simulink model "CONTROL_01"  (R2018b)
(part 101 of 185)

[(de6*((I6xy*(cos(e2)*cos(e3)*sin(e4)*sin(e6) + cos(e2)*cos(e6)*sin(e3)*sin(e5) + cos(e3)*cos(e6)*sin(e2)*sin(e5) - sin(e2)*sin(e3)*sin(e4)*sin(e6) - cos(e2)*cos(e3)*cos(e4)*cos(e5)*cos(e6) + cos(e4)*cos(e5)*cos(e6)*sin(e2)*sin(e3)) + I6yy*(cos(e6)*sin(e2)*sin(e3)*sin(e4) - cos(e2)*cos(e3)*cos(e6)*sin(e4) + cos(e2)*sin(e3)*sin(e5)*sin(e6) + cos(e3)*sin(e2)*sin(e5)*sin(e6) - cos(e2)*cos(e3)*cos(e4)*cos(e5)*sin(e6) + cos(e4)*cos(e5)*sin(e2)*sin(e3)*sin(e6)) + I6yz*(cos(e2)*cos(e5)*sin(e3) + cos(e3)*cos(e5)*sin(e2) + cos(e2)*cos(e3)*cos(e4)*sin(e5) - cos(e4)*sin(e2)*sin(e3)*sin(e5)))*(cos(e2)*cos(e3)*sin(e4)*sin(e6) + cos(e2)*cos(e6)*sin(e3)*sin(e5) + cos(e3)*cos(e6)*sin(e2)*sin(e5) - sin(e2)*sin(e3)*sin(e4)*sin(e6) - cos(e2)*cos(e3)*cos(e4)*cos(e5)*cos(e6) + cos(e4)*cos(e5)*cos(e6)*sin(e2)*sin(e3)) - (I6xx*(cos(e2)*cos(e3)*sin(e4)*sin(e6) + cos(e2)*cos(e6)*sin(e3)*sin(e5) + cos(e3)*cos(e6)*sin(e2)*sin(e5) - sin(e2)*sin(e3)*sin(e4)*sin(e6) - cos(e2)*cos(e3)*cos(e4)*cos(e5)*cos(e6) + cos(e4)*cos(e5)*cos(e6)*sin(e2)*sin(e3)) + I6xy*(cos(e6)*sin(e2)*sin(e3)*sin(e4) - cos(e2)*cos(e3)*cos(e6)*sin(e4) + cos(e2)*sin(e3)*sin(e5)*sin(e6) + cos(e3)*sin(e2)*sin(e5)*sin(e6) - cos(e2)*cos(e3)*cos(e4)*cos(e5)*sin(e6) + cos(e4)*cos(e5)*sin(e2)*sin(e3)*sin(e6)) - I6zx*(cos(e2)*cos(e5)*sin(e3) + cos(e3)*cos(e5)*sin(e2) + cos(e2)*cos(e3)*cos(e4)*sin(e5) - cos(e4)*sin(e2)*sin(e3)*sin(e5)))*(cos(e6)*sin(e2)*sin(e3)*sin(e4) - cos(e2)*cos(e3)*cos(e6)*sin(e4) + cos(e2)*sin(e3)*sin(e5)*sin(e6) + cos(e3)*sin(e2)*sin(e5)*sin(e6) - cos(e2)*cos(e3)*cos(e4)*cos(e5)*sin(e6) + cos(e4)*cos(e5)*sin(e2)*sin(e3)*sin(e6)) + (I6xy*(cos(e2)*cos(e3)*sin(e4)*sin(e6) + cos(e2)*cos(e6)*sin(e3)*sin(e5) + cos(e3)*cos(e6)*sin(e2)*sin(e5) - sin(e2)*sin(e3)*sin(e4)*sin(e6) - cos(e2)*cos(e3)*cos(e4)*cos(e5)*cos(e6) + cos(e4)*cos(e5)*cos(e6)*sin(e2)*sin(e3)) - I6xx*(cos(e6)*sin(e2)*sin(e3)*sin(e4) - cos(e2)*cos(e3)*cos(e6)*sin(e4) + cos(e2)*sin(e3)*sin(e5)*sin(e6) + cos(e3)*sin(e2)*sin(e5)*sin(e6) - cos(e2)*cos(e3)*cos(e4)*cos(e5)*sin(e6) + cos(e4)*cos(e5)*sin(e2)*sin(e3)*sin(e6)))*(cos(e2)*cos(e3)*sin(e4)*sin(e6) + cos(e2)*cos(e6)*sin(e3)*sin(e5) + cos(e3)*cos(e6)*sin(e2)*sin(e5) - sin(e2)*sin(e3)*sin(e4)*sin(e6) - cos(e2)*cos(e3)*cos(e4)*cos(e5)*cos(e6) + cos(e4)*cos(e5)*cos(e6)*sin(e2)*sin(e3)) + (I6yy*(cos(e2)*cos(e3)*sin(e4)*sin(e6) + cos(e2)*cos(e6)*sin(e3)*sin(e5) + cos(e3)*cos(e6)*sin(e2)*sin(e5) - sin(e2)*sin(e3)*sin(e4)*sin(e6) - cos(e2)*cos(e3)*cos(e4)*cos(e5)*cos(e6) + cos(e4)*cos(e5)*cos(e6)*sin(e2)*sin(e3)) - I6xy*(cos(e6)*sin(e2)*sin(e3)*sin(e4) - cos(e2)*cos(e3)*cos(e6)*sin(e4) + cos(e2)*sin(e3)*sin(e5)*sin(e6) + cos(e3)*sin(e2)*sin(e5)*sin(e6) - cos(e2)*cos(e3)*cos(e4)*cos(e5)*sin(e6) + cos(e4)*cos(e5)*sin(e2)*sin(e3)*sin(e6)))*(cos(e6)*sin(e2)*sin(e3)*sin(e4) - cos(e2)*cos(e3)*cos(e6)*sin(e4) + cos(e2)*sin(e3)*sin(e5)*sin(e6) + cos(e3)*sin(e2)*sin(e5)*sin(e6) - cos(e2)*cos(e3)*cos(e4)*cos(e5)*sin(e6) + cos(e4)*cos(e5)*sin(e2)*sin(e3)*sin(e6)) + (I6yz*(cos(e2)*cos(e3)*sin(e4)*sin(e6) + cos(e2)*cos(e6)*sin(e3)*sin(e5) + cos(e3)*cos(e6)*sin(e2)*sin(e5) - sin(e2)*sin(e3)*sin(e4)*sin(e6) - cos(e2)*cos(e3)*cos(e4)*cos(e5)*cos(e6) + cos(e4)*cos(e5)*cos(e6)*sin(e2)*sin(e3)) + I6zx*(cos(e6)*sin(e2)*sin(e3)*sin(e4) - cos(e2)*cos(e3)*cos(e6)*sin(e4) + cos(e2)*sin(e3)*sin(e5)*sin(e6) + cos(e3)*sin(e2)*sin(e5)*sin(e6) - cos(e2)*cos(e3)*cos(e4)*cos(e5)*sin(e6) + cos(e4)*cos(e5)*sin(e2)*sin(e3)*sin(e6)))*(cos(e2)*cos(e5)*sin(e3) + cos(e3)*cos(e5)*sin(e2) + cos(e2)*cos(e3)*cos(e4)*sin(e5) - cos(e4)*sin(e2)*sin(e3)*sin(e5)) + 2*m6*(x6*(cos(e6)*(cos(e4)*sin(e1) - sin(e2 + e3)*cos(e1)*sin(e4)) - sin(e6)*(cos(e5)*(sin(e1)*sin(e4) + sin(e2 + e3)*cos(e1)*cos(e4)) + cos(e2 + e3)*cos(e1)*sin(e5))) - y6*(sin(e6)*(cos(e4)*sin(e1) - sin(e2 + e3)*cos(e1)*sin(e4)) + cos(e6)*(cos(e5)*(sin(e1)*sin(e4) + sin(e2 + e3)*cos(e1)*cos(e4)) + cos(e2 + e3)*cos(e1)*sin(e5))))*(cos(e1)*(a1 + d4*cos(e2 + e3) + a3*sin(e2 + e3) + a2*sin(e2)) + x6*(sin(e6)*(cos(e4)*sin(e1) - sin(e2 + e3)*cos(e1)*sin(e4)) + cos(e6)*(cos(e5)*(sin(e1)*sin(e4) + sin(e2 + e3)*cos(e1)*cos(e4)) + cos(e2 + e3)*cos(e1)*sin(e5))) + y6*(cos(e6)*(cos(e4)*sin(e1) - sin(e2 + e3)*cos(e1)*sin(e4)) - sin(e6)*(cos(e5)*(sin(e1)*sin(e4) + sin(e2 + e3)*cos(e1)*cos(e4)) + cos(e2 + e3)*cos(e1)*sin(e5))) - z6*(sin(e5)*(sin(e1)*sin(e4) + sin(e2 + e3)*cos(e1)*cos(e4)) - cos(e2 + e3)*cos(e1)*cos(e5))) - 2*m6*(x6*(cos(e6)*(cos(e1)*cos(e4) + sin(e2 + e3)*sin(e1)*sin(e4)) - sin(e6)*(cos(e5)*(cos(e1)*sin(e4) - sin(e2 + e3)*cos(e4)*sin(e1)) - cos(e2 + e3)*sin(e1)*sin(e5))) - y6*(sin(e6)*(cos(e1)*cos(e4) + sin(e2 + e3)*sin(e1)*sin(e4)) + cos(e6)*(cos(e5)*(cos(e1)*sin(e4) - sin(e2 + e3)*cos(e4)*sin(e1)) - cos(e2 + e3)*sin(e1)*sin(e5))))*(sin(e1)*(a1 + d4*cos(e2 + e3) + a3*sin(e2 + e3) + a2*sin(e2)) - x6*(sin(e6)*(cos(e1)*cos(e4) + sin(e2 + e3)*sin(e1)*sin(e4)) + cos(e6)*(cos(e5)*(cos(e1)*sin(e4) - sin(e2 + e3)*cos(e4)*sin(e1)) - cos(e2 + e3)*sin(e1)*sin(e5))) - y6*(cos(e6)*(cos(e1)*cos(e4) + sin(e2 + e3)*sin(e1)*sin(e4)) - sin(e6)*(cos(e5)*(cos(e1)*sin(e4) - sin(e2 + e3)*cos(e4)*sin(e1)) - cos(e2 + e3)*sin(e1)*sin(e5))) + z6*(sin(e5)*(cos(e1)*sin(e4) - sin(e2 + e3)*cos(e4)*sin(e1)) + cos(e2 + e3)*cos(e5)*sin(e1)))))/2 + (de3*((I6xx*(cos(e2)*cos(e3)*cos(e6)*sin(e5) - cos(e2)*sin(e3)*sin(e4)*sin(e6) - cos(e3)*sin(e2)*sin(e4)*sin(e6) - cos(e6)*sin(e2)*sin(e3)*sin(e5) + cos(e2)*cos(e4)*cos(e5)*cos(e6)*sin(e3) + cos(e3)*cos(e4)*cos(e5)*cos(e6)*sin(e2)) + I6xy*(cos(e2)*cos(e6)*sin(e3)*sin(e4) + cos(e3)*cos(e6)*sin(e2)*sin(e4) + cos(e2)*cos(e3)*sin(e5)*sin(e6) - sin(e2)*sin(e3)*sin(e5)*sin(e6) + cos(e2)*cos(e4)*cos(e5)*sin(e3)*sin(e6) + cos(e3)*cos(e4)*cos(e5)*sin(e2)*sin(e6)) + I6zx*(cos(e5)*sin(e2)*sin(e3) - cos(e2)*cos(e3)*cos(e5) + cos(e2)*cos(e4)*sin(e3)*sin(e5) + cos(e3)*cos(e4)*sin(e2)*sin(e5)))*(cos(e2)*cos(e3)*sin(e4)*sin(e6) + cos(e2)*cos(e6)*sin(e3)*sin(e5) + cos(e3)*cos(e6)*sin(e2)*sin(e5) - sin(e2)*sin(e3)*sin(e4)*sin(e6) - cos(e2)*cos(e3)*cos(e4)*cos(e5)*cos(e6) + cos(e4)*cos(e5)*cos(e6)*sin(e2)*sin(e3)) + (I6xx*(cos(e2)*cos(e3)*sin(e4)*sin(e6) + cos(e2)*cos(e6)*sin(e3)*sin(e5) + cos(e3)*cos(e6)*sin(e2)*sin(e5) - sin(e2)*sin(e3)*sin(e4)*sin(e6) - cos(e2)*cos(e3)*cos(e4)*cos(e5)*cos(e6) + cos(e4)*cos(e5)*cos(e6)*sin(e2)*sin(e3)) + I6xy*(cos(e6)*sin(e2)*sin(e3)*sin(e4) - cos(e2)*cos(e3)*cos(e6)*sin(e4) + cos(e2)*sin(e3)*sin(e5)*sin(e6) + cos(e3)*sin(e2)*sin(e5)*sin(e6) - cos(e2)*cos(e3)*cos(e4)*cos(e5)*sin(e6) + cos(e4)*cos(e5)*sin(e2)*sin(e3)*sin(e6)) - I6zx*(cos(e2)*cos(e5)*sin(e3) + cos(e3)*cos(e5)*sin(e2) + cos(e2)*cos(e3)*cos(e4)*sin(e5) - cos(e4)*sin(e2)*sin(e3)*sin(e5)))*(cos(e2)*cos(e3)*cos(e6)*sin(e5) - cos(e2)*sin(e3)*sin(e4)*sin(e6) - cos(e3)*sin(e2)*sin(e4)*sin(e6) - cos(e6)*sin(e2)*sin(e3)*sin(e5) + cos(e2)*cos(e4)*cos(e5)*cos(e6)*sin(e3) + cos(e3)*cos(e4)*cos(e5)*cos(e6)*sin(e2)) - (cos(e2)*cos(e3)*cos(e4) - cos(e4)*sin(e2)*sin(e3))*(I4xx*(cos(e2)*cos(e4)*sin(e3) + cos(e3)*cos(e4)*sin(e2)) - I4zx*cos(e2 + e3) + I4xy*(cos(e2)*sin(e3)*sin(e4) + cos(e3)*sin(e2)*sin(e4))) - (cos(e2)*sin(e3)*sin(e4) + cos(e3)*sin(e2)*sin(e4))*(I5zz*(cos(e2)*cos(e3)*sin(e4) - sin(e2)*sin(e3)*sin(e4)) + I5yz*(cos(e2)*cos(e5)*sin(e3) + cos(e3)*cos(e5)*sin(e2) + cos(e2)*cos(e3)*cos(e4)*sin(e5) - cos(e4)*sin(e2)*sin(e3)*sin(e5)) + I5zx*(cos(e2)*sin(e3)*sin(e5) + cos(e3)*sin(e2)*sin(e5) - cos(e2)*cos(e3)*cos(e4)*cos(e5) + cos(e4)*cos(e5)*sin(e2)*sin(e3))) - (cos(e2)*cos(e3)*sin(e4) - sin(e2)*sin(e3)*sin(e4))*(I5zz*(cos(e2)*sin(e3)*sin(e4) + cos(e3)*sin(e2)*sin(e4)) + I5yz*(cos(e5)*sin(e2)*sin(e3) - cos(e2)*cos(e3)*cos(e5) + cos(e2)*cos(e4)*sin(e3)*sin(e5) + cos(e3)*cos(e4)*sin(e2)*sin(e5)) - I5zx*(cos(e2)*cos(e3)*sin(e5) - sin(e2)*sin(e3)*sin(e5) + cos(e2)*cos(e4)*cos(e5)*sin(e3) + cos(e3)*cos(e4)*cos(e5)*sin(e2))) - (cos(e2)*cos(e4)*sin(e3) + cos(e3)*cos(e4)*sin(e2))*(I4zx*sin(e2 + e3) + I4xx*(cos(e2)*cos(e3)*cos(e4) - cos(e4)*sin(e2)*sin(e3)) + I4xy*(cos(e2)*cos(e3)*sin(e4) - sin(e2)*sin(e3)*sin(e4))) + (I6xy*(cos(e2)*cos(e3)*sin(e4)*sin(e6) + cos(e2)*cos(e6)*sin(e3)*sin(e5) + cos(e3)*cos(e6)*sin(e2)*sin(e5) - sin(e2)*sin(e3)*sin(e4)*sin(e6) - cos(e2)*cos(e3)*cos(e4)*cos(e5)*cos(e6) + cos(e4)*cos(e5)*cos(e6)*sin(e2)*sin(e3)) + I6yy*(cos(e6)*sin(e2)*sin(e3)*sin(e4) - cos(e2)*cos(e3)*cos(e6)*sin(e4) + cos(e2)*sin(e3)*sin(e5)*sin(e6) + cos(e3)*sin(e2)*sin(e5)*sin(e6) - cos(e2)*cos(e3)*cos(e4)*cos(e5)*sin(e6) + cos(e4)*cos(e5)*sin(e2)*sin(e3)*sin(e6)) + I6yz*(cos(e2)*cos(e5)*sin(e3) + cos(e3)*cos(e5)*sin(e2) + cos(e2)*cos(e3)*cos(e4)*sin(e5) - cos(e4)*sin(e2)*sin(e3)*sin(e5)))*(cos(e2)*cos(e6)*sin(e3)*sin(e4) + cos(e3)*cos(e6)*sin(e2)*sin(e4) + cos(e2)*cos(e3)*sin(e5)*sin(e6) - sin(e2)*sin(e3)*sin(e5)*sin(e6) + cos(e2)*cos(e4)*cos(e5)*sin(e3)*sin(e6) + cos(e3)*cos(e4)*cos(e5)*sin(e2)*sin(e6)) + (I6xy*(cos(e2)*cos(e3)*cos(e6)*sin(e5) - cos(e2)*sin(e3)*sin(e4)*sin(e6) - cos(e3)*sin(e2)*sin(e4)*sin(e6) - cos(e6)*sin(e2)*sin(e3)*sin(e5) + cos(e2)*cos(e4)*cos(e5)*cos(e6)*sin(e3) + cos(e3)*cos(e4)*cos(e5)*cos(e6)*sin(e2)) + I6yy*(cos(e2)*cos(e6)*sin(e3)*sin(e4) + cos(e3)*cos(e6)*sin(e2)*sin(e4) + cos(e2)*cos(e3)*sin(e5)*sin(e6) - sin(e2)*sin(e3)*sin(e5)*sin(e6) + cos(e2)*cos(e4)*cos(e5)*sin(e3)*sin(e6) + cos(e3)*cos(e4)*cos(e5)*sin(e2)*sin(e6)) - I6yz*(cos(e5)*sin(e2)*sin(e3) - cos(e2)*cos(e3)*cos(e5) + cos(e2)*cos(e4)*sin(e3)*sin(e5) + cos(e3)*cos(e4)*sin(e2)*sin(e5)))*(cos(e6)*sin(e2)*sin(e3)*sin(e4) - cos(e2)*cos(e3)*cos(e6)*sin(e4) + cos(e2)*sin(e3)*sin(e5)*sin(e6) + cos(e3)*sin(e2)*sin(e5)*sin(e6) - cos(e2)*cos(e3)*cos(e4)*cos(e5)*sin(e6) + cos(e4)*cos(e5)*sin(e2)*sin(e3)*sin(e6)) - (cos(e2)*cos(e3)*sin(e4) - sin(e2)*sin(e3)*sin(e4))*(I4yz*cos(e2 + e3) + I4xy*(cos(e2)*cos(e4)*sin(e3) + cos(e3)*cos(e4)*sin(e2)) + I4yy*(cos(e2)*sin(e3)*sin(e4) + cos(e3)*sin(e2)*sin(e4))) + (I5xx*(cos(e2)*cos(e3)*sin(e5) - sin(e2)*sin(e3)*sin(e5) + cos(e2)*cos(e4)*cos(e5)*sin(e3) + cos(e3)*cos(e4)*cos(e5)*sin(e2)) - I5zx*(cos(e2)*sin(e3)*sin(e4) + cos(e3)*sin(e2)*sin(e4)) + I5xy*(cos(e5)*sin(e2)*sin(e3) - cos(e2)*cos(e3)*cos(e5) + cos(e2)*cos(e4)*sin(e3)*sin(e5) + cos(e3)*cos(e4)*sin(e2)*sin(e5)))*(cos(e2)*sin(e3)*sin(e5) + cos(e3)*sin(e2)*sin(e5) - cos(e2)*cos(e3)*cos(e4)*cos(e5) + cos(e4)*cos(e5)*sin(e2)*sin(e3)) + (I5zx*(cos(e2)*cos(e3)*sin(e4) - sin(e2)*sin(e3)*sin(e4)) + I5xx*(cos(e2)*sin(e3)*sin(e5) + cos(e3)*sin(e2)*sin(e5) - cos(e2)*cos(e3)*cos(e4)*cos(e5) + cos(e4)*cos(e5)*sin(e2)*sin(e3)) - I5xy*(cos(e2)*cos(e5)*sin(e3) + cos(e3)*cos(e5)*sin(e2) + cos(e2)*cos(e3)*cos(e4)*sin(e5) - cos(e4)*sin(e2)*sin(e3)*sin(e5)))*(cos(e2)*cos(e3)*sin(e5) - sin(e2)*sin(e3)*sin(e5) + cos(e2)*cos(e4)*cos(e5)*sin(e3) + cos(e3)*cos(e4)*cos(e5)*sin(e2)) - (I5yz*(cos(e2)*sin(e3)*sin(e4) + cos(e3)*sin(e2)*sin(e4)) + I5xy*(cos(e2)*cos(e3)*sin(e5) - sin(e2)*sin(e3)*sin(e5) + cos(e2)*cos(e4)*cos(e5)*sin(e3) + cos(e3)*cos(e4)*cos(e5)*sin(e2)) + I5yy*(cos(e5)*sin(e2)*sin(e3) - cos(e2)*cos(e3)*cos(e5) + cos(e2)*cos(e4)*sin(e3)*sin(e5) + cos(e3)*cos(e4)*sin(e2)*sin(e5)))*(cos(e2)*cos(e5)*sin(e3) + cos(e3)*cos(e5)*sin(e2) + cos(e2)*cos(e3)*cos(e4)*sin(e5) - cos(e4)*sin(e2)*sin(e3)*sin(e5)) - (I5yz*(cos(e2)*cos(e3)*sin(e4) - sin(e2)*sin(e3)*sin(e4)) - I5xy*(cos(e2)*sin(e3)*sin(e5) + cos(e3)*sin(e2)*sin(e5) - cos(e2)*cos(e3)*cos(e4)*cos(e5) + cos(e4)*cos(e5)*sin(e2)*sin(e3)) + I5yy*(cos(e2)*cos(e5)*sin(e3) + cos(e3)*cos(e5)*sin(e2) + cos(e2)*cos(e3)*cos(e4)*sin(e5) - cos(e4)*sin(e2)*sin(e3)*sin(e5)))*(cos(e5)*sin(e2)*sin(e3) - cos(e2)*cos(e3)*cos(e5) + cos(e2)*cos(e4)*sin(e3)*sin(e5) + cos(e3)*cos(e4)*sin(e2)*sin(e5)) - (cos(e2)*sin(e3)*sin(e4) + cos(e3)*sin(e2)*sin(e4))*(I4xy*(cos(e2)*cos(e3)*cos(e4) - cos(e4)*sin(e2)*sin(e3)) - I4yz*sin(e2 + e3) + I4yy*(cos(e2)*cos(e3)*sin(e4) - sin(e2)*sin(e3)*sin(e4))) - (I6zx*(cos(e2)*cos(e3)*cos(e6)*sin(e5) - cos(e2)*sin(e3)*sin(e4)*sin(e6) - cos(e3)*sin(e2)*sin(e4)*sin(e6) - cos(e6)*sin(e2)*sin(e3)*sin(e5) + cos(e2)*cos(e4)*cos(e5)*cos(e6)*sin(e3) + cos(e3)*cos(e4)*cos(e5)*cos(e6)*sin(e2)) - I6yz*(cos(e2)*cos(e6)*sin(e3)*sin(e4) + cos(e3)*cos(e6)*sin(e2)*sin(e4) + cos(e2)*cos(e3)*sin(e5)*sin(e6) - sin(e2)*sin(e3)*sin(e5)*sin(e6) + cos(e2)*cos(e4)*cos(e5)*sin(e3)*sin(e6) + cos(e3)*cos(e4)*cos(e5)*sin(e2)*sin(e6)) + I6zz*(cos(e5)*sin(e2)*sin(e3) - cos(e2)*cos(e3)*cos(e5) + cos(e2)*cos(e4)*sin(e3)*sin(e5) + cos(e3)*cos(e4)*sin(e2)*sin(e5)))*(cos(e2)*cos(e5)*sin(e3) + cos(e3)*cos(e5)*sin(e2) + cos(e2)*cos(e3)*cos(e4)*sin(e5) - cos(e4)*sin(e2)*sin(e3)*sin(e5)) - (I6yz*(cos(e6)*sin(e2)*sin(e3)*sin(e4) - cos(e2)*cos(e3)*cos(e6)*sin(e4) + cos(e2)*sin(e3)*sin(e5)*sin(e6) + cos(e3)*sin(e2)*sin(e5)*sin(e6) - cos(e2)*cos(e3)*cos(e4)*cos(e5)*sin(e6) + cos(e4)*cos(e5)*sin(e2)*sin(e3)*sin(e6)) - I6zx*(cos(e2)*cos(e3)*sin(e4)*sin(e6) + cos(e2)*cos(e6)*sin(e3)*sin(e5) + cos(e3)*cos(e6)*sin(e2)*sin(e5) - sin(e2)*sin(e3)*sin(e4)*sin(e6) - cos(e2)*cos(e3)*cos(e4)*cos(e5)*cos(e6) + cos(e4)*cos(e5)*cos(e6)*sin(e2)*sin(e3)) + I6zz*(cos(e2)*cos(e5)*sin(e3) + cos(e3)*cos(e5)*sin(e2) + cos(e2)*cos(e3)*cos(e4)*sin(e5) - cos(e4)*sin(e2)*sin(e3)*sin(e5)))*(cos(e5)*sin(e2)*sin(e3) - cos(e2)*cos(e3)*cos(e5) + cos(e2)*cos(e4)*sin(e3)*sin(e5) + cos(e3)*cos(e4)*sin(e2)*sin(e5)) + cos(e2 + e3)*(I3xy*cos(e2 + e3) - I3xx*sin(e2 + e3)) + cos(e2 + e3)*(I3xy*cos(e2 + e3) + I3yy*sin(e2 + e3)) - sin(e2 + e3)*(I3xx*cos(e2 + e3) + I3xy*sin(e2 + e3)) + sin(e2 + e3)*(I3yy*cos(e2 + e3) - I3xy*sin(e2 + e3)) + sin(e2 + e3)*(I4zz*cos(e2 + e3) - I4zx*(cos(e2)*cos(e4)*sin(e3) + cos(e3)*cos(e4)*sin(e2)) + I4yz*(cos(e2)*sin(e3)*sin(e4) + cos(e3)*sin(e2)*sin(e4))) + cos(e2 + e3)*(I4zz*sin(e2 + e3) + I4zx*(cos(e2)*cos(e3)*cos(e4) - cos(e4)*sin(e2)*sin(e3)) - I4yz*(cos(e2)*cos(e3)*sin(e4) - sin(e2)*sin(e3)*sin(e4))) + 2*m4*(cos(e1)*(a1 + d4*cos(e2 + e3) + a3*sin(e2 + e3) + a2*sin(e2)) + x4*(sin(e1)*sin(e4) + sin(e2 + e3)*cos(e1)*cos(e4)) + y4*(cos(e4)*sin(e1) - sin(e2 + e3)*cos(e1)*sin(e4)) + z4*cos(e2 + e3)*cos(e1))*(cos(e1)*(a3*cos(e2 + e3) - d4*sin(e2 + e3)) - z4*sin(e2 + e3)*cos(e1) - y4*cos(e2 + e3)*cos(e1)*sin(e4) + x4*cos(e2 + e3)*cos(e1)*cos(e4)) - 2*m6*(sin(e1)*(a1 + d4*cos(e2 + e3) + a3*sin(e2 + e3) + a2*sin(e2)) - x6*(sin(e6)*(cos(e1)*cos(e4) + sin(e2 + e3)*sin(e1)*sin(e4)) + cos(e6)*(cos(e5)*(cos(e1)*sin(e4) - sin(e2 + e3)*cos(e4)*sin(e1)) - cos(e2 + e3)*sin(e1)*sin(e5))) - y6*(cos(e6)*(cos(e1)*cos(e4) + sin(e2 + e3)*sin(e1)*sin(e4)) - sin(e6)*(cos(e5)*(cos(e1)*sin(e4) - sin(e2 + e3)*cos(e4)*sin(e1)) - cos(e2 + e3)*sin(e1)*sin(e5))) + z6*(sin(e5)*(cos(e1)*sin(e4) - sin(e2 + e3)*cos(e4)*sin(e1)) + cos(e2 + e3)*cos(e5)*sin(e1)))*(x6*(cos(e6)*(sin(e2 + e3)*sin(e1)*sin(e5) - cos(e2 + e3)*cos(e4)*cos(e5)*sin(e1)) + cos(e2 + e3)*sin(e1)*sin(e4)*sin(e6)) - y6*(sin(e6)*(sin(e2 + e3)*sin(e1)*sin(e5) - cos(e2 + e3)*cos(e4)*cos(e5)*sin(e1)) - cos(e2 + e3)*cos(e6)*sin(e1)*sin(e4)) + z6*(sin(e2 + e3)*cos(e5)*sin(e1) + cos(e2 + e3)*cos(e4)*sin(e1)*sin(e5)) - sin(e1)*(a3*cos(e2 + e3) - d4*sin(e2 + e3))) - 2*m6*(x6*(cos(e6)*(sin(e2 + e3)*cos(e1)*sin(e5) - cos(e2 + e3)*cos(e1)*cos(e4)*cos(e5)) + cos(e2 + e3)*cos(e1)*sin(e4)*sin(e6)) - y6*(sin(e6)*(sin(e2 + e3)*cos(e1)*sin(e5) - cos(e2 + e3)*cos(e1)*cos(e4)*cos(e5)) - cos(e2 + e3)*cos(e1)*cos(e6)*sin(e4)) + z6*(sin(e2 + e3)*cos(e1)*cos(e5) + cos(e2 + e3)*cos(e1)*cos(e4)*sin(e5)) - cos(e1)*(a3*cos(e2 + e3) - d4*sin(e2 + e3)))*(cos(e1)*(a1 + d4*cos(e2 + e3) + a3*sin(e2 + e3) + a2*sin(e2)) + x6*(sin(e6)*(cos(e4)*sin(e1) - sin(e2 + e3)*cos(e1)*sin(e4)) + cos(e6)*(cos(e5)*(sin(e1)*sin(e4) + sin(e2 + e3)*cos(e1)*cos(e4)) + cos(e2 + e3)*cos(e1)*sin(e5))) + y6*(cos(e6)*(cos(e4)*sin(e1) - sin(e2 + e3)*cos(e1)*sin(e4)) - sin(e6)*(cos(e5)*(sin(e1)*sin(e4) + sin(e2 + e3)*cos(e1)*cos(e4)) + cos(e2 + e3)*cos(e1)*sin(e5))) - z6*(sin(e5)*(sin(e1)*sin(e4) + sin(e2 + e3)*cos(e1)*cos(e4)) - cos(e2 + e3)*cos(e1)*cos(e5))) + 2*m4*(sin(e1)*(a3*cos(e2 + e3) - d4*sin(e2 + e3)) - z4*sin(e2 + e3)*sin(e1) + x4*cos(e2 + e3)*cos(e4)*sin(e1) - y4*cos(e2 + e3)*sin(e1)*sin(e4))*(sin(e1)*(a1 + d4*cos(e2 + e3) + a3*sin(e2 + e3) + a2*sin(e2)) - x4*(cos(e1)*sin(e4) - sin(e2 + e3)*cos(e4)*sin(e1)) - y4*(cos(e1)*cos(e4) + sin(e2 + e3)*sin(e1)*sin(e4)) + z4*cos(e2 + e3)*sin(e1)) - 2*m5*(x5*(sin(e2 + e3)*sin(e1)*sin(e5) - cos(e2 + e3)*cos(e4)*cos(e5)*sin(e1)) + y5*(sin(e2 + e3)*cos(e5)*sin(e1) + cos(e2 + e3)*cos(e4)*sin(e1)*sin(e5)) - sin(e1)*(a3*cos(e2 + e3) - d4*sin(e2 + e3)) - z5*cos(e2 + e3)*sin(e1)*sin(e4))*(sin(e1)*(a1 + d4*cos(e2 + e3) + a3*sin(e2 + e3) + a2*sin(e2)) + z5*(cos(e1)*cos(e4) + sin(e2 + e3)*sin(e1)*sin(e4)) - x5*(cos(e5)*(cos(e1)*sin(e4) - sin(e2 + e3)*cos(e4)*sin(e1)) - cos(e2 + e3)*sin(e1)*sin(e5)) + y5*(sin(e5)*(cos(e1)*sin(e4) - sin(e2 + e3)*cos(e4)*sin(e1)) + cos(e2 + e3)*cos(e5)*sin(e1))) + 2*m3*(x3*cos(e2 + e3)*cos(e1) - y3*sin(e2 + e3)*cos(e1))*(cos(e1)*(a1 + a2*sin(e2)) - z3*sin(e1) + y3*cos(e2 + e3)*cos(e1) + x3*sin(e2 + e3)*cos(e1)) - 2*m5*(cos(e1)*(a1 + d4*cos(e2 + e3) + a3*sin(e2 + e3) + a2*sin(e2)) - z5*(cos(e4)*sin(e1) - sin(e2 + e3)*cos(e1)*sin(e4)) + x5*(cos(e5)*(sin(e1)*sin(e4) + sin(e2 + e3)*cos(e1)*cos(e4)) + cos(e2 + e3)*cos(e1)*sin(e5)) - y5*(sin(e5)*(sin(e1)*sin(e4) + sin(e2 + e3)*cos(e1)*cos(e4)) - cos(e2 + e3)*cos(e1)*cos(e5)))*(x5*(sin(e2 + e3)*cos(e1)*sin(e5) - cos(e2 + e3)*cos(e1)*cos(e4)*cos(e5)) + y5*(sin(e2 + e3)*cos(e1)*cos(e5) + cos(e2 + e3)*cos(e1)*cos(e4)*sin(e5)) - cos(e1)*(a3*cos(e2 + e3) - d4*sin(e2 + e3)) - z5*cos(e2 + e3)*cos(e1)*sin(e4)) + 2*m3*(x3*cos(e2 + e3)*sin(e1) - y3*sin(e2 + e3)*sin(e1))*(sin(e1)*(a1 + a2*sin(e2)) + z3*cos(e1) + y3*cos(e2 + e3)*sin(e1) + x3*sin(e2 + e3)*sin(e1))))/2 + (de5*((I6xy*(cos(e2)*cos(e3)*sin(e4)*sin(e6) + cos(e2)*cos(e6)*sin(e3)*sin(e5) + cos(e3)*cos(e6)*sin(e2)*sin(e5) - sin(e2)*sin(e3)*sin(e4)*sin(e6) - cos(e2)*cos(e3)*cos(e4)*cos(e5)*cos(e6) + cos(e4)*cos(e5)*cos(e6)*sin(e2)*sin(e3)) + I6yy*(cos(e6)*sin(e2)*sin(e3)*sin(e4) - cos(e2)*cos(e3)*cos(e6)*sin(e4) + cos(e2)*sin(e3)*sin(e5)*sin(e6) + cos(e3)*sin(e2)*sin(e5)*sin(e6) - cos(e2)*cos(e3)*cos(e4)*cos(e5)*sin(e6) + cos(e4)*cos(e5)*sin(e2)*sin(e3)*sin(e6)) + I6yz*(cos(e2)*cos(e5)*sin(e3) + cos(e3)*cos(e5)*sin(e2) + cos(e2)*cos(e3)*cos(e4)*sin(e5) - cos(e4)*sin(e2)*sin(e3)*sin(e5)))*(cos(e2)*cos(e5)*sin(e3)*sin(e6) + cos(e3)*cos(e5)*sin(e2)*sin(e6) + cos(e2)*cos(e3)*cos(e4)*sin(e5)*sin(e6) - cos(e4)*sin(e2)*sin(e3)*sin(e5)*sin(e6)) - (I6zz*(cos(e2)*sin(e3)*sin(e5) + cos(e3)*sin(e2)*sin(e5) - cos(e2)*cos(e3)*cos(e4)*cos(e5) + cos(e4)*cos(e5)*sin(e2)*sin(e3)) - I6yz*(cos(e2)*cos(e5)*sin(e3)*sin(e6) + cos(e3)*cos(e5)*sin(e2)*sin(e6) + cos(e2)*cos(e3)*cos(e4)*sin(e5)*sin(e6) - cos(e4)*sin(e2)*sin(e3)*sin(e5)*sin(e6)) + I6zx*(cos(e2)*cos(e5)*cos(e6)*sin(e3) + cos(e3)*cos(e5)*cos(e6)*sin(e2) + cos(e2)*cos(e3)*cos(e4)*cos(e6)*sin(e5) - cos(e4)*cos(e6)*sin(e2)*sin(e3)*sin(e5)))*(cos(e2)*cos(e5)*sin(e3) + cos(e3)*cos(e5)*sin(e2) + cos(e2)*cos(e3)*cos(e4)*sin(e5) - cos(e4)*sin(e2)*sin(e3)*sin(e5)) + (I5zx*(cos(e2)*cos(e3)*sin(e4) - sin(e2)*sin(e3)*sin(e4)) + I5xx*(cos(e2)*sin(e3)*sin(e5) + cos(e3)*sin(e2)*sin(e5) - cos(e2)*cos(e3)*cos(e4)*cos(e5) + cos(e4)*cos(e5)*sin(e2)*sin(e3)) - I5xy*(cos(e2)*cos(e5)*sin(e3) + cos(e3)*cos(e5)*sin(e2) + cos(e2)*cos(e3)*cos(e4)*sin(e5) - cos(e4)*sin(e2)*sin(e3)*sin(e5)))*(cos(e2)*cos(e5)*sin(e3) + cos(e3)*cos(e5)*sin(e2) + cos(e2)*cos(e3)*cos(e4)*sin(e5) - cos(e4)*sin(e2)*sin(e3)*sin(e5)) - (I5yz*(cos(e2)*cos(e3)*sin(e4) - sin(e2)*sin(e3)*sin(e4)) - I5xy*(cos(e2)*sin(e3)*sin(e5) + cos(e3)*sin(e2)*sin(e5) - cos(e2)*cos(e3)*cos(e4)*cos(e5) + cos(e4)*cos(e5)*sin(e2)*sin(e3)) + I5yy*(cos(e2)*cos(e5)*sin(e3) + cos(e3)*cos(e5)*sin(e2) + cos(e2)*cos(e3)*cos(e4)*sin(e5) - cos(e4)*sin(e2)*sin(e3)*sin(e5)))*(cos(e2)*sin(e3)*sin(e5) + cos(e3)*sin(e2)*sin(e5) - cos(e2)*cos(e3)*cos(e4)*cos(e5) + cos(e4)*cos(e5)*sin(e2)*sin(e3)) - (cos(e2)*cos(e3)*sin(e4) - sin(e2)*sin(e3)*sin(e4))*(I5yz*(cos(e2)*sin(e3)*sin(e5) + cos(e3)*sin(e2)*sin(e5) - cos(e2)*cos(e3)*cos(e4)*cos(e5) + cos(e4)*cos(e5)*sin(e2)*sin(e3)) - I5zx*(cos(e2)*cos(e5)*sin(e3) + cos(e3)*cos(e5)*sin(e2) + cos(e2)*cos(e3)*cos(e4)*sin(e5) - cos(e4)*sin(e2)*sin(e3)*sin(e5))) + (I6xy*(cos(e2)*cos(e5)*sin(e3)*sin(e6) + cos(e3)*cos(e5)*sin(e2)*sin(e6) + cos(e2)*cos(e3)*cos(e4)*sin(e5)*sin(e6) - cos(e4)*sin(e2)*sin(e3)*sin(e5)*sin(e6)) + I6zx*(cos(e2)*sin(e3)*sin(e5) + cos(e3)*sin(e2)*sin(e5) - cos(e2)*cos(e3)*cos(e4)*cos(e5) + cos(e4)*cos(e5)*sin(e2)*sin(e3)) + I6xx*(cos(e2)*cos(e5)*cos(e6)*sin(e3) + cos(e3)*cos(e5)*cos(e6)*sin(e2) + cos(e2)*cos(e3)*cos(e4)*cos(e6)*sin(e5) - cos(e4)*cos(e6)*sin(e2)*sin(e3)*sin(e5)))*(cos(e2)*cos(e3)*sin(e4)*sin(e6) + cos(e2)*cos(e6)*sin(e3)*sin(e5) + cos(e3)*cos(e6)*sin(e2)*sin(e5) - sin(e2)*sin(e3)*sin(e4)*sin(e6) - cos(e2)*cos(e3)*cos(e4)*cos(e5)*cos(e6) + cos(e4)*cos(e5)*cos(e6)*sin(e2)*sin(e3)) + (I5xx*(cos(e2)*cos(e5)*sin(e3) + cos(e3)*cos(e5)*sin(e2) + cos(e2)*cos(e3)*cos(e4)*sin(e5) - cos(e4)*sin(e2)*sin(e3)*sin(e5)) + I5xy*(cos(e2)*sin(e3)*sin(e5) + cos(e3)*sin(e2)*sin(e5) - cos(e2)*cos(e3)*cos(e4)*cos(e5) + cos(e4)*cos(e5)*sin(e2)*sin(e3)))*(cos(e2)*sin(e3)*sin(e5) + cos(e3)*sin(e2)*sin(e5) - cos(e2)*cos(e3)*cos(e4)*cos(e5) + cos(e4)*cos(e5)*sin(e2)*sin(e3)) - (I5xy*(cos(e2)*cos(e5)*sin(e3) + cos(e3)*cos(e5)*sin(e2) + cos(e2)*cos(e3)*cos(e4)*sin(e5) - cos(e4)*sin(e2)*sin(e3)*sin(e5)) + I5yy*(cos(e2)*sin(e3)*sin(e5) + cos(e3)*sin(e2)*sin(e5) - cos(e2)*cos(e3)*cos(e4)*cos(e5) + cos(e4)*cos(e5)*sin(e2)*sin(e3)))*(cos(e2)*cos(e5)*sin(e3) + cos(e3)*cos(e5)*sin(e2) + cos(e2)*cos(e3)*cos(e4)*sin(e5) - cos(e4)*sin(e2)*sin(e3)*sin(e5)) + (I6yy*(cos(e2)*cos(e5)*sin(e3)*sin(e6) + cos(e3)*cos(e5)*sin(e2)*sin(e6) + cos(e2)*cos(e3)*cos(e4)*sin(e5)*sin(e6) - cos(e4)*sin(e2)*sin(e3)*sin(e5)*sin(e6)) - I6yz*(cos(e2)*sin(e3)*sin(e5) + cos(e3)*sin(e2)*sin(e5) - cos(e2)*cos(e3)*cos(e4)*cos(e5) + cos(e4)*cos(e5)*sin(e2)*sin(e3)) + I6xy*(cos(e2)*cos(e5)*cos(e6)*sin(e3) + cos(e3)*cos(e5)*cos(e6)*sin(e2) + cos(e2)*cos(e3)*cos(e4)*cos(e6)*sin(e5) - cos(e4)*cos(e6)*sin(e2)*sin(e3)*sin(e5)))*(cos(e6)*sin(e2)*sin(e3)*sin(e4) - cos(e2)*cos(e3)*cos(e6)*sin(e4) + cos(e2)*sin(e3)*sin(e5)*sin(e6) + cos(e3)*sin(e2)*sin(e5)*sin(e6) - cos(e2)*cos(e3)*cos(e4)*cos(e5)*sin(e6) + cos(e4)*cos(e5)*sin(e2)*sin(e3)*sin(e6)) - (I6yz*(cos(e6)*sin(e2)*sin(e3)*sin(e4) - cos(e2)*cos(e3)*cos(e6)*sin(e4) + cos(e2)*sin(e3)*sin(e5)*sin(e6) + cos(e3)*sin(e2)*sin(e5)*sin(e6) - cos(e2)*cos(e3)*cos(e4)*cos(e5)*sin(e6) + cos(e4)*cos(e5)*sin(e2)*sin(e3)*sin(e6)) - I6zx*(cos(e2)*cos(e3)*sin(e4)*sin(e6) + cos(e2)*cos(e6)*sin(e3)*sin(e5) + cos(e3)*cos(e6)*sin(e2)*sin(e5) - sin(e2)*sin(e3)*sin(e4)*sin(e6) - cos(e2)*cos(e3)*cos(e4)*cos(e5)*cos(e6) + cos(e4)*cos(e5)*cos(e6)*sin(e2)*sin(e3)) + I6zz*(cos(e2)*cos(e5)*sin(e3) + cos(e3)*cos(e5)*sin(e2) + cos(e2)*cos(e3)*cos(e4)*sin(e5) - cos(e4)*sin(e2)*sin(e3)*sin(e5)))*(cos(e2)*sin(e3)*sin(e5) + cos(e3)*sin(e2)*sin(e5) - cos(e2)*cos(e3)*cos(e4)*cos(e5) + cos(e4)*cos(e5)*sin(e2)*sin(e3)) + (I6xx*(cos(e2)*cos(e3)*sin(e4)*sin(e6) + cos(e2)*cos(e6)*sin(e3)*sin(e5) + cos(e3)*cos(e6)*sin(e2)*sin(e5) - sin(e2)*sin(e3)*sin(e4)*sin(e6) - cos(e2)*cos(e3)*cos(e4)*cos(e5)*cos(e6) + cos(e4)*cos(e5)*cos(e6)*sin(e2)*sin(e3)) + I6xy*(cos(e6)*sin(e2)*sin(e3)*sin(e4) - cos(e2)*cos(e3)*cos(e6)*sin(e4) + cos(e2)*sin(e3)*sin(e5)*sin(e6) + cos(e3)*sin(e2)*sin(e5)*sin(e6) - cos(e2)*cos(e3)*cos(e4)*cos(e5)*sin(e6) + cos(e4)*cos(e5)*sin(e2)*sin(e3)*sin(e6)) - I6zx*(cos(e2)*cos(e5)*sin(e3) + cos(e3)*cos(e5)*sin(e2) + cos(e2)*cos(e3)*cos(e4)*sin(e5) - cos(e4)*sin(e2)*sin(e3)*sin(e5)))*(cos(e2)*cos(e5)*cos(e6)*sin(e3) + cos(e3)*cos(e5)*cos(e6)*sin(e2) + cos(e2)*cos(e3)*cos(e4)*cos(e6)*sin(e5) - cos(e4)*cos(e6)*sin(e2)*sin(e3)*sin(e5)) - 2*m5*(x5*(sin(e5)*(sin(e1)*sin(e4) + sin(e2 + e3)*cos(e1)*cos(e4)) - cos(e2 + e3)*cos(e1)*cos(e5)) + y5*(cos(e5)*(sin(e1)*sin(e4) + sin(e2 + e3)*cos(e1)*cos(e4)) + cos(e2 + e3)*cos(e1)*sin(e5)))*(cos(e1)*(a1 + d4*cos(e2 + e3) + a3*sin(e2 + e3) + a2*sin(e2)) - z5*(cos(e4)*sin(e1) - sin(e2 + e3)*cos(e1)*sin(e4)) + x5*(cos(e5)*(sin(e1)*sin(e4) + sin(e2 + e3)*cos(e1)*cos(e4)) + cos(e2 + e3)*cos(e1)*sin(e5)) - y5*(sin(e5)*(sin(e1)*sin(e4) + sin(e2 + e3)*cos(e1)*cos(e4)) - cos(e2 + e3)*cos(e1)*cos(e5))) - 2*m6*(z6*(cos(e5)*(sin(e1)*sin(e4) + sin(e2 + e3)*cos(e1)*cos(e4)) + cos(e2 + e3)*cos(e1)*sin(e5)) + x6*cos(e6)*(sin(e5)*(sin(e1)*sin(e4) + sin(e2 + e3)*cos(e1)*cos(e4)) - cos(e2 + e3)*cos(e1)*cos(e5)) - y6*sin(e6)*(sin(e5)*(sin(e1)*sin(e4) + sin(e2 + e3)*cos(e1)*cos(e4)) - cos(e2 + e3)*cos(e1)*cos(e5)))*(cos(e1)*(a1 + d4*cos(e2 + e3) + a3*sin(e2 + e3) + a2*sin(e2)) + x6*(sin(e6)*(cos(e4)*sin(e1) - sin(e2 + e3)*cos(e1)*sin(e4)) + cos(e6)*(cos(e5)*(sin(e1)*sin(e4) + sin(e2 + e3)*cos(e1)*cos(e4)) + cos(e2 + e3)*cos(e1)*sin(e5))) + y6*(cos(e6)*(cos(e4)*sin(e1) - sin(e2 + e3)*cos(e1)*sin(e4)) - sin(e6)*(cos(e5)*(sin(e1)*sin(e4) + sin(e2 + e3)*cos(e1)*cos(e4)) + cos(e2 + e3)*cos(e1)*sin(e5))) - z6*(sin(e5)*(sin(e1)*sin(e4) + sin(e2 + e3)*cos(e1)*cos(e4)) - cos(e2 + e3)*cos(e1)*cos(e5))) + 2*m5*(x5*(sin(e5)*(cos(e1)*sin(e4) - sin(e2 + e3)*cos(e4)*sin(e1)) + cos(e2 + e3)*cos(e5)*sin(e1)) + y5*(cos(e5)*(cos(e1)*sin(e4) - sin(e2 + e3)*cos(e4)*sin(e1)) - cos(e2 + e3)*sin(e1)*sin(e5)))*(sin(e1)*(a1 + d4*cos(e2 + e3) + a3*sin(e2 + e3) + a2*sin(e2)) + z5*(cos(e1)*cos(e4) + sin(e2 + e3)*sin(e1)*sin(e4)) - x5*(cos(e5)*(cos(e1)*sin(e4) - sin(e2 + e3)*cos(e4)*sin(e1)) - cos(e2 + e3)*sin(e1)*sin(e5)) + y5*(sin(e5)*(cos(e1)*sin(e4) - sin(e2 + e3)*cos(e4)*sin(e1)) + cos(e2 + e3)*cos(e5)*sin(e1))) + 2*m6*(z6*(cos(e5)*(cos(e1)*sin(e4) - sin(e2 + e3)*cos(e4)*sin(e1)) - cos(e2 + e3)*sin(e1)*sin(e5)) + x6*cos(e6)*(sin(e5)*(cos(e1)*sin(e4) - sin(e2 + e3)*cos(e4)*sin(e1)) + cos(e2 + e3)*cos(e5)*sin(e1)) - y6*sin(e6)*(sin(e5)*(cos(e1)*sin(e4) - sin(e2 + e3)*cos(e4)*sin(e1)) + cos(e2 + e3)*cos(e5)*sin(e1)))*(sin(e1)*(a1 + d4*cos(e2 + e3) + a3*sin(e2 + e3) + a2*sin(e2)) - x6*(sin(e6)*(cos(e1)*cos(e4) + sin(e2 + e3)*sin(e1)*sin(e4)) + cos(e6)*(cos(e5)*(cos(e1)*sin(e4) - sin(e2 + e3)*cos(e4)*sin(e1)) - cos(e2 + e3)*sin(e1)*sin(e5))) - y6*(cos(e6)*(cos(e1)*cos(e4) + sin(e2 + e3)*sin(e1)*sin(e4)) - sin(e6)*(cos(e5)*(cos(e1)*sin(e4) - sin(e2 + e3)*cos(e4)*sin(e1)) - cos(e2 + e3)*sin(e1)*sin(e5))) + z6*(sin(e5)*(cos(e1)*sin(e4) - sin(e2 + e3)*cos(e4)*sin(e1)) + cos(e2 + e3)*cos(e5)*sin(e1)))))/2 + (de2*((I6xx*(cos(e2)*cos(e3)*cos(e6)*sin(e5) - cos(e2)*sin(e3)*sin(e4)*sin(e6) - cos(e3)*sin(e2)*sin(e4)*sin(e6) - cos(e6)*sin(e2)*sin(e3)*sin(e5) + cos(e2)*cos(e4)*cos(e5)*cos(e6)*sin(e3) + cos(e3)*cos(e4)*cos(e5)*cos(e6)*sin(e2)) + I6xy*(cos(e2)*cos(e6)*sin(e3)*sin(e4) + cos(e3)*cos(e6)*sin(e2)*sin(e4) + cos(e2)*cos(e3)*sin(e5)*sin(e6) - sin(e2)*sin(e3)*sin(e5)*sin(e6) + cos(e2)*cos(e4)*cos(e5)*sin(e3)*sin(e6) + cos(e3)*cos(e4)*cos(e5)*sin(e2)*sin(e6)) + I6zx*(cos(e5)*sin(e2)*sin(e3) - cos(e2)*cos(e3)*cos(e5) + cos(e2)*cos(e4)*sin(e3)*sin(e5) + cos(e3)*cos(e4)*sin(e2)*sin(e5)))*(cos(e2)*cos(e3)*sin(e4)*sin(e6) + cos(e2)*cos(e6)*sin(e3)*sin(e5) + cos(e3)*cos(e6)*sin(e2)*sin(e5) - sin(e2)*sin(e3)*sin(e4)*sin(e6) - cos(e2)*cos(e3)*cos(e4)*cos(e5)*cos(e6) + cos(e4)*cos(e5)*cos(e6)*sin(e2)*sin(e3)) + (I6xx*(cos(e2)*cos(e3)*sin(e4)*sin(e6) + cos(e2)*cos(e6)*sin(e3)*sin(e5) + cos(e3)*cos(e6)*sin(e2)*sin(e5) - sin(e2)*sin(e3)*sin(e4)*sin(e6) - cos(e2)*cos(e3)*cos(e4)*cos(e5)*cos(e6) + cos(e4)*cos(e5)*cos(e6)*sin(e2)*sin(e3)) + I6xy*(cos(e6)*sin(e2)*sin(e3)*sin(e4) - cos(e2)*cos(e3)*cos(e6)*sin(e4) + cos(e2)*sin(e3)*sin(e5)*sin(e6) + cos(e3)*sin(e2)*sin(e5)*sin(e6) - cos(e2)*cos(e3)*cos(e4)*cos(e5)*sin(e6) + cos(e4)*cos(e5)*sin(e2)*sin(e3)*sin(e6)) - I6zx*(cos(e2)*cos(e5)*sin(e3) + cos(e3)*cos(e5)*sin(e2) + cos(e2)*cos(e3)*cos(e4)*sin(e5) - cos(e4)*sin(e2)*sin(e3)*sin(e5)))*(cos(e2)*cos(e3)*cos(e6)*sin(e5) - cos(e2)*sin(e3)*sin(e4)*sin(e6) - cos(e3)*sin(e2)*sin(e4)*sin(e6) - cos(e6)*sin(e2)*sin(e3)*sin(e5) + cos(e2)*cos(e4)*cos(e5)*cos(e6)*sin(e3) + cos(e3)*cos(e4)*cos(e5)*cos(e6)*sin(e2)) - (cos(e2)*cos(e3)*cos(e4) - cos(e4)*sin(e2)*sin(e3))*(I4xx*(cos(e2)*cos(e4)*sin(e3) + cos(e3)*cos(e4)*sin(e2)) - I4zx*cos(e2 + e3) + I4xy*(cos(e2)*sin(e3)*sin(e4) + cos(e3)*sin(e2)*sin(e4))) - (cos(e2)*sin(e3)*sin(e4) + cos(e3)*sin(e2)*sin(e4))*(I5zz*(cos(e2)*cos(e3)*sin(e4) - sin(e2)*sin(e3)*sin(e4)) + I5yz*(cos(e2)*cos(e5)*sin(e3) + cos(e3)*cos(e5)*sin(e2) + cos(e2)*cos(e3)*cos(e4)*sin(e5) - cos(e4)*sin(e2)*sin(e3)*sin(e5)) + I5zx*(cos(e2)*sin(e3)*sin(e5) + cos(e3)*sin(e2)*sin(e5) - cos(e2)*cos(e3)*cos(e4)*cos(e5) + cos(e4)*cos(e5)*sin(e2)*sin(e3))) - (cos(e2)*cos(e3)*sin(e4) - sin(e2)*sin(e3)*sin(e4))*(I5zz*(cos(e2)*sin(e3)*sin(e4) + cos(e3)*sin(e2)*sin(e4)) + I5yz*(cos(e5)*sin(e2)*sin(e3) - cos(e2)*cos(e3)*cos(e5) + cos(e2)*cos(e4)*sin(e3)*sin(e5) + cos(e3)*cos(e4)*sin(e2)*sin(e5)) - I5zx*(cos(e2)*cos(e3)*sin(e5) - sin(e2)*sin(e3)*sin(e5) + cos(e2)*cos(e4)*cos(e5)*sin(e3) + cos(e3)*cos(e4)*cos(e5)*sin(e2))) - (cos(e2)*cos(e4)*sin(e3) + cos(e3)*cos(e4)*sin(e2))*(I4zx*sin(e2 + e3) + I4xx*(cos(e2)*cos(e3)*cos(e4) - cos(e4)*sin(e2)*sin(e3)) + I4xy*(cos(e2)*cos(e3)*sin(e4) - sin(e2)*sin(e3)*sin(e4))) + (I6xy*(cos(e2)*cos(e3)*sin(e4)*sin(e6) + cos(e2)*cos(e6)*sin(e3)*sin(e5) + cos(e3)*cos(e6)*sin(e2)*sin(e5) - sin(e2)*sin(e3)*sin(e4)*sin(e6) - cos(e2)*cos(e3)*cos(e4)*cos(e5)*cos(e6) + cos(e4)*cos(e5)*cos(e6)*sin(e2)*sin(e3)) + I6yy*(cos(e6)*sin(e2)*sin(e3)*sin(e4) - cos(e2)*cos(e3)*cos(e6)*sin(e4) + cos(e2)*sin(e3)*sin(e5)*sin(e6) + cos(e3)*sin(e2)*sin(e5)*sin(e6) - cos(e2)*cos(e3)*cos(e4)*cos(e5)*sin(e6) + cos(e4)*cos(e5)*sin(e2)*sin(e3)*sin(e6)) + I6yz*(cos(e2)*cos(e5)*sin(e3) + cos(e3)*cos(e5)*sin(e2) + cos(e2)*cos(e3)*cos(e4)*sin(e5) - cos(e4)*sin(e2)*sin(e3)*sin(e5)))*(cos(e2)*cos(e6)*sin(e3)*sin(e4) + cos(e3)*cos(e6)*sin(e2)*sin(e4) + cos(e2)*cos(e3)*sin(e5)*sin(e6) - sin(e2)*sin(e3)*sin(e5)*sin(e6) + cos(e2)*cos(e4)*cos(e5)*sin(e3)*sin(e6) + cos(e3)*cos(e4)*cos(e5)*sin(e2)*sin(e6)) + (I6xy*(cos(e2)*cos(e3)*cos(e6)*sin(e5) - cos(e2)*sin(e3)*sin(e4)*sin(e6) - cos(e3)*sin(e2)*sin(e4)*sin(e6) - cos(e6)*sin(e2)*sin(e3)*sin(e5) + cos(e2)*cos(e4)*cos(e5)*cos(e6)*sin(e3) + cos(e3)*cos(e4)*cos(e5)*cos(e6)*sin(e2)) + I6yy*(cos(e2)*cos(e6)*sin(e3)*sin(e4) + cos(e3)*cos(e6)*sin(e2)*sin(e4) + cos(e2)*cos(e3)*sin(e5)*sin(e6) - sin(e2)*sin(e3)*sin(e5)*sin(e6) + cos(e2)*cos(e4)*cos(e5)*sin(e3)*sin(e6) + cos(e3)*cos(e4)*cos(e5)*sin(e2)*sin(e6)) - I6yz*(cos(e5)*sin(e2)*sin(e3) - cos(e2)*cos(e3)*cos(e5) + cos(e2)*cos(e4)*sin(e3)*sin(e5) + cos(e3)*cos(e4)*sin(e2)*sin(e5)))*(cos(e6)*sin(e2)*sin(e3)*sin(e4) - cos(e2)*cos(e3)*cos(e6)*sin(e4) + cos(e2)*sin(e3)*sin(e5)*sin(e6) + cos(e3)*sin(e2)*sin(e5)*sin(e6) - cos(e2)*cos(e3)*cos(e4)*cos(e5)*sin(e6) + cos(e4)*cos(e5)*sin(e2)*sin(e3)*sin(e6)) - (cos(e2)*cos(e3)*sin(e4) - sin(e2)*sin(e3)*sin(e4))*(I4yz*cos(e2 + e3) + I4xy*(cos(e2)*cos(e4)*sin(e3) + cos(e3)*cos(e4)*sin(e2)) + I4yy*(cos(e2)*sin(e3)*sin(e4) + cos(e3)*sin(e2)*sin(e4))) + (I5xx*(cos(e2)*cos(e3)*sin(e5) - sin(e2)*sin(e3)*sin(e5) + cos(e2)*cos(e4)*cos(e5)*sin(e3) + cos(e3)*cos(e4)*cos(e5)*sin(e2)) - I5zx*(cos(e2)*sin(e3)*sin(e4) + cos(e3)*sin(e2)*sin(e4)) + I5xy*(cos(e5)*sin(e2)*sin(e3) - cos(e2)*cos(e3)*cos(e5) + cos(e2)*cos(e4)*sin(e3)*sin(e5) + cos(e3)*cos(e4)*sin(e2)*sin(e5)))*(cos(e2)*sin(e3)*sin(e5) + cos(e3)*sin(e2)*sin(e5) - cos(e2)*cos(e3)*cos(e4)*cos(e5) + cos(e4)*cos(e5)*sin(e2)*sin(e3)) + (I5zx*(cos(e2)*cos(e3)*sin(e4) - sin(e2)*sin(e3)*sin(e4)) + I5xx*(cos(e2)*sin(e3)*sin(e5) + cos(e3)*sin(e2)*sin(e5) - cos(e2)*cos(e3)*cos(e4)*cos(e5) + cos(e4)*cos(e5)*sin(e2)*sin(e3)) - I5xy*(cos(e2)*cos(e5)*sin(e3) + cos(e3)*cos(e5)*sin(e2) + cos(e2)*cos(e3)*cos(e4)*sin(e5) - cos(e4)*sin(e2)*sin(e3)*sin(e5)))*(cos(e2)*cos(e3)*sin(e5) - sin(e2)*sin(e3)*sin(e5) + cos(e2)*cos(e4)*cos(e5)*sin(e3) + cos(e3)*cos(e4)*cos(e5)*sin(e2)) - (I5yz*(cos(e2)*sin(e3)*sin(e4) + cos(e3)*sin(e2)*sin(e4)) + I5xy*(cos(e2)*cos(e3)*sin(e5) - sin(e2)*sin(e3)*sin(e5) + cos(e2)*cos(e4)*cos(e5)*sin(e3) + cos(e3)*cos(e4)*cos(e5)*sin(e2)) + I5yy*(cos(e5)*sin(e2)*sin(e3) - cos(e2)*cos(e3)*cos(e5) + cos(e2)*cos(e4)*sin(e3)*sin(e5) + cos(e3)*cos(e4)*sin(e2)*sin(e5)))*(cos(e2)*cos(e5)*sin(e3) + cos(e3)*cos(e5)*sin(e2) + cos(e2)*cos(e3)*cos(e4)*sin(e5) - cos(e4)*sin(e2)*sin(e3)*sin(e5)) - (I5yz*(cos(e2)*cos(e3)*sin(e4) - sin(e2)*sin(e3)*sin(e4)) - I5xy*(cos(e2)*sin(e3)*sin(e5) + cos(e3)*sin(e2)*sin(e5) - cos(e2)*cos(e3)*cos(e4)*cos(e5) + cos(e4)*cos(e5)*sin(e2)*sin(e3)) + I5yy*(cos(e2)*cos(e5)*sin(e3) + cos(e3)*cos(e5)*sin(e2) + cos(e2)*cos(e3)*cos(e4)*sin(e5) - cos(e4)*sin(e2)*sin(e3)*sin(e5)))*(cos(e5)*sin(e2)*sin(e3) - cos(e2)*cos(e3)*cos(e5) + cos(e2)*cos(e4)*sin(e3)*sin(e5) + cos(e3)*cos(e4)*sin(e2)*sin(e5)) - (cos(e2)*sin(e3)*sin(e4) + cos(e3)*sin(e2)*sin(e4))*(I4xy*(cos(e2)*cos(e3)*cos(e4) - cos(e4)*sin(e2)*sin(e3)) - I4yz*sin(e2 + e3) + I4yy*(cos(e2)*cos(e3)*sin(e4) - sin(e2)*sin(e3)*sin(e4))) + cos(e2)*(I2xy*cos(e2) - I2xx*sin(e2)) + cos(e2)*(I2xy*cos(e2) + I2yy*sin(e2)) - sin(e2)*(I2xx*cos(e2) + I2xy*sin(e2)) + sin(e2)*(I2yy*cos(e2) - I2xy*sin(e2)) - (I6zx*(cos(e2)*cos(e3)*cos(e6)*sin(e5) - cos(e2)*sin(e3)*sin(e4)*sin(e6) - cos(e3)*sin(e2)*sin(e4)*sin(e6) - cos(e6)*sin(e2)*sin(e3)*sin(e5) + cos(e2)*cos(e4)*cos(e5)*cos(e6)*sin(e3) + cos(e3)*cos(e4)*cos(e5)*cos(e6)*sin(e2)) - I6yz*(cos(e2)*cos(e6)*sin(e3)*sin(e4) + cos(e3)*cos(e6)*sin(e2)*sin(e4) + cos(e2)*cos(e3)*sin(e5)*sin(e6) - sin(e2)*sin(e3)*sin(e5)*sin(e6) + cos(e2)*cos(e4)*cos(e5)*sin(e3)*sin(e6) + cos(e3)*cos(e4)*cos(e5)*sin(e2)*sin(e6)) + I6zz*(cos(e5)*sin(e2)*sin(e3) - cos(e2)*cos(e3)*cos(e5) + cos(e2)*cos(e4)*sin(e3)*sin(e5) + cos(e3)*cos(e4)*sin(e2)*sin(e5)))*(cos(e2)*cos(e5)*sin(e3) + cos(e3)*cos(e5)*sin(e2) + cos(e2)*cos(e3)*cos(e4)*sin(e5) - cos(e4)*sin(e2)*sin(e3)*sin(e5)) - (I6yz*(cos(e6)*sin(e2)*sin(e3)*sin(e4) - cos(e2)*cos(e3)*cos(e6)*sin(e4) + cos(e2)*sin(e3)*sin(e5)*sin(e6) + cos(e3)*sin(e2)*sin(e5)*sin(e6) - cos(e2)*cos(e3)*cos(e4)*cos(e5)*sin(e6) + cos(e4)*cos(e5)*sin(e2)*sin(e3)*sin(e6)) - I6zx*(cos(e2)*cos(e3)*sin(e4)*sin(e6) + cos(e2)*cos(e6)*sin(e3)*sin(e5) + cos(e3)*cos(e6)*sin(e2)*sin(e5) - sin(e2)*sin(e3)*sin(e4)*sin(e6) - cos(e2)*cos(e3)*cos(e4)*cos(e5)*cos(e6) + cos(e4)*cos(e5)*cos(e6)*sin(e2)*sin(e3)) + I6zz*(cos(e2)*cos(e5)*sin(e3) + cos(e3)*cos(e5)*sin(e2) + cos(e2)*cos(e3)*cos(e4)*sin(e5) - cos(e4)*sin(e2)*sin(e3)*sin(e5)))*(cos(e5)*sin(e2)*sin(e3) - cos(e2)*cos(e3)*cos(e5) + cos(e2)*cos(e4)*sin(e3)*sin(e5) + cos(e3)*cos(e4)*sin(e2)*sin(e5)) + cos(e2 + e3)*(I3xy*cos(e2 + e3) - I3xx*sin(e2 + e3)) + cos(e2 + e3)*(I3xy*cos(e2 + e3) + I3yy*sin(e2 + e3)) - sin(e2 + e3)*(I3xx*cos(e2 + e3) + I3xy*sin(e2 + e3)) + sin(e2 + e3)*(I3yy*cos(e2 + e3) - I3xy*sin(e2 + e3)) + sin(e2 + e3)*(I4zz*cos(e2 + e3) - I4zx*(cos(e2)*cos(e4)*sin(e3) + cos(e3)*cos(e4)*sin(e2)) + I4yz*(cos(e2)*sin(e3)*sin(e4) + cos(e3)*sin(e2)*sin(e4))) + cos(e2 + e3)*(I4zz*sin(e2 + e3) + I4zx*(cos(e2)*cos(e3)*cos(e4) - cos(e4)*sin(e2)*sin(e3)) - I4yz*(cos(e2)*cos(e3)*sin(e4) - sin(e2)*sin(e3)*sin(e4))) + 2*m3*(x3*cos(e2 + e3)*sin(e1) - y3*sin(e2 + e3)*sin(e1) + a2*cos(e2)*sin(e1))*(sin(e1)*(a1 + a2*sin(e2)) + z3*cos(e1) + y3*cos(e2 + e3)*sin(e1) + x3*sin(e2 + e3)*sin(e1)) - 2*m5*(cos(e1)*(a1 + d4*cos(e2 + e3) + a3*sin(e2 + e3) + a2*sin(e2)) - z5*(cos(e4)*sin(e1) - sin(e2 + e3)*cos(e1)*sin(e4)) + x5*(cos(e5)*(sin(e1)*sin(e4) + sin(e2 + e3)*cos(e1)*cos(e4)) + cos(e2 + e3)*cos(e1)*sin(e5)) - y5*(sin(e5)*(sin(e1)*sin(e4) + sin(e2 + e3)*cos(e1)*cos(e4)) - cos(e2 + e3)*cos(e1)*cos(e5)))*(x5*(sin(e2 + e3)*cos(e1)*sin(e5) - cos(e2 + e3)*cos(e1)*cos(e4)*cos(e5)) + y5*(sin(e2 + e3)*cos(e1)*cos(e5) + cos(e2 + e3)*cos(e1)*cos(e4)*sin(e5)) - cos(e1)*(a3*cos(e2 + e3) - d4*sin(e2 + e3) + a2*cos(e2)) - z5*cos(e2 + e3)*cos(e1)*sin(e4)) + 2*m2*(x2*cos(e1)*cos(e2) - y2*cos(e1)*sin(e2))*(a1*cos(e1) - z2*sin(e1) + y2*cos(e1)*cos(e2) + x2*cos(e1)*sin(e2)) + 2*m4*(cos(e1)*(a3*cos(e2 + e3) - d4*sin(e2 + e3) + a2*cos(e2)) - z4*sin(e2 + e3)*cos(e1) - y4*cos(e2 + e3)*cos(e1)*sin(e4) + x4*cos(e2 + e3)*cos(e1)*cos(e4))*(cos(e1)*(a1 + d4*cos(e2 + e3) + a3*sin(e2 + e3) + a2*sin(e2)) + x4*(sin(e1)*sin(e4) + sin(e2 + e3)*cos(e1)*cos(e4)) + y4*(cos(e4)*sin(e1) - sin(e2 + e3)*cos(e1)*sin(e4)) + z4*cos(e2 + e3)*cos(e1)) - 2*m6*(sin(e1)*(a1 + d4*cos(e2 + e3) + a3*sin(e2 + e3) + a2*sin(e2)) - x6*(sin(e6)*(cos(e1)*cos(e4) + sin(e2 + e3)*sin(e1)*sin(e4)) + cos(e6)*(cos(e5)*(cos(e1)*sin(e4) - sin(e2 + e3)*cos(e4)*sin(e1)) - cos(e2 + e3)*sin(e1)*sin(e5))) - y6*(cos(e6)*(cos(e1)*cos(e4) + sin(e2 + e3)*sin(e1)*sin(e4)) - sin(e6)*(cos(e5)*(cos(e1)*sin(e4) - sin(e2 + e3)*cos(e4)*sin(e1)) - cos(e2 + e3)*sin(e1)*sin(e5))) + z6*(sin(e5)*(cos(e1)*sin(e4) - sin(e2 + e3)*cos(e4)*sin(e1)) + cos(e2 + e3)*cos(e5)*sin(e1)))*(x6*(cos(e6)*(sin(e2 + e3)*sin(e1)*sin(e5) - cos(e2 + e3)*cos(e4)*cos(e5)*sin(e1)) + cos(e2 + e3)*sin(e1)*sin(e4)*sin(e6)) - y6*(sin(e6)*(sin(e2 + e3)*sin(e1)*sin(e5) - cos(e2 + e3)*cos(e4)*cos(e5)*sin(e1)) - cos(e2 + e3)*cos(e6)*sin(e1)*sin(e4)) + z6*(sin(e2 + e3)*cos(e5)*sin(e1) + cos(e2 + e3)*cos(e4)*sin(e1)*sin(e5)) - sin(e1)*(a3*cos(e2 + e3) - d4*sin(e2 + e3) + a2*cos(e2))) + 2*m2*(x2*cos(e2)*sin(e1) - y2*sin(e1)*sin(e2))*(a1*sin(e1) + z2*cos(e1) + y2*cos(e2)*sin(e1) + x2*sin(e1)*sin(e2)) - 2*m6*(x6*(cos(e6)*(sin(e2 + e3)*cos(e1)*sin(e5) - cos(e2 + e3)*cos(e1)*cos(e4)*cos(e5)) + cos(e2 + e3)*cos(e1)*sin(e4)*sin(e6)) - y6*(sin(e6)*(sin(e2 + e3)*cos(e1)*sin(e5) - cos(e2 + e3)*cos(e1)*cos(e4)*cos(e5)) - cos(e2 + e3)*cos(e1)*cos(e6)*sin(e4)) + z6*(sin(e2 + e3)*cos(e1)*cos(e5) + cos(e2 + e3)*cos(e1)*cos(e4)*sin(e5)) - cos(e1)*(a3*cos(e2 + e3) - d4*sin(e2 + e3) + a2*cos(e2)))*(cos(e1)*(a1 + d4*cos(e2 + e3) + a3*sin(e2 + e3) + a2*sin(e2)) + x6*(sin(e6)*(cos(e4)*sin(e1) - sin(e2 + e3)*cos(e1)*sin(e4)) + cos(e6)*(cos(e5)*(sin(e1)*sin(e4) + sin(e2 + e3)*cos(e1)*cos(e4)) + cos(e2 + e3)*cos(e1)*sin(e5))) + y6*(cos(e6)*(cos(e4)*sin(e1) - sin(e2 + e3)*cos(e1)*sin(e4)) - sin(e6)*(cos(e5)*(sin(e1)*sin(e4) + sin(e2 + e3)*cos(e1)*cos(e4)) + cos(e2 + e3)*cos(e1)*sin(e5))) - z6*(sin(e5)*(sin(e1)*sin(e4) + sin(e2 + e3)*cos(e1)*cos(e4)) - cos(e2 + e3)*cos(e1)*cos(e5))) + 2*m3*(x3*cos(e2 + e3)*cos(e1) - y3*sin(e2 + e3)*cos(e1) + a2*cos(e1)*cos(e2))*(cos(e1)*(a1 + a2*sin(e2)) - z3*sin(e1) + y3*cos(e2 + e3)*cos(e1) + x3*sin(e2 + e3)*cos(e1)) + 2*m4*(sin(e1)*(a1 + d4*cos(e2 + e3) + a3*sin(e2 + e3) + a2*sin(e2)) - x4*(cos(e1)*sin(e4) - sin(e2 + e3)*cos(e4)*sin(e1)) - y4*(cos(e1)*cos(e4) + sin(e2 + e3)*sin(e1)*sin(e4)) + z4*cos(e2 + e3)*sin(e1))*(sin(e1)*(a3*cos(e2 + e3) - d4*sin(e2 + e3) + a2*cos(e2)) - z4*sin(e2 + e3)*sin(e1) + x4*cos(e2 + e3)*cos(e4)*sin(e1) - y4*cos(e2 + e3)*sin(e1)*sin(e4)) - 2*m5*(sin(e1)*(a1 + d4*cos(e2 + e3) + a3*sin(e2 + e3) + a2*sin(e2)) + z5*(cos(e1)*cos(e4) + sin(e2 + e3)*sin(e1)*sin(e4)) - x5*(cos(e5)*(cos(e1)*sin(e4) - sin(e2 + e3)*cos(e4)*sin(e1)) - cos(e2 + e3)*sin(e1)*sin(e5)) + y5*(sin(e5)*(cos(e1)*sin(e4) - sin(e2 + e3)*cos(e4)*sin(e1)) + cos(e2 + e3)*cos(e5)*sin(e1)))*(x5*(sin(e2 + e3)*sin(e1)*sin(e5) - cos(e2 + e3)*cos(e4)*cos(e5)*sin(e1)) + y5*(sin(e2 + e3)*cos(e5)*sin(e1) + cos(e2 + e3)*cos(e4)*sin(e1)*sin(e5)) - sin(e1)*(a3*cos(e2 + e3) - d4*sin(e2 + e3) + a2*cos(e2)) - z5*cos(e2 + e3)*sin(e1)*sin(e4))))/2 - (de4*((sin(2*e2 + 2*e3)*(I4yz*cos(e4) + I4zx*sin(e4)))/2 - cos(e2 + e3)*cos(e4)*(I5zz*cos(e2 + e3)*sin(e4) + I5yz*cos(e2)*cos(e5)*sin(e3) + I5yz*cos(e3)*cos(e5)*sin(e2) + I5zx*cos(e2)*sin(e3)*sin(e5) + I5zx*cos(e3)*sin(e2)*sin(e5) - I5zx*cos(e2)*cos(e3)*cos(e4)*cos(e5) + I5yz*cos(e2)*cos(e3)*cos(e4)*sin(e5) + I5zx*cos(e4)*cos(e5)*sin(e2)*sin(e3) - I5yz*cos(e4)*sin(e2)*sin(e3)*sin(e5)) - cos(e2 + e3)*(I6xx*cos(e4)*sin(e6) - I6xy*cos(e4)*cos(e6) + I6zx*sin(e4)*sin(e5) + I6xx*cos(e5)*cos(e6)*sin(e4) + I6xy*cos(e5)*sin(e4)*sin(e6))*(cos(e2)*cos(e3)*sin(e4)*sin(e6) + cos(e2)*cos(e6)*sin(e3)*sin(e5) + cos(e3)*cos(e6)*sin(e2)*sin(e5) - sin(e2)*sin(e3)*sin(e4)*sin(e6) - cos(e2)*cos(e3)*cos(e4)*cos(e5)*cos(e6) + cos(e4)*cos(e5)*cos(e6)*sin(e2)*sin(e3)) - cos(e2 + e3)*(cos(e4)*sin(e6) + cos(e5)*cos(e6)*sin(e4))*(I6xx*(cos(e2)*cos(e3)*sin(e4)*sin(e6) + cos(e2)*cos(e6)*sin(e3)*sin(e5) + cos(e3)*cos(e6)*sin(e2)*sin(e5) - sin(e2)*sin(e3)*sin(e4)*sin(e6) - cos(e2)*cos(e3)*cos(e4)*cos(e5)*cos(e6) + cos(e4)*cos(e5)*cos(e6)*sin(e2)*sin(e3)) + I6xy*(cos(e6)*sin(e2)*sin(e3)*sin(e4) - cos(e2)*cos(e3)*cos(e6)*sin(e4) + cos(e2)*sin(e3)*sin(e5)*sin(e6) + cos(e3)*sin(e2)*sin(e5)*sin(e6) - cos(e2)*cos(e3)*cos(e4)*cos(e5)*sin(e6) + cos(e4)*cos(e5)*sin(e2)*sin(e3)*sin(e6)) - I6zx*(cos(e2)*cos(e5)*sin(e3) + cos(e3)*cos(e5)*sin(e2) + cos(e2)*cos(e3)*cos(e4)*sin(e5) - cos(e4)*sin(e2)*sin(e3)*sin(e5))) + cos(e2 + e3)*(cos(e4)*cos(e6) - cos(e5)*sin(e4)*sin(e6))*(I6xy*(cos(e2)*cos(e3)*sin(e4)*sin(e6) + cos(e2)*cos(e6)*sin(e3)*sin(e5) + cos(e3)*cos(e6)*sin(e2)*sin(e5) - sin(e2)*sin(e3)*sin(e4)*sin(e6) - cos(e2)*cos(e3)*cos(e4)*cos(e5)*cos(e6) + cos(e4)*cos(e5)*cos(e6)*sin(e2)*sin(e3)) + I6yy*(cos(e6)*sin(e2)*sin(e3)*sin(e4) - cos(e2)*cos(e3)*cos(e6)*sin(e4) + cos(e2)*sin(e3)*sin(e5)*sin(e6) + cos(e3)*sin(e2)*sin(e5)*sin(e6) - cos(e2)*cos(e3)*cos(e4)*cos(e5)*sin(e6) + cos(e4)*cos(e5)*sin(e2)*sin(e3)*sin(e6)) + I6yz*(cos(e2)*cos(e5)*sin(e3) + cos(e3)*cos(e5)*sin(e2) + cos(e2)*cos(e3)*cos(e4)*sin(e5) - cos(e4)*sin(e2)*sin(e3)*sin(e5))) - 2*m5*(cos(e1)*(a1 + d4*cos(e2 + e3) + a3*sin(e2 + e3) + a2*sin(e2)) - y5*(sin(e1)*sin(e4)*sin(e5) - cos(e2 + e3)*cos(e1)*cos(e5) + sin(e2 + e3)*cos(e1)*cos(e4)*sin(e5)) + x5*(cos(e2 + e3)*cos(e1)*sin(e5) + cos(e5)*sin(e1)*sin(e4) + sin(e2 + e3)*cos(e1)*cos(e4)*cos(e5)) - z5*cos(e4)*sin(e1) + z5*sin(e2 + e3)*cos(e1)*sin(e4))*(z5*sin(e1)*sin(e4) + z5*sin(e2 + e3)*cos(e1)*cos(e4) + x5*cos(e4)*cos(e5)*sin(e1) - y5*cos(e4)*sin(e1)*sin(e5) - x5*sin(e2 + e3)*cos(e1)*cos(e5)*sin(e4) + y5*sin(e2 + e3)*cos(e1)*sin(e4)*sin(e5)) - cos(e2 + e3)*(I6xy*cos(e4)*sin(e6) - I6yy*cos(e4)*cos(e6) - I6yz*sin(e4)*sin(e5) + I6xy*cos(e5)*cos(e6)*sin(e4) + I6yy*cos(e5)*sin(e4)*sin(e6))*(cos(e6)*sin(e2)*sin(e3)*sin(e4) - cos(e2)*cos(e3)*cos(e6)*sin(e4) + cos(e2)*sin(e3)*sin(e5)*sin(e6) + cos(e3)*sin(e2)*sin(e5)*sin(e6) - cos(e2)*cos(e3)*cos(e4)*cos(e5)*sin(e6) + cos(e4)*cos(e5)*sin(e2)*sin(e3)*sin(e6)) - cos(e2 + e3)^2*cos(e4)*(I4xy*cos(e4) - I4xx*sin(e4)) - cos(e2 + e3)^2*sin(e4)*(I4yy*cos(e4) - I4xy*sin(e4)) + 2*m6*(x6*(sin(e6)*(sin(e1)*sin(e4) + sin(e2 + e3)*cos(e1)*cos(e4)) - cos(e5)*cos(e6)*(cos(e4)*sin(e1) - sin(e2 + e3)*cos(e1)*sin(e4))) + y6*(cos(e6)*(sin(e1)*sin(e4) + sin(e2 + e3)*cos(e1)*cos(e4)) + cos(e5)*sin(e6)*(cos(e4)*sin(e1) - sin(e2 + e3)*cos(e1)*sin(e4))) + z6*sin(e5)*(cos(e4)*sin(e1) - sin(e2 + e3)*cos(e1)*sin(e4)))*(cos(e1)*(a1 + d4*cos(e2 + e3) + a3*sin(e2 + e3) + a2*sin(e2)) - z6*(sin(e1)*sin(e4)*sin(e5) - cos(e2 + e3)*cos(e1)*cos(e5) + sin(e2 + e3)*cos(e1)*cos(e4)*sin(e5)) + x6*(sin(e6)*(cos(e4)*sin(e1) - sin(e2 + e3)*cos(e1)*sin(e4)) + cos(e6)*(cos(e2 + e3)*cos(e1)*sin(e5) + cos(e5)*sin(e1)*sin(e4) + sin(e2 + e3)*cos(e1)*cos(e4)*cos(e5))) + y6*(cos(e6)*(cos(e4)*sin(e1) - sin(e2 + e3)*cos(e1)*sin(e4)) - sin(e6)*(cos(e2 + e3)*cos(e1)*sin(e5) + cos(e5)*sin(e1)*sin(e4) + sin(e2 + e3)*cos(e1)*cos(e4)*cos(e5)))) + 2*m4*(x4*cos(e1)*cos(e4) - y4*cos(e1)*sin(e4) + y4*sin(e2 + e3)*cos(e4)*sin(e1) + x4*sin(e2 + e3)*sin(e1)*sin(e4))*(sin(e1)*(a1 + d4*cos(e2 + e3) + a3*sin(e2 + e3) + a2*sin(e2)) - y4*(cos(e1)*cos(e4) + sin(e2 + e3)*sin(e1)*sin(e4)) + z4*cos(e2 + e3)*sin(e1) - x4*cos(e1)*sin(e4) + x4*sin(e2 + e3)*cos(e4)*sin(e1)) + cos(e2 + e3)*(cos(e2)*cos(e5)*sin(e3) + cos(e3)*cos(e5)*sin(e2) + cos(e2)*cos(e3)*cos(e4)*sin(e5) - cos(e4)*sin(e2)*sin(e3)*sin(e5))*(I6yz*cos(e4)*cos(e6) + I6zx*cos(e4)*sin(e6) + I6zz*sin(e4)*sin(e5) + I6zx*cos(e5)*cos(e6)*sin(e4) - I6yz*cos(e5)*sin(e4)*sin(e6)) - cos(e2 + e3)*(I5zx*cos(e4) + I5xx*cos(e5)*sin(e4) + I5xy*sin(e4)*sin(e5))*(cos(e2)*sin(e3)*sin(e5) + cos(e3)*sin(e2)*sin(e5) - cos(e2)*cos(e3)*cos(e4)*cos(e5) + cos(e4)*cos(e5)*sin(e2)*sin(e3)) + cos(e2 + e3)*(I5xy*cos(e5)*sin(e4) - I5yz*cos(e4) + I5yy*sin(e4)*sin(e5))*(cos(e2)*cos(e5)*sin(e3) + cos(e3)*cos(e5)*sin(e2) + cos(e2)*cos(e3)*cos(e4)*sin(e5) - cos(e4)*sin(e2)*sin(e3)*sin(e5)) - cos(e2 + e3)^2*sin(e4)*(I5zz*cos(e4) + I5zx*cos(e5)*sin(e4) - I5yz*sin(e4)*sin(e5)) + 2*m4*(cos(e1)*(a1 + d4*cos(e2 + e3) + a3*sin(e2 + e3) + a2*sin(e2)) + x4*(sin(e1)*sin(e4) + sin(e2 + e3)*cos(e1)*cos(e4)) + y4*(cos(e4)*sin(e1) - sin(e2 + e3)*cos(e1)*sin(e4)) + z4*cos(e2 + e3)*cos(e1))*(y4*sin(e1)*sin(e4) - x4*cos(e4)*sin(e1) + y4*sin(e2 + e3)*cos(e1)*cos(e4) + x4*sin(e2 + e3)*cos(e1)*sin(e4)) - 2*m6*(x6*(sin(e6)*(cos(e1)*sin(e4) - sin(e2 + e3)*cos(e4)*sin(e1)) - cos(e5)*cos(e6)*(cos(e1)*cos(e4) + sin(e2 + e3)*sin(e1)*sin(e4))) + y6*(cos(e6)*(cos(e1)*sin(e4) - sin(e2 + e3)*cos(e4)*sin(e1)) + cos(e5)*sin(e6)*(cos(e1)*cos(e4) + sin(e2 + e3)*sin(e1)*sin(e4))) + z6*sin(e5)*(cos(e1)*cos(e4) + sin(e2 + e3)*sin(e1)*sin(e4)))*(z6*(cos(e2 + e3)*cos(e5)*sin(e1) + cos(e1)*sin(e4)*sin(e5) - sin(e2 + e3)*cos(e4)*sin(e1)*sin(e5)) + sin(e1)*(a1 + d4*cos(e2 + e3) + a3*sin(e2 + e3) + a2*sin(e2)) - y6*(cos(e1)*cos(e4)*cos(e6) + sin(e2 + e3)*cos(e6)*sin(e1)*sin(e4) + cos(e2 + e3)*sin(e1)*sin(e5)*sin(e6) - cos(e1)*cos(e5)*sin(e4)*sin(e6) + sin(e2 + e3)*cos(e4)*cos(e5)*sin(e1)*sin(e6)) - x6*(sin(e6)*(cos(e1)*cos(e4) + sin(e2 + e3)*sin(e1)*sin(e4)) - cos(e6)*(cos(e2 + e3)*sin(e1)*sin(e5) - cos(e1)*cos(e5)*sin(e4) + sin(e2 + e3)*cos(e4)*cos(e5)*sin(e1)))) + cos(e2 + e3)*cos(e4)*(I4yz*sin(e2 + e3) - I4xy*cos(e2)*cos(e3)*cos(e4) - I4yy*cos(e2)*cos(e3)*sin(e4) + I4xy*cos(e4)*sin(e2)*sin(e3) + I4yy*sin(e2)*sin(e3)*sin(e4)) + cos(e2 + e3)*sin(e4)*(I4zx*sin(e2 + e3) + I4xx*cos(e2)*cos(e3)*cos(e4) + I4xy*cos(e2)*cos(e3)*sin(e4) - I4xx*cos(e4)*sin(e2)*sin(e3) - I4xy*sin(e2)*sin(e3)*sin(e4)) + 2*m5*(z5*(cos(e1)*sin(e4) - sin(e2 + e3)*cos(e4)*sin(e1)) + x5*cos(e5)*(cos(e1)*cos(e4) + sin(e2 + e3)*sin(e1)*sin(e4)) - y5*sin(e5)*(cos(e1)*cos(e4) + sin(e2 + e3)*sin(e1)*sin(e4)))*(x5*(cos(e2 + e3)*sin(e1)*sin(e5) - cos(e1)*cos(e5)*sin(e4) + sin(e2 + e3)*cos(e4)*cos(e5)*sin(e1)) + y5*(cos(e2 + e3)*cos(e5)*sin(e1) + cos(e1)*sin(e4)*sin(e5) - sin(e2 + e3)*cos(e4)*sin(e1)*sin(e5)) + sin(e1)*(a1 + d4*cos(e2 + e3) + a3*sin(e2 + e3) + a2*sin(e2)) + z5*(cos(e1)*cos(e4) + sin(e2 + e3)*sin(e1)*sin(e4))) + cos(e2 + e3)*sin(e4)*sin(e5)*(I6yz*(cos(e6)*sin(e2)*sin(e3)*sin(e4) - cos(e2)*cos(e3)*cos(e6)*sin(e4) + cos(e2)*sin(e3)*sin(e5)*sin(e6) + cos(e3)*sin(e2)*sin(e5)*sin(e6) - cos(e2)*cos(e3)*cos(e4)*cos(e5)*sin(e6) + cos(e4)*cos(e5)*sin(e2)*sin(e3)*sin(e6)) - I6zx*(cos(e2)*cos(e3)*sin(e4)*sin(e6) + cos(e2)*cos(e6)*sin(e3)*sin(e5) + cos(e3)*cos(e6)*sin(e2)*sin(e5) - sin(e2)*sin(e3)*sin(e4)*sin(e6) - cos(e2)*cos(e3)*cos(e4)*cos(e5)*cos(e6) + cos(e4)*cos(e5)*cos(e6)*sin(e2)*sin(e3)) + I6zz*(cos(e2)*cos(e5)*sin(e3) + cos(e3)*cos(e5)*sin(e2) + cos(e2)*cos(e3)*cos(e4)*sin(e5) - cos(e4)*sin(e2)*sin(e3)*sin(e5))) - cos(e2 + e3)*cos(e5)*sin(e4)*(I5zx*cos(e2 + e3)*sin(e4) - I5xy*cos(e2)*cos(e5)*sin(e3) - I5xy*cos(e3)*cos(e5)*sin(e2) + I5xx*cos(e2)*sin(e3)*sin(e5) + I5xx*cos(e3)*sin(e2)*sin(e5) - I5xx*cos(e2)*cos(e3)*cos(e4)*cos(e5) - I5xy*cos(e2)*cos(e3)*cos(e4)*sin(e5) + I5xx*cos(e4)*cos(e5)*sin(e2)*sin(e3) + I5xy*cos(e4)*sin(e2)*sin(e3)*sin(e5)) + cos(e2 + e3)*sin(e4)*sin(e5)*(I5yz*cos(e2 + e3)*sin(e4) + I5yy*cos(e2)*cos(e5)*sin(e3) + I5yy*cos(e3)*cos(e5)*sin(e2) - I5xy*cos(e2)*sin(e3)*sin(e5) - I5xy*cos(e3)*sin(e2)*sin(e5) + I5xy*cos(e2)*cos(e3)*cos(e4)*cos(e5) + I5yy*cos(e2)*cos(e3)*cos(e4)*sin(e5) - I5xy*cos(e4)*cos(e5)*sin(e2)*sin(e3) - I5yy*cos(e4)*sin(e2)*sin(e3)*sin(e5))))/2,I3xy*de1 - I2xy*de1 + 2*I2xy*de1*cos(e2)^2 - 2*I3xy*de1*cos(e2)^2 - 2*I3xy*de1*cos(e3)^2 - (I2xx*de1*sin(2*e2))/2 + (I3xx*de1*sin(2*e2))/2 + (I3xx*de1*sin(2*e3))/2 - (I5xx*de1*sin(2*e2))/2 - (I5xx*de1*sin(2*e3))/2 + (I6xx*de1*sin(2*e2))/2 + (I6xx*de1*sin(2*e3))/2 + (I2yy*de1*sin(2*e2))/2 - (I3yy*de1*sin(2*e2))/2 - (I3yy*de1*sin(2*e3))/2 + (I4yy*de1*sin(2*e2))/2 + (I4yy*de1*sin(2*e3))/2 - (I6yy*de1*sin(2*e2))/2 - (I6yy*de1*sin(2*e3))/2 - (I4zz*de1*sin(2*e2))/2 - (I4zz*de1*sin(2*e3))/2 + (I5zz*de1*sin(2*e2))/2 + (I5zz*de1*sin(2*e3))/2 - I5xy*de1*cos(e4) + I2yz*de2*cos(e2) + I4zx*de1*cos(e4) - I4yz*de1*sin(e4) + I2zx*de2*sin(e2) + a3*de1*m4*z4 + 2*I4yz*de1*cos(e2)^2*sin(e4) + 2*I4yz*de1*cos(e3)^2*sin(e4) - de1*m2*x2*y2 + de1*m3*x3*y3 + (a2^2*de1*m3*sin(2*e2))/2 + (a2^2*de1*m4*sin(2*e2))/2 + (a2^2*de1*m5*sin(2*e2))/2 - (a3^2*de1*m4*sin(2*e2))/2 + (a2^2*de1*m6*sin(2*e2))/2 - (a3^2*de1*m4*sin(2*e3))/2 - (a3^2*de1*m5*sin(2*e2))/2 - (a3^2*de1*m5*sin(2*e3))/2 - (a3^2*de1*m6*sin(2*e2))/2 - (a3^2*de1*m6*sin(2*e3))/2 + (d4^2*de1*m4*sin(2*e2))/2 + (d4^2*de1*m4*sin(2*e3))/2 + (d4^2*de1*m5*sin(2*e2))/2 + (d4^2*de1*m5*sin(2*e3))/2 + (d4^2*de1*m6*sin(2*e2))/2 + (d4^2*de1*m6*sin(2*e3))/2 + (de1*m2*x2^2*sin(2*e2))/2 - (de1*m3*x3^2*sin(2*e2))/2 - (de1*m3*x3^2*sin(2*e3))/2 + (de1*m5*x5^2*sin(2*e2))/2 + (de1*m5*x5^2*sin(2*e3))/2 - (de1*m6*x6^2*sin(2*e2))/2 - (de1*m6*x6^2*sin(2*e3))/2 - (de1*m2*y2^2*sin(2*e2))/2 + (de1*m3*y3^2*sin(2*e2))/2 + (de1*m3*y3^2*sin(2*e3))/2 - (de1*m4*y4^2*sin(2*e2))/2 - (de1*m4*y4^2*sin(2*e3))/2 + (de1*m6*y6^2*sin(2*e2))/2 + (de1*m6*y6^2*sin(2*e3))/2 + (de1*m4*z4^2*sin(2*e2))/2 + (de1*m4*z4^2*sin(2*e3))/2 - (de1*m5*z5^2*sin(2*e2))/2 - (de1*m5*z5^2*sin(2*e3))/2 + 4*I3xy*de1*cos(e2)^2*cos(e3)^2 + (I4xx*de4*cos(e2)*cos(e3))/2 - (I5xx*de4*cos(e2)*cos(e3))/2 - (I6xx*de4*cos(e2)*cos(e3))/2 + I3yz*de2*cos(e2)*cos(e3) + I3yz*de3*cos(e2)*cos(e3) - (I4yy*de4*cos(e2)*cos(e3))/2 + (I5yy*de4*cos(e2)*cos(e3))/2 - (I6yy*de4*cos(e2)*cos(e3))/2 - (I4zz*de4*cos(e2)*cos(e3))/2 - (I5zz*de4*cos(e2)*cos(e3))/2 - I6zx*de1*cos(e4)*cos(e6) + (I6zz*de4*cos(e2)*cos(e3))/2 + I4xy*de2*cos(e2)*sin(e3) + I4xy*de2*cos(e3)*sin(e2) + I4xy*de3*cos(e2)*sin(e3) + I4xy*de3*cos(e3)*sin(e2) + I5yz*de1*cos(e5)*sin(e4) + I6yz*de1*cos(e4)*sin(e6) + I3zx*de2*cos(e2)*sin(e3) + I3zx*de2*cos(e3)*sin(e2) + I3zx*de3*cos(e2)*sin(e3) + I3zx*de3*cos(e3)*sin(e2) - (I4xx*de4*sin(e2)*sin(e3))/2 + (I5xx*de4*sin(e2)*sin(e3))/2 + (I6xx*de4*sin(e2)*sin(e3))/2 + I6xy*de1*sin(e4)*sin(e5) - I3yz*de2*sin(e2)*sin(e3) - I3yz*de3*sin(e2)*sin(e3) + (I4yy*de4*sin(e2)*sin(e3))/2 - (I5yy*de4*sin(e2)*sin(e3))/2 + (I6yy*de4*sin(e2)*sin(e3))/2 + I5zx*de1*sin(e4)*sin(e5) + (I4zz*de4*sin(e2)*sin(e3))/2 + (I5zz*de4*sin(e2)*sin(e3))/2 - (I6zz*de4*sin(e2)*sin(e3))/2 + a3*d4*de1*m4 + a3*d4*de1*m5 + a3*d4*de1*m6 + 2*I5xy*de1*cos(e2)^2*cos(e4) + 2*I5xy*de1*cos(e3)^2*cos(e4) + 2*I5xy*de1*cos(e4)*cos(e5)^2 - 2*I4zx*de1*cos(e2)^2*cos(e4) - 2*I4zx*de1*cos(e3)^2*cos(e4) - 2*a3*d4*de1*m4*cos(e2)^2 - 2*a3*d4*de1*m4*cos(e3)^2 - 2*a3*d4*de1*m5*cos(e2)^2 - 2*a3*d4*de1*m5*cos(e3)^2 - 2*a3*d4*de1*m6*cos(e2)^2 - 2*a3*d4*de1*m6*cos(e3)^2 - 4*I5xy*de1*cos(e2)^2*cos(e3)^2*cos(e4) - 4*I5xy*de1*cos(e2)^2*cos(e4)*cos(e5)^2 - 4*I5xy*de1*cos(e3)^2*cos(e4)*cos(e5)^2 + 4*I4zx*de1*cos(e2)^2*cos(e3)^2*cos(e4) - 2*a3*de1*m4*z4*cos(e2)^2 - 2*a3*de1*m4*z4*cos(e3)^2 - 4*I4yz*de1*cos(e2)^2*cos(e3)^2*sin(e4) + d4*de1*m4*z4*sin(2*e2) + d4*de1*m4*z4*sin(2*e3) + 2*de1*m2*x2*y2*cos(e2)^2 - 2*de1*m3*x3*y3*cos(e2)^2 - 2*de1*m3*x3*y3*cos(e3)^2 - (I6xx*de6*cos(e2)*cos(e3)*cos(e5))/2 - I4yz*de2*cos(e2)*cos(e3)*cos(e4) - I4yz*de3*cos(e2)*cos(e3)*cos(e4) + (I6yy*de6*cos(e2)*cos(e3)*cos(e5))/2 - (I6zz*de6*cos(e2)*cos(e3)*cos(e5))/2 + I5xy*de2*cos(e2)*cos(e3)*sin(e4) + I5xy*de3*cos(e2)*cos(e3)*sin(e4) - I6xy*de2*cos(e2)*cos(e5)*sin(e3) - I6xy*de2*cos(e3)*cos(e5)*sin(e2) - I5xx*de1*cos(e4)*cos(e5)*sin(e5) - I6xy*de3*cos(e2)*cos(e5)*sin(e3) - I6xy*de3*cos(e3)*cos(e5)*sin(e2) + I5yy*de1*cos(e4)*cos(e5)*sin(e5) - I6yy*de1*cos(e4)*cos(e5)*sin(e5) - I6yz*de1*cos(e5)*cos(e6)*sin(e4) - I4zx*de2*cos(e2)*cos(e3)*sin(e4) - I4zx*de3*cos(e2)*cos(e3)*sin(e4) - I5zx*de2*cos(e2)*cos(e5)*sin(e3) - I5zx*de2*cos(e3)*cos(e5)*sin(e2) - I5zx*de3*cos(e2)*cos(e5)*sin(e3) - I5zx*de3*cos(e3)*cos(e5)*sin(e2) + I6zz*de1*cos(e4)*cos(e5)*sin(e5) - (I5xx*de5*cos(e2)*sin(e3)*sin(e4))/2 - (I5xx*de5*cos(e3)*sin(e2)*sin(e4))/2 - (I6xx*de5*cos(e2)*sin(e3)*sin(e4))/2 - (I6xx*de5*cos(e3)*sin(e2)*sin(e4))/2 + (I6xx*de6*cos(e5)*sin(e2)*sin(e3))/2 + I4yz*de2*cos(e4)*sin(e2)*sin(e3) + I4yz*de3*cos(e4)*sin(e2)*sin(e3) + I5yz*de2*cos(e2)*sin(e3)*sin(e5) + I5yz*de2*cos(e3)*sin(e2)*sin(e5) + (I5yy*de5*cos(e2)*sin(e3)*sin(e4))/2 + (I5yy*de5*cos(e3)*sin(e2)*sin(e4))/2 + I5yz*de3*cos(e2)*sin(e3)*sin(e5) + I5yz*de3*cos(e3)*sin(e2)*sin(e5) - (I6yy*de5*cos(e2)*sin(e3)*sin(e4))/2 - (I6yy*de5*cos(e3)*sin(e2)*sin(e4))/2 - (I6yy*de6*cos(e5)*sin(e2)*sin(e3))/2 - (I5zz*de5*cos(e2)*sin(e3)*sin(e4))/2 - (I5zz*de5*cos(e3)*sin(e2)*sin(e4))/2 - I6zx*de1*cos(e5)*sin(e4)*sin(e6) + (I6zz*de5*cos(e2)*sin(e3)*sin(e4))/2 + (I6zz*de5*cos(e3)*sin(e2)*sin(e4))/2 + (I6zz*de6*cos(e5)*sin(e2)*sin(e3))/2 - I5xy*de2*sin(e2)*sin(e3)*sin(e4) - I5xy*de3*sin(e2)*sin(e3)*sin(e4) + I4zx*de2*sin(e2)*sin(e3)*sin(e4) + I4zx*de3*sin(e2)*sin(e3)*sin(e4) - de4*m4*x4^2*cos(e2)*cos(e3) - de4*m5*y5^2*cos(e2)*cos(e3) - de4*m6*z6^2*cos(e2)*cos(e3) + de4*m4*x4^2*sin(e2)*sin(e3) + de4*m5*y5^2*sin(e2)*sin(e3) + de4*m6*z6^2*sin(e2)*sin(e3) + a1*a2*de1*m3*cos(e2) + a1*a2*de1*m4*cos(e2) + a1*a2*de1*m5*cos(e2) + a1*a2*de1*m6*cos(e2) - a2*d4*de1*m4*cos(e3) - a2*d4*de1*m5*cos(e3) - a2*d4*de1*m6*cos(e3) - I4xx*de4*cos(e2)*cos(e3)*cos(e4)^2 + I5xx*de4*cos(e2)*cos(e3)*cos(e5)^2 + I6xx*de4*cos(e2)*cos(e3)*cos(e4)^2 + I4yy*de4*cos(e2)*cos(e3)*cos(e4)^2 - I5yy*de4*cos(e2)*cos(e3)*cos(e4)^2 - I5yy*de4*cos(e2)*cos(e3)*cos(e5)^2 + I6yy*de4*cos(e2)*cos(e3)*cos(e5)^2 + 2*I6zx*de1*cos(e2)^2*cos(e4)*cos(e6) + 2*I6zx*de1*cos(e3)^2*cos(e4)*cos(e6) + I5zz*de4*cos(e2)*cos(e3)*cos(e4)^2 - I6zz*de4*cos(e2)*cos(e3)*cos(e4)^2 + 2*I6zx*de1*cos(e4)*cos(e5)^2*cos(e6) - I6zz*de4*cos(e2)*cos(e3)*cos(e5)^2 - a2*a3*de1*m4*sin(e3) - a2*a3*de1*m5*sin(e3) - a2*a3*de1*m6*sin(e3) + a1*de1*m2*x2*cos(e2) - a2*de1*m3*y3*cos(e3) + a3*de1*m5*y5*cos(e5) - a2*de1*m4*z4*cos(e3) + a3*de1*m6*z6*cos(e5) + d4*de1*m4*x4*cos(e4) - 2*I3xx*de1*cos(e2)*cos(e3)^2*sin(e2) - 2*I3xx*de1*cos(e2)^2*cos(e3)*sin(e3) + I4xx*de1*cos(e2)*cos(e4)^2*sin(e2) + 2*I5xx*de1*cos(e2)*cos(e3)^2*sin(e2) + 2*I5xx*de1*cos(e2)^2*cos(e3)*sin(e3) - 2*I6xx*de1*cos(e2)*cos(e3)^2*sin(e2) + I4xx*de1*cos(e3)*cos(e4)^2*sin(e3) + I5xx*de1*cos(e2)*cos(e5)^2*sin(e2) - I6xx*de1*cos(e2)*cos(e4)^2*sin(e2) - 2*I6xx*de1*cos(e2)^2*cos(e3)*sin(e3) - 2*I4xy*de2*cos(e2)*cos(e4)^2*sin(e3) - 2*I4xy*de2*cos(e3)*cos(e4)^2*sin(e2) - 2*I4xy*de3*cos(e2)*cos(e4)^2*sin(e3) - 2*I4xy*de3*cos(e3)*cos(e4)^2*sin(e2) + I5xx*de1*cos(e3)*cos(e5)^2*sin(e3) - 2*I6xx*de1*cos(e2)*cos(e6)^2*sin(e2) - I6xx*de1*cos(e3)*cos(e4)^2*sin(e3) - 2*I6xx*de1*cos(e3)*cos(e6)^2*sin(e3) + 2*I3yy*de1*cos(e2)*cos(e3)^2*sin(e2) + 2*I3yy*de1*cos(e2)^2*cos(e3)*sin(e3) - 2*I4yy*de1*cos(e2)*cos(e3)^2*sin(e2) - I4yy*de1*cos(e2)*cos(e4)^2*sin(e2) - 2*I4yy*de1*cos(e2)^2*cos(e3)*sin(e3) + I5yy*de1*cos(e2)*cos(e4)^2*sin(e2) + 2*I6yy*de1*cos(e2)*cos(e3)^2*sin(e2) - I4yy*de1*cos(e3)*cos(e4)^2*sin(e3) - I5yy*de1*cos(e2)*cos(e5)^2*sin(e2) + 2*I6yy*de1*cos(e2)^2*cos(e3)*sin(e3) + I5yy*de1*cos(e3)*cos(e4)^2*sin(e3) + I6yy*de1*cos(e2)*cos(e5)^2*sin(e2) - I5yy*de1*cos(e3)*cos(e5)^2*sin(e3) + 2*I6yy*de1*cos(e2)*cos(e6)^2*sin(e2) - 2*I5yz*de1*cos(e2)^2*cos(e5)*sin(e4) + I6yy*de1*cos(e3)*cos(e5)^2*sin(e3) - 2*I5yz*de1*cos(e3)^2*cos(e5)*sin(e4) + 2*I6yy*de1*cos(e3)*cos(e6)^2*sin(e3) - 2*I6yz*de1*cos(e2)^2*cos(e4)*sin(e6) - 2*I6yz*de1*cos(e3)^2*cos(e4)*sin(e6) - 2*I6yz*de1*cos(e4)*cos(e5)^2*sin(e6) + 2*I4zz*de1*cos(e2)*cos(e3)^2*sin(e2) + 2*I4zz*de1*cos(e2)^2*cos(e3)*sin(e3) - 2*I5zz*de1*cos(e2)*cos(e3)^2*sin(e2) - I5zz*de1*cos(e2)*cos(e4)^2*sin(e2) - 2*I5zz*de1*cos(e2)^2*cos(e3)*sin(e3) + I6zz*de1*cos(e2)*cos(e4)^2*sin(e2) - I5zz*de1*cos(e3)*cos(e4)^2*sin(e3) - I6zz*de1*cos(e2)*cos(e5)^2*sin(e2) + I6zz*de1*cos(e3)*cos(e4)^2*sin(e3) - I6zz*de1*cos(e3)*cos(e5)^2*sin(e3) - a2*de1*m3*x3*sin(e3) + a3*de1*m5*x5*sin(e5) - a1*de1*m2*y2*sin(e2) + a2*de2*m3*z3*sin(e2) + I4xx*de4*cos(e4)^2*sin(e2)*sin(e3) - I5xx*de4*cos(e5)^2*sin(e2)*sin(e3) - I6xx*de4*cos(e4)^2*sin(e2)*sin(e3) - 2*I6xy*de1*cos(e2)^2*sin(e4)*sin(e5) - 2*I6xy*de1*cos(e3)^2*sin(e4)*sin(e5) - 2*I6xy*de1*cos(e6)^2*sin(e4)*sin(e5) - I4yy*de4*cos(e4)^2*sin(e2)*sin(e3) + I5yy*de4*cos(e4)^2*sin(e2)*sin(e3) + I5yy*de4*cos(e5)^2*sin(e2)*sin(e3) - I6yy*de4*cos(e5)^2*sin(e2)*sin(e3) - 2*I5zx*de1*cos(e2)^2*sin(e4)*sin(e5) - 2*I5zx*de1*cos(e3)^2*sin(e4)*sin(e5) - I5zz*de4*cos(e4)^2*sin(e2)*sin(e3) + I6zz*de4*cos(e4)^2*sin(e2)*sin(e3) + I6zz*de4*cos(e5)^2*sin(e2)*sin(e3) - d4*de1*m4*y4*sin(e4) + d4*de1*m5*z5*sin(e4) - de1*m5*x5*y5*cos(e4) + de1*m4*x4*z4*cos(e4) + de2*m2*y2*z2*cos(e2) + de2*m2*x2*z2*sin(e2) - de1*m4*y4*z4*sin(e4) + 2*a2*de1*m3*x3*cos(e2)^2*sin(e3) - 2*a3*de1*m5*x5*cos(e2)^2*sin(e5) - 2*a3*de1*m5*x5*cos(e3)^2*sin(e5) + 4*I6xy*de1*cos(e2)^2*cos(e3)^2*sin(e4)*sin(e5) + I5xx*de4*cos(e4)^2*cos(e5)^2*sin(e2)*sin(e3) + I6xx*de4*cos(e4)^2*cos(e6)^2*sin(e2)*sin(e3) + 4*I6xy*de1*cos(e2)^2*cos(e6)^2*sin(e4)*sin(e5) - I6xx*de4*cos(e5)^2*cos(e6)^2*sin(e2)*sin(e3) + 4*I6xy*de1*cos(e3)^2*cos(e6)^2*sin(e4)*sin(e5) - I5yy*de4*cos(e4)^2*cos(e5)^2*sin(e2)*sin(e3) + I6yy*de4*cos(e4)^2*cos(e5)^2*sin(e2)*sin(e3) - I6yy*de4*cos(e4)^2*cos(e6)^2*sin(e2)*sin(e3) + I6yy*de4*cos(e5)^2*cos(e6)^2*sin(e2)*sin(e3) + 4*I5zx*de1*cos(e2)^2*cos(e3)^2*sin(e4)*sin(e5) - I6zz*de4*cos(e4)^2*cos(e5)^2*sin(e2)*sin(e3) + 2*d4*de1*m4*y4*cos(e2)^2*sin(e4) + 2*d4*de1*m4*y4*cos(e3)^2*sin(e4) - 2*d4*de1*m5*z5*cos(e2)^2*sin(e4) - 2*d4*de1*m5*z5*cos(e3)^2*sin(e4) + 2*de1*m5*x5*y5*cos(e2)^2*cos(e4) + 2*de1*m5*x5*y5*cos(e3)^2*cos(e4) + 2*de1*m5*x5*y5*cos(e4)*cos(e5)^2 - 2*de1*m4*x4*z4*cos(e2)^2*cos(e4) - 2*de1*m4*x4*z4*cos(e3)^2*cos(e4) + 2*de1*m4*y4*z4*cos(e2)^2*sin(e4) + 2*de1*m4*y4*z4*cos(e3)^2*sin(e4) + I5yz*de2*cos(e2)*cos(e3)*cos(e4)*cos(e5) + I5yz*de3*cos(e2)*cos(e3)*cos(e4)*cos(e5) - 2*I4xy*de4*cos(e2)*cos(e3)*cos(e4)*sin(e4) + I6xy*de2*cos(e2)*cos(e3)*cos(e4)*sin(e5) + I5xy*de5*cos(e2)*cos(e3)*cos(e4)*sin(e4) + I6xy*de3*cos(e2)*cos(e3)*cos(e4)*sin(e5) + 2*I5xy*de4*cos(e2)*cos(e3)*cos(e5)*sin(e5) + I6xy*de5*cos(e2)*cos(e4)*cos(e5)*sin(e3) + I6xy*de5*cos(e3)*cos(e4)*cos(e5)*sin(e2) + I6xy*de6*cos(e2)*cos(e3)*cos(e4)*sin(e4) + I5zx*de2*cos(e2)*cos(e3)*cos(e4)*sin(e5) + I5zx*de3*cos(e2)*cos(e3)*cos(e4)*sin(e5) + I6zx*de2*cos(e2)*cos(e3)*cos(e6)*sin(e4) + I5zx*de5*cos(e2)*cos(e4)*cos(e5)*sin(e3) + I5zx*de5*cos(e3)*cos(e4)*cos(e5)*sin(e2) + I6zx*de3*cos(e2)*cos(e3)*cos(e6)*sin(e4) + I6zx*de6*cos(e2)*cos(e3)*cos(e6)*sin(e5) + 4*a3*d4*de1*m4*cos(e2)^2*cos(e3)^2 + 4*a3*d4*de1*m5*cos(e2)^2*cos(e3)^2 + 4*a3*d4*de1*m6*cos(e2)^2*cos(e3)^2 + 8*I5xy*de1*cos(e2)^2*cos(e3)^2*cos(e4)*cos(e5)^2 - 4*I3xy*de1*cos(e2)*cos(e3)*sin(e2)*sin(e3) + 2*I4xy*de1*cos(e2)*cos(e4)*sin(e2)*sin(e4) + I4xx*de2*cos(e2)*cos(e4)*sin(e3)*sin(e4) + I4xx*de2*cos(e3)*cos(e4)*sin(e2)*sin(e4) + I4xx*de3*cos(e2)*cos(e4)*sin(e3)*sin(e4) + I4xx*de3*cos(e3)*cos(e4)*sin(e2)*sin(e4) + 2*I4xy*de1*cos(e3)*cos(e4)*sin(e3)*sin(e4) + 2*I5xy*de1*cos(e2)*cos(e5)*sin(e2)*sin(e5) - I6xx*de2*cos(e2)*cos(e4)*sin(e3)*sin(e4) - I6xx*de2*cos(e3)*cos(e4)*sin(e2)*sin(e4) - I6xx*de3*cos(e2)*cos(e4)*sin(e3)*sin(e4) - I6xx*de3*cos(e3)*cos(e4)*sin(e2)*sin(e4) + 2*I5xy*de1*cos(e3)*cos(e5)*sin(e3)*sin(e5) - 4*I6xy*de1*cos(e2)*cos(e6)*sin(e2)*sin(e6) - (I6xx*de6*cos(e2)*cos(e4)*sin(e3)*sin(e5))/2 - (I6xx*de6*cos(e3)*cos(e4)*sin(e2)*sin(e5))/2 - 4*I6xy*de1*cos(e3)*cos(e6)*sin(e3)*sin(e6) - I4yy*de2*cos(e2)*cos(e4)*sin(e3)*sin(e4) - I4yy*de2*cos(e3)*cos(e4)*sin(e2)*sin(e4) - I4yy*de3*cos(e2)*cos(e4)*sin(e3)*sin(e4) - I4yy*de3*cos(e3)*cos(e4)*sin(e2)*sin(e4) + I5yy*de2*cos(e2)*cos(e4)*sin(e3)*sin(e4) + I5yy*de2*cos(e3)*cos(e4)*sin(e2)*sin(e4) + I5yy*de3*cos(e2)*cos(e4)*sin(e3)*sin(e4) + I5yy*de3*cos(e3)*cos(e4)*sin(e2)*sin(e4) - I5yz*de2*cos(e4)*cos(e5)*sin(e2)*sin(e3) - I5yz*de3*cos(e4)*cos(e5)*sin(e2)*sin(e3) - I6yz*de2*cos(e2)*cos(e3)*sin(e4)*sin(e6) - I5yz*de5*cos(e2)*cos(e4)*sin(e3)*sin(e5) - I5yz*de5*cos(e3)*cos(e4)*sin(e2)*sin(e5) - I6yz*de2*cos(e2)*cos(e6)*sin(e3)*sin(e5) - I6yz*de2*cos(e3)*cos(e6)*sin(e2)*sin(e5) - I6yz*de3*cos(e2)*cos(e3)*sin(e4)*sin(e6) + (I6yy*de6*cos(e2)*cos(e4)*sin(e3)*sin(e5))/2 + (I6yy*de6*cos(e3)*cos(e4)*sin(e2)*sin(e5))/2 - I6yz*de3*cos(e2)*cos(e6)*sin(e3)*sin(e5) - I6yz*de3*cos(e3)*cos(e6)*sin(e2)*sin(e5) - I6yz*de6*cos(e2)*cos(e6)*sin(e3)*sin(e4) - I6yz*de6*cos(e3)*cos(e6)*sin(e2)*sin(e4) - I6yz*de6*cos(e2)*cos(e3)*sin(e5)*sin(e6) - I5zz*de2*cos(e2)*cos(e4)*sin(e3)*sin(e4) - I5zz*de2*cos(e3)*cos(e4)*sin(e2)*sin(e4) - I5zz*de3*cos(e2)*cos(e4)*sin(e3)*sin(e4) - I5zz*de3*cos(e3)*cos(e4)*sin(e2)*sin(e4) + I6zz*de2*cos(e2)*cos(e4)*sin(e3)*sin(e4) + I6zz*de2*cos(e3)*cos(e4)*sin(e2)*sin(e4) + I6zz*de3*cos(e2)*cos(e4)*sin(e3)*sin(e4) + I6zz*de3*cos(e3)*cos(e4)*sin(e2)*sin(e4) + (I6zz*de6*cos(e2)*cos(e4)*sin(e3)*sin(e5))/2 + (I6zz*de6*cos(e3)*cos(e4)*sin(e2)*sin(e5))/2 + 4*a3*de1*m4*z4*cos(e2)^2*cos(e3)^2 + 2*I4xy*de4*cos(e4)*sin(e2)*sin(e3)*sin(e4) - I6xy*de2*cos(e4)*sin(e2)*sin(e3)*sin(e5) - I5xy*de5*cos(e4)*sin(e2)*sin(e3)*sin(e4) - I6xy*de3*cos(e4)*sin(e2)*sin(e3)*sin(e5) - 2*I5xy*de4*cos(e5)*sin(e2)*sin(e3)*sin(e5) - I6xy*de6*cos(e4)*sin(e2)*sin(e3)*sin(e4) + I6xx*de1*cos(e6)*sin(e4)*sin(e5)*sin(e6) - I6yy*de1*cos(e6)*sin(e4)*sin(e5)*sin(e6) - I5zx*de2*cos(e4)*sin(e2)*sin(e3)*sin(e5) - I5zx*de3*cos(e4)*sin(e2)*sin(e3)*sin(e5) - I6zx*de2*cos(e6)*sin(e2)*sin(e3)*sin(e4) - I6zx*de2*cos(e2)*sin(e3)*sin(e5)*sin(e6) - I6zx*de2*cos(e3)*sin(e2)*sin(e5)*sin(e6) - I6zx*de3*cos(e6)*sin(e2)*sin(e3)*sin(e4) - I6zx*de3*cos(e2)*sin(e3)*sin(e5)*sin(e6) - I6zx*de3*cos(e3)*sin(e2)*sin(e5)*sin(e6) - I6zx*de6*cos(e2)*sin(e3)*sin(e4)*sin(e6) - I6zx*de6*cos(e3)*sin(e2)*sin(e4)*sin(e6) - I6zx*de6*cos(e6)*sin(e2)*sin(e3)*sin(e5) - de6*m6*y6^2*cos(e2)*cos(e3)*cos(e5) + I6yz*de2*sin(e2)*sin(e3)*sin(e4)*sin(e6) + I6yz*de3*sin(e2)*sin(e3)*sin(e4)*sin(e6) + I6yz*de6*sin(e2)*sin(e3)*sin(e5)*sin(e6) + de1*m5*x5^2*cos(e4)*cos(e5)*sin(e5) + 4*de1*m3*x3*y3*cos(e2)^2*cos(e3)^2 - de1*m5*y5^2*cos(e4)*cos(e5)*sin(e5) + de1*m6*y6^2*cos(e4)*cos(e5)*sin(e5) - de1*m6*z6^2*cos(e4)*cos(e5)*sin(e5) - de5*m5*y5^2*cos(e2)*sin(e3)*sin(e4) - de5*m5*y5^2*cos(e3)*sin(e2)*sin(e4) + de6*m6*y6^2*cos(e5)*sin(e2)*sin(e3) - de5*m6*z6^2*cos(e2)*sin(e3)*sin(e4) - de5*m6*z6^2*cos(e3)*sin(e2)*sin(e4) + a1*a3*de1*m4*cos(e2)*cos(e3) + a1*a3*de1*m5*cos(e2)*cos(e3) + a1*a3*de1*m6*cos(e2)*cos(e3) + I6xx*de6*cos(e2)*cos(e3)*cos(e4)^2*cos(e5) + I6xx*de6*cos(e2)*cos(e3)*cos(e5)*cos(e6)^2 + I5yz*de5*cos(e2)*cos(e3)*cos(e4)^2*cos(e5) - I6yy*de6*cos(e2)*cos(e3)*cos(e4)^2*cos(e5) - I6yy*de6*cos(e2)*cos(e3)*cos(e5)*cos(e6)^2 - a1*d4*de1*m4*cos(e2)*sin(e3) - a1*d4*de1*m4*cos(e3)*sin(e2) - a1*d4*de1*m5*cos(e2)*sin(e3) - a1*d4*de1*m5*cos(e3)*sin(e2) - a1*d4*de1*m6*cos(e2)*sin(e3) - a1*d4*de1*m6*cos(e3)*sin(e2) + a1*de1*m3*x3*cos(e2)*cos(e3) - a2*de1*m5*y5*cos(e3)*cos(e5) - a2*de1*m6*z6*cos(e3)*cos(e5) + d4*de1*m5*x5*cos(e4)*cos(e5) + 2*I5xx*de1*cos(e2)^2*cos(e4)*cos(e5)*sin(e5) - 2*I5xy*de2*cos(e2)*cos(e3)*cos(e5)^2*sin(e4) + 2*I5xx*de1*cos(e3)^2*cos(e4)*cos(e5)*sin(e5) - 2*I5xy*de3*cos(e2)*cos(e3)*cos(e5)^2*sin(e4) + 2*I6xy*de2*cos(e2)*cos(e4)^2*cos(e5)*sin(e3) + 2*I6xy*de2*cos(e3)*cos(e4)^2*cos(e5)*sin(e2) + 2*I6xy*de3*cos(e2)*cos(e4)^2*cos(e5)*sin(e3) + 2*I6xy*de3*cos(e3)*cos(e4)^2*cos(e5)*sin(e2) + 2*I6xy*de2*cos(e2)*cos(e5)*cos(e6)^2*sin(e3) + 2*I6xy*de2*cos(e3)*cos(e5)*cos(e6)^2*sin(e2) + 2*I6xy*de3*cos(e2)*cos(e5)*cos(e6)^2*sin(e3) + 2*I6xy*de3*cos(e3)*cos(e5)*cos(e6)^2*sin(e2) + I6xy*de5*cos(e2)*cos(e3)*cos(e4)^2*sin(e5) - I6xx*de1*cos(e4)*cos(e5)*cos(e6)^2*sin(e5) - 2*I5yy*de1*cos(e2)^2*cos(e4)*cos(e5)*sin(e5) - 2*I5yy*de1*cos(e3)^2*cos(e4)*cos(e5)*sin(e5) + 2*I6yy*de1*cos(e2)^2*cos(e4)*cos(e5)*sin(e5) + 2*I6yy*de1*cos(e3)^2*cos(e4)*cos(e5)*sin(e5) + 2*I6yz*de1*cos(e2)^2*cos(e5)*cos(e6)*sin(e4) + 2*I6yz*de1*cos(e3)^2*cos(e5)*cos(e6)*sin(e4) + I6yy*de1*cos(e4)*cos(e5)*cos(e6)^2*sin(e5) + 2*I5zx*de2*cos(e2)*cos(e4)^2*cos(e5)*sin(e3) + 2*I5zx*de2*cos(e3)*cos(e4)^2*cos(e5)*sin(e2) + 2*I5zx*de3*cos(e2)*cos(e4)^2*cos(e5)*sin(e3) + 2*I5zx*de3*cos(e3)*cos(e4)^2*cos(e5)*sin(e2) + I5zx*de5*cos(e2)*cos(e3)*cos(e4)^2*sin(e5) - 2*I6zz*de1*cos(e2)^2*cos(e4)*cos(e5)*sin(e5) - 2*I6zz*de1*cos(e3)^2*cos(e4)*cos(e5)*sin(e5) - a1*a3*de1*m4*sin(e2)*sin(e3) - a1*a3*de1*m5*sin(e2)*sin(e3) - a1*a3*de1*m6*sin(e2)*sin(e3) - a2*de1*m4*x4*cos(e4)*sin(e3) - a2*de1*m5*x5*cos(e3)*sin(e5) + a3*de1*m6*x6*cos(e6)*sin(e5) - a1*de1*m3*y3*cos(e2)*sin(e3) - a1*de1*m3*y3*cos(e3)*sin(e2) - a2*de2*m4*y4*cos(e4)*sin(e2) - a1*de1*m4*z4*cos(e2)*sin(e3) - a1*de1*m4*z4*cos(e3)*sin(e2) + a2*de2*m5*z5*cos(e4)*sin(e2) + I5xx*de5*cos(e2)*cos(e5)^2*sin(e3)*sin(e4) + I5xx*de5*cos(e3)*cos(e5)^2*sin(e2)*sin(e4) - I6xx*de6*cos(e4)^2*cos(e5)*sin(e2)*sin(e3) - I6xx*de6*cos(e5)*cos(e6)^2*sin(e2)*sin(e3) - 2*I5yz*de2*cos(e2)*cos(e4)^2*sin(e3)*sin(e5) - 2*I5yz*de2*cos(e3)*cos(e4)^2*sin(e2)*sin(e5) - 2*I5yz*de3*cos(e2)*cos(e4)^2*sin(e3)*sin(e5) - 2*I5yz*de3*cos(e3)*cos(e4)^2*sin(e2)*sin(e5) - I5yy*de5*cos(e2)*cos(e5)^2*sin(e3)*sin(e4) - I5yy*de5*cos(e3)*cos(e5)^2*sin(e2)*sin(e4) - I5yz*de5*cos(e4)^2*cos(e5)*sin(e2)*sin(e3) + I6yy*de5*cos(e2)*cos(e5)^2*sin(e3)*sin(e4) + I6yy*de5*cos(e3)*cos(e5)^2*sin(e2)*sin(e4) + I6yy*de6*cos(e4)^2*cos(e5)*sin(e2)*sin(e3) + I6yy*de6*cos(e5)*cos(e6)^2*sin(e2)*sin(e3) + 2*I6zx*de1*cos(e2)^2*cos(e5)*sin(e4)*sin(e6) + 2*I6zx*de1*cos(e3)^2*cos(e5)*sin(e4)*sin(e6) - I6zz*de5*cos(e2)*cos(e5)^2*sin(e3)*sin(e4) - I6zz*de5*cos(e3)*cos(e5)^2*sin(e2)*sin(e4) - d4*de1*m5*y5*cos(e4)*sin(e5) - d4*de1*m6*y6*cos(e6)*sin(e4) - d4*de1*m6*z6*cos(e4)*sin(e5) - de1*m6*x6*z6*cos(e4)*cos(e6) + de2*m3*y3*z3*cos(e2)*cos(e3) + de3*m3*y3*z3*cos(e2)*cos(e3) + 2*a3^2*de1*m4*cos(e2)*cos(e3)^2*sin(e2) + 2*a3^2*de1*m4*cos(e2)^2*cos(e3)*sin(e3) + 2*a3^2*de1*m5*cos(e2)*cos(e3)^2*sin(e2) + 2*a3^2*de1*m5*cos(e2)^2*cos(e3)*sin(e3) + 2*a3^2*de1*m6*cos(e2)*cos(e3)^2*sin(e2) + 2*a3^2*de1*m6*cos(e2)^2*cos(e3)*sin(e3) - a1*de1*m3*x3*sin(e2)*sin(e3) - a2*de2*m4*x4*sin(e2)*sin(e4) + a2*de1*m4*y4*sin(e3)*sin(e4) - a3*de1*m6*y6*sin(e5)*sin(e6) - a2*de1*m5*z5*sin(e3)*sin(e4) - 2*d4^2*de1*m4*cos(e2)*cos(e3)^2*sin(e2) - 2*d4^2*de1*m4*cos(e2)^2*cos(e3)*sin(e3) - 2*d4^2*de1*m5*cos(e2)*cos(e3)^2*sin(e2) - 2*d4^2*de1*m5*cos(e2)^2*cos(e3)*sin(e3) - 2*d4^2*de1*m6*cos(e2)*cos(e3)^2*sin(e2) - 2*d4^2*de1*m6*cos(e2)^2*cos(e3)*sin(e3) - d4*de1*m6*x6*sin(e4)*sin(e6) + 2*I5xy*de2*cos(e5)^2*sin(e2)*sin(e3)*sin(e4) + 2*I5xy*de3*cos(e5)^2*sin(e2)*sin(e3)*sin(e4) - I6xy*de5*cos(e4)^2*sin(e2)*sin(e3)*sin(e5) - I5zx*de5*cos(e4)^2*sin(e2)*sin(e3)*sin(e5) + de4*m4*x4^2*cos(e2)*cos(e3)*cos(e4)^2 - de4*m5*x5^2*cos(e2)*cos(e3)*cos(e5)^2 - de4*m6*x6^2*cos(e2)*cos(e3)*cos(e4)^2 - de4*m4*y4^2*cos(e2)*cos(e3)*cos(e4)^2 + de4*m5*y5^2*cos(e2)*cos(e3)*cos(e4)^2 + de4*m5*y5^2*cos(e2)*cos(e3)*cos(e5)^2 - de4*m6*y6^2*cos(e2)*cos(e3)*cos(e5)^2 + de2*m4*x4*y4*cos(e2)*sin(e3) + de2*m4*x4*y4*cos(e3)*sin(e2) + de3*m4*x4*y4*cos(e2)*sin(e3) + de3*m4*x4*y4*cos(e3)*sin(e2) - de4*m5*z5^2*cos(e2)*cos(e3)*cos(e4)^2 + de4*m6*z6^2*cos(e2)*cos(e3)*cos(e4)^2 + de4*m6*z6^2*cos(e2)*cos(e3)*cos(e5)^2 + de2*m3*x3*z3*cos(e2)*sin(e3) + de2*m3*x3*z3*cos(e3)*sin(e2) + de3*m3*x3*z3*cos(e2)*sin(e3) + de3*m3*x3*z3*cos(e3)*sin(e2) + de1*m5*y5*z5*cos(e5)*sin(e4) + de1*m6*y6*z6*cos(e4)*sin(e6) + 2*de1*m3*x3^2*cos(e2)*cos(e3)^2*sin(e2) + 2*de1*m3*x3^2*cos(e2)^2*cos(e3)*sin(e3) - de1*m4*x4^2*cos(e2)*cos(e4)^2*sin(e2) - 2*de1*m5*x5^2*cos(e2)*cos(e3)^2*sin(e2) - de1*m4*x4^2*cos(e3)*cos(e4)^2*sin(e3) - 2*de1*m5*x5^2*cos(e2)^2*cos(e3)*sin(e3) - de1*m5*x5^2*cos(e2)*cos(e5)^2*sin(e2) + 2*de1*m6*x6^2*cos(e2)*cos(e3)^2*sin(e2) + de1*m6*x6^2*cos(e2)*cos(e4)^2*sin(e2) + 2*de1*m6*x6^2*cos(e2)^2*cos(e3)*sin(e3) - de1*m5*x5^2*cos(e3)*cos(e5)^2*sin(e3) + 2*de1*m6*x6^2*cos(e2)*cos(e6)^2*sin(e2) + de1*m6*x6^2*cos(e3)*cos(e4)^2*sin(e3) + 2*de1*m6*x6^2*cos(e3)*cos(e6)^2*sin(e3) - 2*de1*m3*y3^2*cos(e2)*cos(e3)^2*sin(e2) - 2*de1*m3*y3^2*cos(e2)^2*cos(e3)*sin(e3) + 2*de1*m4*y4^2*cos(e2)*cos(e3)^2*sin(e2) + de1*m4*y4^2*cos(e2)*cos(e4)^2*sin(e2) + 2*de1*m4*y4^2*cos(e2)^2*cos(e3)*sin(e3) + de1*m4*y4^2*cos(e3)*cos(e4)^2*sin(e3) - de1*m5*y5^2*cos(e2)*cos(e4)^2*sin(e2) + de1*m5*y5^2*cos(e2)*cos(e5)^2*sin(e2) - 2*de1*m6*y6^2*cos(e2)*cos(e3)^2*sin(e2) - de1*m5*y5^2*cos(e3)*cos(e4)^2*sin(e3) - 2*de1*m6*y6^2*cos(e2)^2*cos(e3)*sin(e3) + de1*m5*y5^2*cos(e3)*cos(e5)^2*sin(e3) - de1*m6*y6^2*cos(e2)*cos(e5)^2*sin(e2) - 2*de1*m6*y6^2*cos(e2)*cos(e6)^2*sin(e2) - de1*m6*y6^2*cos(e3)*cos(e5)^2*sin(e3) - 2*de1*m6*y6^2*cos(e3)*cos(e6)^2*sin(e3) + de1*m6*x6*y6*sin(e4)*sin(e5) - 2*de1*m4*z4^2*cos(e2)*cos(e3)^2*sin(e2) - 2*de1*m4*z4^2*cos(e2)^2*cos(e3)*sin(e3) + 2*de1*m5*z5^2*cos(e2)*cos(e3)^2*sin(e2) + de1*m5*z5^2*cos(e2)*cos(e4)^2*sin(e2) + 2*de1*m5*z5^2*cos(e2)^2*cos(e3)*sin(e3) + de1*m5*z5^2*cos(e3)*cos(e4)^2*sin(e3) - de1*m6*z6^2*cos(e2)*cos(e4)^2*sin(e2) + de1*m6*z6^2*cos(e2)*cos(e5)^2*sin(e2) - de1*m6*z6^2*cos(e3)*cos(e4)^2*sin(e3) + de1*m6*z6^2*cos(e3)*cos(e5)^2*sin(e3) + de1*m5*x5*z5*sin(e4)*sin(e5) - de2*m3*y3*z3*sin(e2)*sin(e3) - de3*m3*y3*z3*sin(e2)*sin(e3) - de4*m4*x4^2*cos(e4)^2*sin(e2)*sin(e3) + de4*m5*x5^2*cos(e5)^2*sin(e2)*sin(e3) + de4*m6*x6^2*cos(e4)^2*sin(e2)*sin(e3) + de4*m4*y4^2*cos(e4)^2*sin(e2)*sin(e3) - de4*m5*y5^2*cos(e4)^2*sin(e2)*sin(e3) - de4*m5*y5^2*cos(e5)^2*sin(e2)*sin(e3) + de4*m6*y6^2*cos(e5)^2*sin(e2)*sin(e3) + de4*m5*z5^2*cos(e4)^2*sin(e2)*sin(e3) - de4*m6*z6^2*cos(e4)^2*sin(e2)*sin(e3) - de4*m6*z6^2*cos(e5)^2*sin(e2)*sin(e3) + 2*a2*d4*de1*m4*cos(e2)^2*cos(e3) + 2*a2*d4*de1*m5*cos(e2)^2*cos(e3) + 2*a2*d4*de1*m6*cos(e2)^2*cos(e3) - I5xx*de4*cos(e2)*cos(e3)*cos(e4)^2*cos(e5)^2 - I6xx*de4*cos(e2)*cos(e3)*cos(e4)^2*cos(e6)^2 + I6xx*de4*cos(e2)*cos(e3)*cos(e5)^2*cos(e6)^2 + I5yy*de4*cos(e2)*cos(e3)*cos(e4)^2*cos(e5)^2 - I6yy*de4*cos(e2)*cos(e3)*cos(e4)^2*cos(e5)^2 + I6yy*de4*cos(e2)*cos(e3)*cos(e4)^2*cos(e6)^2 - I6yy*de4*cos(e2)*cos(e3)*cos(e5)^2*cos(e6)^2 - 4*I6zx*de1*cos(e2)^2*cos(e3)^2*cos(e4)*cos(e6) - 4*I6zx*de1*cos(e2)^2*cos(e4)*cos(e5)^2*cos(e6) - 4*I6zx*de1*cos(e3)^2*cos(e4)*cos(e5)^2*cos(e6) + I6zz*de4*cos(e2)*cos(e3)*cos(e4)^2*cos(e5)^2 + 2*a2*a3*de1*m4*cos(e2)^2*sin(e3) + 2*a2*a3*de1*m5*cos(e2)^2*sin(e3) + 2*a2*a3*de1*m6*cos(e2)^2*sin(e3) + 2*a2*de1*m3*y3*cos(e2)^2*cos(e3) - 2*a3*de1*m5*y5*cos(e2)^2*cos(e5) - 2*a3*de1*m5*y5*cos(e3)^2*cos(e5) + 2*a2*de1*m4*z4*cos(e2)^2*cos(e3) - 2*a3*de1*m6*z6*cos(e2)^2*cos(e5) - 2*a3*de1*m6*z6*cos(e3)^2*cos(e5) - 2*d4*de1*m4*x4*cos(e2)^2*cos(e4) - 2*d4*de1*m4*x4*cos(e3)^2*cos(e4) - 2*I4xx*de1*cos(e2)*cos(e3)^2*cos(e4)^2*sin(e2) - 2*I4xx*de1*cos(e2)^2*cos(e3)*cos(e4)^2*sin(e3) - 2*I5xx*de1*cos(e2)*cos(e3)^2*cos(e5)^2*sin(e2) + 2*I6xx*de1*cos(e2)*cos(e3)^2*cos(e4)^2*sin(e2) + I5xx*de1*cos(e2)*cos(e4)^2*cos(e5)^2*sin(e2) - 2*I5xx*de1*cos(e2)^2*cos(e3)*cos(e5)^2*sin(e3) + 2*I6xx*de1*cos(e2)^2*cos(e3)*cos(e4)^2*sin(e3) + 4*I6xx*de1*cos(e2)*cos(e3)^2*cos(e6)^2*sin(e2) + I5xx*de1*cos(e3)*cos(e4)^2*cos(e5)^2*sin(e3) + I6xx*de1*cos(e2)*cos(e4)^2*cos(e6)^2*sin(e2) + 4*I6xx*de1*cos(e2)^2*cos(e3)*cos(e6)^2*sin(e3) + I6xx*de1*cos(e2)*cos(e5)^2*cos(e6)^2*sin(e2) + I6xx*de1*cos(e3)*cos(e4)^2*cos(e6)^2*sin(e3) + I6xx*de1*cos(e3)*cos(e5)^2*cos(e6)^2*sin(e3) + 2*I4yy*de1*cos(e2)*cos(e3)^2*cos(e4)^2*sin(e2) + 2*I4yy*de1*cos(e2)^2*cos(e3)*cos(e4)^2*sin(e3) - 2*I5yy*de1*cos(e2)*cos(e3)^2*cos(e4)^2*sin(e2) + 2*I5yy*de1*cos(e2)*cos(e3)^2*cos(e5)^2*sin(e2) - 2*I5yy*de1*cos(e2)^2*cos(e3)*cos(e4)^2*sin(e3) - I5yy*de1*cos(e2)*cos(e4)^2*cos(e5)^2*sin(e2) + 2*I5yy*de1*cos(e2)^2*cos(e3)*cos(e5)^2*sin(e3) - 2*I6yy*de1*cos(e2)*cos(e3)^2*cos(e5)^2*sin(e2) - 4*I6yy*de1*cos(e2)*cos(e3)^2*cos(e6)^2*sin(e2) + I6yy*de1*cos(e2)*cos(e4)^2*cos(e5)^2*sin(e2) - 2*I6yy*de1*cos(e2)^2*cos(e3)*cos(e5)^2*sin(e3) - I5yy*de1*cos(e3)*cos(e4)^2*cos(e5)^2*sin(e3) + 4*I5yz*de1*cos(e2)^2*cos(e3)^2*cos(e5)*sin(e4) - I6yy*de1*cos(e2)*cos(e4)^2*cos(e6)^2*sin(e2) - 4*I6yy*de1*cos(e2)^2*cos(e3)*cos(e6)^2*sin(e3) - I6yy*de1*cos(e2)*cos(e5)^2*cos(e6)^2*sin(e2) + I6yy*de1*cos(e3)*cos(e4)^2*cos(e5)^2*sin(e3) - I6yy*de1*cos(e3)*cos(e4)^2*cos(e6)^2*sin(e3) + 4*I6yz*de1*cos(e2)^2*cos(e3)^2*cos(e4)*sin(e6) - I6yy*de1*cos(e3)*cos(e5)^2*cos(e6)^2*sin(e3) + 4*I6yz*de1*cos(e2)^2*cos(e4)*cos(e5)^2*sin(e6) + 4*I6yz*de1*cos(e3)^2*cos(e4)*cos(e5)^2*sin(e6) + 2*I5zz*de1*cos(e2)*cos(e3)^2*cos(e4)^2*sin(e2) + 2*I5zz*de1*cos(e2)^2*cos(e3)*cos(e4)^2*sin(e3) - 2*I6zz*de1*cos(e2)*cos(e3)^2*cos(e4)^2*sin(e2) + 2*I6zz*de1*cos(e2)*cos(e3)^2*cos(e5)^2*sin(e2) - 2*I6zz*de1*cos(e2)^2*cos(e3)*cos(e4)^2*sin(e3) - I6zz*de1*cos(e2)*cos(e4)^2*cos(e5)^2*sin(e2) + 2*I6zz*de1*cos(e2)^2*cos(e3)*cos(e5)^2*sin(e3) - I6zz*de1*cos(e3)*cos(e4)^2*cos(e5)^2*sin(e3) + 2*I6xy*de4*cos(e2)*cos(e3)*cos(e4)*cos(e5)*sin(e4) + 2*I6xy*de6*cos(e2)*cos(e3)*cos(e5)*cos(e6)*sin(e6) + 2*I5zx*de4*cos(e2)*cos(e3)*cos(e4)*cos(e5)*sin(e4) - I6zx*de2*cos(e2)*cos(e3)*cos(e4)*cos(e5)*sin(e6) - I6zx*de3*cos(e2)*cos(e3)*cos(e4)*cos(e5)*sin(e6) + I6zx*de5*cos(e2)*cos(e3)*cos(e4)*cos(e6)*sin(e4) + 2*I6zx*de4*cos(e2)*cos(e3)*cos(e5)*cos(e6)*sin(e5) - de4*m5*x5^2*cos(e4)^2*cos(e5)^2*sin(e2)*sin(e3) - de4*m6*x6^2*cos(e4)^2*cos(e6)^2*sin(e2)*sin(e3) + de4*m6*x6^2*cos(e5)^2*cos(e6)^2*sin(e2)*sin(e3) + de4*m5*y5^2*cos(e4)^2*cos(e5)^2*sin(e2)*sin(e3) - de4*m6*y6^2*cos(e4)^2*cos(e5)^2*sin(e2)*sin(e3) + de4*m6*y6^2*cos(e4)^2*cos(e6)^2*sin(e2)*sin(e3) - de4*m6*y6^2*cos(e5)^2*cos(e6)^2*sin(e2)*sin(e3) + de4*m6*z6^2*cos(e4)^2*cos(e5)^2*sin(e2)*sin(e3) - I6xx*de4*cos(e2)*cos(e3)*cos(e4)^2*cos(e5)^2*cos(e6)^2 + I6yy*de4*cos(e2)*cos(e3)*cos(e4)^2*cos(e5)^2*cos(e6)^2 + 8*I6zx*de1*cos(e2)^2*cos(e3)^2*cos(e4)*cos(e5)^2*cos(e6) + 4*I5xy*de1*cos(e2)*cos(e3)*cos(e4)*sin(e2)*sin(e3) - 2*I6xy*de1*cos(e2)*cos(e4)*cos(e5)*sin(e2)*sin(e4) + I5xx*de2*cos(e2)*cos(e3)*cos(e5)*sin(e4)*sin(e5) + I5xx*de3*cos(e2)*cos(e3)*cos(e5)*sin(e4)*sin(e5) - 2*I6xy*de1*cos(e3)*cos(e4)*cos(e5)*sin(e3)*sin(e4) - I6xx*de2*cos(e2)*cos(e5)*cos(e6)*sin(e3)*sin(e6) - I6xx*de2*cos(e3)*cos(e5)*cos(e6)*sin(e2)*sin(e6) - I6xx*de3*cos(e2)*cos(e5)*cos(e6)*sin(e3)*sin(e6) - I6xx*de3*cos(e3)*cos(e5)*cos(e6)*sin(e2)*sin(e6) - 2*I6xy*de1*cos(e4)*cos(e5)*cos(e6)*sin(e5)*sin(e6) - I5yy*de2*cos(e2)*cos(e3)*cos(e5)*sin(e4)*sin(e5) - I5yy*de3*cos(e2)*cos(e3)*cos(e5)*sin(e4)*sin(e5) + I6yy*de2*cos(e2)*cos(e3)*cos(e5)*sin(e4)*sin(e5) - 2*I5yz*de4*cos(e2)*cos(e3)*cos(e4)*sin(e4)*sin(e5) + I6yy*de3*cos(e2)*cos(e3)*cos(e5)*sin(e4)*sin(e5) + I6yz*de2*cos(e4)*cos(e5)*cos(e6)*sin(e2)*sin(e3) + I6yy*de2*cos(e2)*cos(e5)*cos(e6)*sin(e3)*sin(e6) + I6yy*de2*cos(e3)*cos(e5)*cos(e6)*sin(e2)*sin(e6) + I6yz*de3*cos(e4)*cos(e5)*cos(e6)*sin(e2)*sin(e3) + I6yy*de3*cos(e2)*cos(e5)*cos(e6)*sin(e3)*sin(e6) + I6yy*de3*cos(e3)*cos(e5)*cos(e6)*sin(e2)*sin(e6) - I6yz*de5*cos(e2)*cos(e3)*cos(e4)*sin(e4)*sin(e6) - 2*I6yz*de4*cos(e2)*cos(e3)*cos(e5)*sin(e5)*sin(e6) + I6yz*de5*cos(e2)*cos(e4)*cos(e6)*sin(e3)*sin(e5) + I6yz*de5*cos(e3)*cos(e4)*cos(e6)*sin(e2)*sin(e5) - 4*I4zx*de1*cos(e2)*cos(e3)*cos(e4)*sin(e2)*sin(e3) - 2*I5zx*de1*cos(e2)*cos(e4)*cos(e5)*sin(e2)*sin(e4) - 2*I5zx*de1*cos(e3)*cos(e4)*cos(e5)*sin(e3)*sin(e4) + 2*I6zx*de1*cos(e2)*cos(e5)*cos(e6)*sin(e2)*sin(e5) + 2*I6zx*de1*cos(e3)*cos(e5)*cos(e6)*sin(e3)*sin(e5) - I6zz*de2*cos(e2)*cos(e3)*cos(e5)*sin(e4)*sin(e5) - I6zz*de3*cos(e2)*cos(e3)*cos(e5)*sin(e4)*sin(e5) + 4*a3*de1*m5*y5*cos(e2)^2*cos(e3)^2*cos(e5) + 4*a3*de1*m6*z6*cos(e2)^2*cos(e3)^2*cos(e5) + 4*d4*de1*m4*x4*cos(e2)^2*cos(e3)^2*cos(e4) - 2*I5xx*de1*cos(e2)*cos(e3)^2*cos(e4)^2*cos(e5)^2*sin(e2) - 2*I5xx*de1*cos(e2)^2*cos(e3)*cos(e4)^2*cos(e5)^2*sin(e3) - 2*I6xx*de1*cos(e2)*cos(e3)^2*cos(e4)^2*cos(e6)^2*sin(e2) - 2*I6xx*de1*cos(e2)*cos(e3)^2*cos(e5)^2*cos(e6)^2*sin(e2) - 2*I6xx*de1*cos(e2)^2*cos(e3)*cos(e4)^2*cos(e6)^2*sin(e3) + I6xx*de1*cos(e2)*cos(e4)^2*cos(e5)^2*cos(e6)^2*sin(e2) - 2*I6xx*de1*cos(e2)^2*cos(e3)*cos(e5)^2*cos(e6)^2*sin(e3) + I6xx*de1*cos(e3)*cos(e4)^2*cos(e5)^2*cos(e6)^2*sin(e3) + 2*I5yy*de1*cos(e2)*cos(e3)^2*cos(e4)^2*cos(e5)^2*sin(e2) + 2*I5yy*de1*cos(e2)^2*cos(e3)*cos(e4)^2*cos(e5)^2*sin(e3) - 2*I6yy*de1*cos(e2)*cos(e3)^2*cos(e4)^2*cos(e5)^2*sin(e2) + 2*I6yy*de1*cos(e2)*cos(e3)^2*cos(e4)^2*cos(e6)^2*sin(e2) - 2*I6yy*de1*cos(e2)^2*cos(e3)*cos(e4)^2*cos(e5)^2*sin(e3) + 2*I6yy*de1*cos(e2)*cos(e3)^2*cos(e5)^2*cos(e6)^2*sin(e2) + 2*I6yy*de1*cos(e2)^2*cos(e3)*cos(e4)^2*cos(e6)^2*sin(e3) - I6yy*de1*cos(e2)*cos(e4)^2*cos(e5)^2*cos(e6)^2*sin(e2) + 2*I6yy*de1*cos(e2)^2*cos(e3)*cos(e5)^2*cos(e6)^2*sin(e3) - I6yy*de1*cos(e3)*cos(e4)^2*cos(e5)^2*cos(e6)^2*sin(e3) - 8*I6yz*de1*cos(e2)^2*cos(e3)^2*cos(e4)*cos(e5)^2*sin(e6) + 2*I6zz*de1*cos(e2)*cos(e3)^2*cos(e4)^2*cos(e5)^2*sin(e2) + 2*I6zz*de1*cos(e2)^2*cos(e3)*cos(e4)^2*cos(e5)^2*sin(e3) - 2*I6xy*de4*cos(e4)*cos(e5)*sin(e2)*sin(e3)*sin(e4) + 2*I5xy*de5*cos(e2)*cos(e5)*sin(e3)*sin(e4)*sin(e5) + 2*I5xy*de5*cos(e3)*cos(e5)*sin(e2)*sin(e4)*sin(e5) - I6xy*de6*cos(e2)*cos(e5)*sin(e3)*sin(e4)*sin(e5) - I6xy*de6*cos(e3)*cos(e5)*sin(e2)*sin(e4)*sin(e5) - 2*I6xy*de6*cos(e5)*cos(e6)*sin(e2)*sin(e3)*sin(e6) + 4*I4yz*de1*cos(e2)*cos(e3)*sin(e2)*sin(e3)*sin(e4) + 2*I5yz*de1*cos(e2)*cos(e4)*sin(e2)*sin(e4)*sin(e5) + 2*I5yz*de1*cos(e3)*cos(e4)*sin(e3)*sin(e4)*sin(e5) - 2*I6yz*de1*cos(e2)*cos(e5)*sin(e2)*sin(e5)*sin(e6) - 2*I6yz*de1*cos(e3)*cos(e5)*sin(e3)*sin(e5)*sin(e6) - 2*I5zx*de4*cos(e4)*cos(e5)*sin(e2)*sin(e3)*sin(e4) + I6zx*de2*cos(e4)*cos(e5)*sin(e2)*sin(e3)*sin(e6) + I6zx*de3*cos(e4)*cos(e5)*sin(e2)*sin(e3)*sin(e6) - I6zx*de5*cos(e4)*cos(e6)*sin(e2)*sin(e3)*sin(e4) - 2*I6zx*de4*cos(e5)*cos(e6)*sin(e2)*sin(e3)*sin(e5) + I6zx*de5*cos(e2)*cos(e4)*sin(e3)*sin(e5)*sin(e6) + I6zx*de5*cos(e3)*cos(e4)*sin(e2)*sin(e5)*sin(e6) + 4*a3*de1*m5*x5*cos(e2)^2*cos(e3)^2*sin(e5) - 8*I6xy*de1*cos(e2)^2*cos(e3)^2*cos(e6)^2*sin(e4)*sin(e5) + I6xx*de4*cos(e4)^2*cos(e5)^2*cos(e6)^2*sin(e2)*sin(e3) - I6yy*de4*cos(e4)^2*cos(e5)^2*cos(e6)^2*sin(e2)*sin(e3) - 4*d4*de1*m4*y4*cos(e2)^2*cos(e3)^2*sin(e4) - I5xx*de2*cos(e5)*sin(e2)*sin(e3)*sin(e4)*sin(e5) - I5xx*de3*cos(e5)*sin(e2)*sin(e3)*sin(e4)*sin(e5) + I5yy*de2*cos(e5)*sin(e2)*sin(e3)*sin(e4)*sin(e5) + I5yy*de3*cos(e5)*sin(e2)*sin(e3)*sin(e4)*sin(e5) - I6yy*de2*cos(e5)*sin(e2)*sin(e3)*sin(e4)*sin(e5) + 2*I5yz*de4*cos(e4)*sin(e2)*sin(e3)*sin(e4)*sin(e5) - I6yy*de3*cos(e5)*sin(e2)*sin(e3)*sin(e4)*sin(e5) + I6yz*de5*cos(e4)*sin(e2)*sin(e3)*sin(e4)*sin(e6) + 2*I6yz*de4*cos(e5)*sin(e2)*sin(e3)*sin(e5)*sin(e6) + I6zz*de2*cos(e5)*sin(e2)*sin(e3)*sin(e4)*sin(e5) + I6zz*de3*cos(e5)*sin(e2)*sin(e3)*sin(e4)*sin(e5) + 4*d4*de1*m5*z5*cos(e2)^2*cos(e3)^2*sin(e4) - 4*de1*m5*x5*y5*cos(e2)^2*cos(e3)^2*cos(e4) - 4*de1*m5*x5*y5*cos(e2)^2*cos(e4)*cos(e5)^2 - 4*de1*m5*x5*y5*cos(e3)^2*cos(e4)*cos(e5)^2 + 4*de1*m4*x4*z4*cos(e2)^2*cos(e3)^2*cos(e4) - de2*m4*x4^2*cos(e2)*cos(e4)*sin(e3)*sin(e4) - de2*m4*x4^2*cos(e3)*cos(e4)*sin(e2)*sin(e4) - de3*m4*x4^2*cos(e2)*cos(e4)*sin(e3)*sin(e4) - de3*m4*x4^2*cos(e3)*cos(e4)*sin(e2)*sin(e4) + de2*m6*x6^2*cos(e2)*cos(e4)*sin(e3)*sin(e4) + de2*m6*x6^2*cos(e3)*cos(e4)*sin(e2)*sin(e4) + de3*m6*x6^2*cos(e2)*cos(e4)*sin(e3)*sin(e4) + de3*m6*x6^2*cos(e3)*cos(e4)*sin(e2)*sin(e4) + de6*m6*x6^2*cos(e2)*cos(e4)*sin(e3)*sin(e5) + de6*m6*x6^2*cos(e3)*cos(e4)*sin(e2)*sin(e5) + de2*m4*y4^2*cos(e2)*cos(e4)*sin(e3)*sin(e4) + de2*m4*y4^2*cos(e3)*cos(e4)*sin(e2)*sin(e4) + de3*m4*y4^2*cos(e2)*cos(e4)*sin(e3)*sin(e4) + de3*m4*y4^2*cos(e3)*cos(e4)*sin(e2)*sin(e4) - de2*m5*y5^2*cos(e2)*cos(e4)*sin(e3)*sin(e4) - de2*m5*y5^2*cos(e3)*cos(e4)*sin(e2)*sin(e4) - de3*m5*y5^2*cos(e2)*cos(e4)*sin(e3)*sin(e4) - de3*m5*y5^2*cos(e3)*cos(e4)*sin(e2)*sin(e4) + de2*m5*z5^2*cos(e2)*cos(e4)*sin(e3)*sin(e4) + de2*m5*z5^2*cos(e3)*cos(e4)*sin(e2)*sin(e4) + de3*m5*z5^2*cos(e2)*cos(e4)*sin(e3)*sin(e4) + de3*m5*z5^2*cos(e3)*cos(e4)*sin(e2)*sin(e4) - de2*m6*z6^2*cos(e2)*cos(e4)*sin(e3)*sin(e4) - de2*m6*z6^2*cos(e3)*cos(e4)*sin(e2)*sin(e4) - de3*m6*z6^2*cos(e2)*cos(e4)*sin(e3)*sin(e4) - de3*m6*z6^2*cos(e3)*cos(e4)*sin(e2)*sin(e4) - 4*de1*m4*y4*z4*cos(e2)^2*cos(e3)^2*sin(e4) - I6yz*de5*cos(e2)*cos(e3)*cos(e4)^2*cos(e5)*cos(e6) - de1*m6*x6^2*cos(e6)*sin(e4)*sin(e5)*sin(e6) + de1*m6*y6^2*cos(e6)*sin(e4)*sin(e5)*sin(e6) + 2*a2*a3*de1*m4*cos(e2)*cos(e3)*sin(e2) + 2*a2*a3*de1*m5*cos(e2)*cos(e3)*sin(e2) + 2*a2*a3*de1*m6*cos(e2)*cos(e3)*sin(e2) + a1*de1*m4*x4*cos(e2)*cos(e3)*cos(e4) + d4*de1*m6*x6*cos(e4)*cos(e5)*cos(e6) - 2*I5xy*de4*cos(e2)*cos(e3)*cos(e4)^2*cos(e5)*sin(e5) - 2*I5xy*de5*cos(e2)*cos(e3)*cos(e4)*cos(e5)^2*sin(e4) - 2*I6xy*de2*cos(e2)*cos(e3)*cos(e4)*cos(e6)^2*sin(e5) - 2*I6xy*de3*cos(e2)*cos(e3)*cos(e4)*cos(e6)^2*sin(e5) + I6xy*de6*cos(e2)*cos(e3)*cos(e4)*cos(e5)^2*sin(e4) - 2*I6xy*de4*cos(e2)*cos(e3)*cos(e4)^2*cos(e6)*sin(e6) - 2*I6xy*de5*cos(e2)*cos(e4)*cos(e5)*cos(e6)^2*sin(e3) - 2*I6xy*de5*cos(e3)*cos(e4)*cos(e5)*cos(e6)^2*sin(e2) - 2*I6xy*de6*cos(e2)*cos(e3)*cos(e4)*cos(e6)^2*sin(e4) + 2*I6xy*de4*cos(e2)*cos(e3)*cos(e5)^2*cos(e6)*sin(e6) - 2*I6zx*de2*cos(e2)*cos(e3)*cos(e5)^2*cos(e6)*sin(e4) - 2*I6zx*de3*cos(e2)*cos(e3)*cos(e5)^2*cos(e6)*sin(e4) - I6zx*de5*cos(e2)*cos(e3)*cos(e4)^2*cos(e5)*sin(e6) - I6zx*de6*cos(e2)*cos(e3)*cos(e4)^2*cos(e6)*sin(e5) - d4*de2*m4*y4*cos(e2)*cos(e3)*cos(e4) - d4*de3*m4*y4*cos(e2)*cos(e3)*cos(e4) + d4*de2*m5*z5*cos(e2)*cos(e3)*cos(e4) + d4*de3*m5*z5*cos(e2)*cos(e3)*cos(e4) - 2*a2*d4*de1*m4*cos(e2)*sin(e2)*sin(e3) - 2*a2*d4*de1*m5*cos(e2)*sin(e2)*sin(e3) - 2*a2*d4*de1*m6*cos(e2)*sin(e2)*sin(e3) + 2*a2*de1*m3*x3*cos(e2)*cos(e3)*sin(e2) - 2*a3*de1*m4*x4*cos(e2)*cos(e4)*sin(e2) - 2*a3*de1*m4*x4*cos(e3)*cos(e4)*sin(e3) - a2*de1*m5*x5*cos(e4)*cos(e5)*sin(e3) - a2*de1*m6*x6*cos(e3)*cos(e6)*sin(e5) - a1*de1*m4*y4*cos(e2)*cos(e3)*sin(e4) - a1*de1*m5*y5*cos(e2)*cos(e5)*sin(e3) - a1*de1*m5*y5*cos(e3)*cos(e5)*sin(e2) - a3*de2*m4*y4*cos(e2)*cos(e4)*sin(e3) - a3*de2*m4*y4*cos(e3)*cos(e4)*sin(e2) - a3*de3*m4*y4*cos(e2)*cos(e4)*sin(e3) - a3*de3*m4*y4*cos(e3)*cos(e4)*sin(e2) - a2*de2*m6*y6*cos(e4)*cos(e6)*sin(e2) + a1*de1*m5*z5*cos(e2)*cos(e3)*sin(e4) - a1*de1*m6*z6*cos(e2)*cos(e5)*sin(e3) - a1*de1*m6*z6*cos(e3)*cos(e5)*sin(e2) + a3*de2*m5*z5*cos(e2)*cos(e4)*sin(e3) + a3*de2*m5*z5*cos(e3)*cos(e4)*sin(e2) + a3*de3*m5*z5*cos(e2)*cos(e4)*sin(e3) + a3*de3*m5*z5*cos(e3)*cos(e4)*sin(e2) - d4*de2*m4*x4*cos(e2)*cos(e3)*sin(e4) - d4*de3*m4*x4*cos(e2)*cos(e3)*sin(e4) - 4*I4xy*de1*cos(e2)*cos(e3)^2*cos(e4)*sin(e2)*sin(e4) - 4*I4xy*de1*cos(e2)^2*cos(e3)*cos(e4)*sin(e3)*sin(e4) - 4*I5xy*de1*cos(e2)*cos(e3)^2*cos(e5)*sin(e2)*sin(e5) + I5xx*de2*cos(e2)*cos(e4)*cos(e5)^2*sin(e3)*sin(e4) + I5xx*de2*cos(e3)*cos(e4)*cos(e5)^2*sin(e2)*sin(e4) + 2*I5xy*de1*cos(e2)*cos(e4)^2*cos(e5)*sin(e2)*sin(e5) - 4*I5xy*de1*cos(e2)^2*cos(e3)*cos(e5)*sin(e3)*sin(e5) + I5xx*de3*cos(e2)*cos(e4)*cos(e5)^2*sin(e3)*sin(e4) + I5xx*de3*cos(e3)*cos(e4)*cos(e5)^2*sin(e2)*sin(e4) + 2*I5xy*de1*cos(e3)*cos(e4)^2*cos(e5)*sin(e3)*sin(e5) + I6xx*de2*cos(e2)*cos(e4)*cos(e6)^2*sin(e3)*sin(e4) + I6xx*de2*cos(e3)*cos(e4)*cos(e6)^2*sin(e2)*sin(e4) + 8*I6xy*de1*cos(e2)*cos(e3)^2*cos(e6)*sin(e2)*sin(e6) + I6xx*de3*cos(e2)*cos(e4)*cos(e6)^2*sin(e3)*sin(e4) + I6xx*de3*cos(e3)*cos(e4)*cos(e6)^2*sin(e2)*sin(e4) + 2*I6xy*de1*cos(e2)*cos(e4)^2*cos(e6)*sin(e2)*sin(e6) + 8*I6xy*de1*cos(e2)^2*cos(e3)*cos(e6)*sin(e3)*sin(e6) + 2*I6xy*de1*cos(e2)*cos(e5)^2*cos(e6)*sin(e2)*sin(e6) + 2*I6xy*de1*cos(e3)*cos(e4)^2*cos(e6)*sin(e3)*sin(e6) + 2*I6xy*de1*cos(e3)*cos(e5)^2*cos(e6)*sin(e3)*sin(e6) + I6xx*de6*cos(e2)*cos(e4)*cos(e6)^2*sin(e3)*sin(e5) + I6xx*de6*cos(e3)*cos(e4)*cos(e6)^2*sin(e2)*sin(e5) - I5yy*de2*cos(e2)*cos(e4)*cos(e5)^2*sin(e3)*sin(e4) - I5yy*de2*cos(e3)*cos(e4)*cos(e5)^2*sin(e2)*sin(e4) - I5yy*de3*cos(e2)*cos(e4)*cos(e5)^2*sin(e3)*sin(e4) - I5yy*de3*cos(e3)*cos(e4)*cos(e5)^2*sin(e2)*sin(e4) + I6yy*de2*cos(e2)*cos(e4)*cos(e5)^2*sin(e3)*sin(e4) + I6yy*de2*cos(e3)*cos(e4)*cos(e5)^2*sin(e2)*sin(e4) - I6yy*de2*cos(e2)*cos(e4)*cos(e6)^2*sin(e3)*sin(e4) - I6yy*de2*cos(e3)*cos(e4)*cos(e6)^2*sin(e2)*sin(e4) + I6yy*de3*cos(e2)*cos(e4)*cos(e5)^2*sin(e3)*sin(e4) + I6yy*de3*cos(e3)*cos(e4)*cos(e5)^2*sin(e2)*sin(e4) - I6yy*de3*cos(e2)*cos(e4)*cos(e6)^2*sin(e3)*sin(e4) - I6yy*de3*cos(e3)*cos(e4)*cos(e6)^2*sin(e2)*sin(e4) + 2*I6yz*de2*cos(e2)*cos(e3)*cos(e5)^2*sin(e4)*sin(e6) + 2*I6yz*de2*cos(e2)*cos(e4)^2*cos(e6)*sin(e3)*sin(e5) + 2*I6yz*de2*cos(e3)*cos(e4)^2*cos(e6)*sin(e2)*sin(e5) + 2*I6yz*de3*cos(e2)*cos(e3)*cos(e5)^2*sin(e4)*sin(e6) + 2*I6yz*de3*cos(e2)*cos(e4)^2*cos(e6)*sin(e3)*sin(e5) + 2*I6yz*de3*cos(e3)*cos(e4)^2*cos(e6)*sin(e2)*sin(e5) - I6yy*de6*cos(e2)*cos(e4)*cos(e6)^2*sin(e3)*sin(e5) - I6yy*de6*cos(e3)*cos(e4)*cos(e6)^2*sin(e2)*sin(e5) + I6yz*de5*cos(e4)^2*cos(e5)*cos(e6)*sin(e2)*sin(e3) + I6yz*de6*cos(e2)*cos(e3)*cos(e4)^2*sin(e5)*sin(e6) + I6yz*de6*cos(e2)*cos(e5)^2*cos(e6)*sin(e3)*sin(e4) + I6yz*de6*cos(e3)*cos(e5)^2*cos(e6)*sin(e2)*sin(e4) - I6zz*de2*cos(e2)*cos(e4)*cos(e5)^2*sin(e3)*sin(e4) - I6zz*de2*cos(e3)*cos(e4)*cos(e5)^2*sin(e2)*sin(e4) - I6zz*de3*cos(e2)*cos(e4)*cos(e5)^2*sin(e3)*sin(e4) - I6zz*de3*cos(e3)*cos(e4)*cos(e5)^2*sin(e2)*sin(e4) + 2*d4*de1*m5*y5*cos(e2)*cos(e5)*sin(e2) + 2*d4*de1*m5*y5*cos(e3)*cos(e5)*sin(e3) - d4*de1*m6*y6*cos(e4)*cos(e5)*sin(e6) + 2*d4*de1*m6*z6*cos(e2)*cos(e5)*sin(e2) + 2*d4*de1*m6*z6*cos(e3)*cos(e5)*sin(e3) - de2*m4*y4*z4*cos(e2)*cos(e3)*cos(e4) - de3*m4*y4*z4*cos(e2)*cos(e3)*cos(e4) - a1*de1*m4*x4*cos(e4)*sin(e2)*sin(e3) - a1*de1*m5*x5*cos(e2)*sin(e3)*sin(e5) - a1*de1*m5*x5*cos(e3)*sin(e2)*sin(e5) - a3*de2*m4*x4*cos(e2)*sin(e3)*sin(e4) - a3*de2*m4*x4*cos(e3)*sin(e2)*sin(e4) - a3*de3*m4*x4*cos(e2)*sin(e3)*sin(e4) - a3*de3*m4*x4*cos(e3)*sin(e2)*sin(e4) - a2*de2*m5*x5*cos(e5)*sin(e2)*sin(e4) - a2*de2*m6*x6*cos(e4)*sin(e2)*sin(e6) - 2*a2*de1*m3*y3*cos(e2)*sin(e2)*sin(e3) + 2*a3*de1*m4*y4*cos(e2)*sin(e2)*sin(e4) + 2*a3*de1*m4*y4*cos(e3)*sin(e3)*sin(e4) + a2*de1*m5*y5*cos(e4)*sin(e3)*sin(e5) + a2*de1*m6*y6*cos(e6)*sin(e3)*sin(e4) + a2*de1*m6*y6*cos(e3)*sin(e5)*sin(e6) - 2*a2*de1*m4*z4*cos(e2)*sin(e2)*sin(e3) - 2*a3*de1*m5*z5*cos(e2)*sin(e2)*sin(e4) - 2*a3*de1*m5*z5*cos(e3)*sin(e3)*sin(e4) + a2*de1*m6*z6*cos(e4)*sin(e3)*sin(e5) + 2*d4*de1*m5*x5*cos(e2)*sin(e2)*sin(e5) + 2*d4*de1*m5*x5*cos(e3)*sin(e3)*sin(e5) + 2*I5xy*de4*cos(e4)^2*cos(e5)*sin(e2)*sin(e3)*sin(e5) + 2*I5xy*de5*cos(e4)*cos(e5)^2*sin(e2)*sin(e3)*sin(e4) + 2*I6xy*de2*cos(e4)*cos(e6)^2*sin(e2)*sin(e3)*sin(e5) - 2*I6xx*de1*cos(e2)^2*cos(e6)*sin(e4)*sin(e5)*sin(e6) + 2*I6xy*de3*cos(e4)*cos(e6)^2*sin(e2)*sin(e3)*sin(e5) - 2*I6xx*de1*cos(e3)^2*cos(e6)*sin(e4)*sin(e5)*sin(e6) - I6xy*de6*cos(e4)*cos(e5)^2*sin(e2)*sin(e3)*sin(e4) + 2*I6xy*de4*cos(e4)^2*cos(e6)*sin(e2)*sin(e3)*sin(e6) + 2*I6xy*de6*cos(e4)*cos(e6)^2*sin(e2)*sin(e3)*sin(e4) - 2*I6xy*de4*cos(e5)^2*cos(e6)*sin(e2)*sin(e3)*sin(e6) + 2*I6yy*de1*cos(e2)^2*cos(e6)*sin(e4)*sin(e5)*sin(e6) + 2*I6yy*de1*cos(e3)^2*cos(e6)*sin(e4)*sin(e5)*sin(e6) + 2*I6zx*de2*cos(e2)*cos(e4)^2*sin(e3)*sin(e5)*sin(e6) + 2*I6zx*de2*cos(e3)*cos(e4)^2*sin(e2)*sin(e5)*sin(e6) + 2*I6zx*de2*cos(e5)^2*cos(e6)*sin(e2)*sin(e3)*sin(e4) + 2*I6zx*de3*cos(e2)*cos(e4)^2*sin(e3)*sin(e5)*sin(e6) + 2*I6zx*de3*cos(e3)*cos(e4)^2*sin(e2)*sin(e5)*sin(e6) + 2*I6zx*de3*cos(e5)^2*cos(e6)*sin(e2)*sin(e3)*sin(e4) + I6zx*de5*cos(e4)^2*cos(e5)*sin(e2)*sin(e3)*sin(e6) + I6zx*de6*cos(e2)*cos(e5)^2*sin(e3)*sin(e4)*sin(e6) + I6zx*de6*cos(e3)*cos(e5)^2*sin(e2)*sin(e4)*sin(e6) + I6zx*de6*cos(e4)^2*cos(e6)*sin(e2)*sin(e3)*sin(e5) + d4*de2*m4*y4*cos(e4)*sin(e2)*sin(e3) + d4*de3*m4*y4*cos(e4)*sin(e2)*sin(e3) - d4*de2*m5*z5*cos(e4)*sin(e2)*sin(e3) - d4*de3*m5*z5*cos(e4)*sin(e2)*sin(e3) - de6*m6*x6^2*cos(e2)*cos(e3)*cos(e4)^2*cos(e5) - de6*m6*x6^2*cos(e2)*cos(e3)*cos(e5)*cos(e6)^2 + de6*m6*y6^2*cos(e2)*cos(e3)*cos(e4)^2*cos(e5) + de6*m6*y6^2*cos(e2)*cos(e3)*cos(e5)*cos(e6)^2 + de2*m5*x5*y5*cos(e2)*cos(e3)*sin(e4) + de3*m5*x5*y5*cos(e2)*cos(e3)*sin(e4) - de2*m6*x6*y6*cos(e2)*cos(e5)*sin(e3) - de2*m6*x6*y6*cos(e3)*cos(e5)*sin(e2) - de3*m6*x6*y6*cos(e2)*cos(e5)*sin(e3) - de3*m6*x6*y6*cos(e3)*cos(e5)*sin(e2) - de2*m4*x4*z4*cos(e2)*cos(e3)*sin(e4) - de3*m4*x4*z4*cos(e2)*cos(e3)*sin(e4) - de2*m5*x5*z5*cos(e2)*cos(e5)*sin(e3) - de2*m5*x5*z5*cos(e3)*cos(e5)*sin(e2) - de3*m5*x5*z5*cos(e2)*cos(e5)*sin(e3) - de3*m5*x5*z5*cos(e3)*cos(e5)*sin(e2) - de1*m6*y6*z6*cos(e5)*cos(e6)*sin(e4) + a2*de1*m6*x6*sin(e3)*sin(e4)*sin(e6) + a1*de1*m4*y4*sin(e2)*sin(e3)*sin(e4) + a2*de2*m5*y5*sin(e2)*sin(e4)*sin(e5) - a1*de1*m5*z5*sin(e2)*sin(e3)*sin(e4) + a2*de2*m6*z6*sin(e2)*sin(e4)*sin(e5) + d4*de2*m4*x4*sin(e2)*sin(e3)*sin(e4) + d4*de3*m4*x4*sin(e2)*sin(e3)*sin(e4) - 2*I6yz*de2*cos(e5)^2*sin(e2)*sin(e3)*sin(e4)*sin(e6) - 2*I6yz*de3*cos(e5)^2*sin(e2)*sin(e3)*sin(e4)*sin(e6) - I6yz*de6*cos(e4)^2*sin(e2)*sin(e3)*sin(e5)*sin(e6) - 2*de1*m5*x5^2*cos(e2)^2*cos(e4)*cos(e5)*sin(e5) - 2*de1*m5*x5^2*cos(e3)^2*cos(e4)*cos(e5)*sin(e5) + de1*m6*x6^2*cos(e4)*cos(e5)*cos(e6)^2*sin(e5) + 2*de1*m5*y5^2*cos(e2)^2*cos(e4)*cos(e5)*sin(e5) + 2*de1*m5*y5^2*cos(e3)^2*cos(e4)*cos(e5)*sin(e5) - 2*de1*m6*y6^2*cos(e2)^2*cos(e4)*cos(e5)*sin(e5) - 2*de1*m6*y6^2*cos(e3)^2*cos(e4)*cos(e5)*sin(e5) - de1*m6*y6^2*cos(e4)*cos(e5)*cos(e6)^2*sin(e5) + 2*de1*m6*z6^2*cos(e2)^2*cos(e4)*cos(e5)*sin(e5) + 2*de1*m6*z6^2*cos(e3)^2*cos(e4)*cos(e5)*sin(e5) - de1*m6*x6*z6*cos(e5)*sin(e4)*sin(e6) + de2*m4*y4*z4*cos(e4)*sin(e2)*sin(e3) + de3*m4*y4*z4*cos(e4)*sin(e2)*sin(e3) + de2*m5*y5*z5*cos(e2)*sin(e3)*sin(e5) + de2*m5*y5*z5*cos(e3)*sin(e2)*sin(e5) + de3*m5*y5*z5*cos(e2)*sin(e3)*sin(e5) + de3*m5*y5*z5*cos(e3)*sin(e2)*sin(e5) - de5*m5*x5^2*cos(e2)*cos(e5)^2*sin(e3)*sin(e4) - de5*m5*x5^2*cos(e3)*cos(e5)^2*sin(e2)*sin(e4) + de6*m6*x6^2*cos(e4)^2*cos(e5)*sin(e2)*sin(e3) + de6*m6*x6^2*cos(e5)*cos(e6)^2*sin(e2)*sin(e3) + de5*m5*y5^2*cos(e2)*cos(e5)^2*sin(e3)*sin(e4) + de5*m5*y5^2*cos(e3)*cos(e5)^2*sin(e2)*sin(e4) - de5*m6*y6^2*cos(e2)*cos(e5)^2*sin(e3)*sin(e4) - de5*m6*y6^2*cos(e3)*cos(e5)^2*sin(e2)*sin(e4) - de6*m6*y6^2*cos(e4)^2*cos(e5)*sin(e2)*sin(e3) - de6*m6*y6^2*cos(e5)*cos(e6)^2*sin(e2)*sin(e3) - de2*m5*x5*y5*sin(e2)*sin(e3)*sin(e4) - de3*m5*x5*y5*sin(e2)*sin(e3)*sin(e4) + de5*m6*z6^2*cos(e2)*cos(e5)^2*sin(e3)*sin(e4) + de5*m6*z6^2*cos(e3)*cos(e5)^2*sin(e2)*sin(e4) + de2*m4*x4*z4*sin(e2)*sin(e3)*sin(e4) + de3*m4*x4*z4*sin(e2)*sin(e3)*sin(e4) - 2*I6xx*de6*cos(e2)*cos(e3)*cos(e4)^2*cos(e5)*cos(e6)^2 + 2*I6yy*de6*cos(e2)*cos(e3)*cos(e4)^2*cos(e5)*cos(e6)^2 + 2*a2*de1*m5*y5*cos(e2)^2*cos(e3)*cos(e5) + 2*a2*de1*m6*z6*cos(e2)^2*cos(e3)*cos(e5) - 2*d4*de1*m5*x5*cos(e2)^2*cos(e4)*cos(e5) - 2*d4*de1*m5*x5*cos(e3)^2*cos(e4)*cos(e5) - 4*I5xx*de1*cos(e2)^2*cos(e3)^2*cos(e4)*cos(e5)*sin(e5) + 2*I6xx*de1*cos(e2)^2*cos(e4)*cos(e5)*cos(e6)^2*sin(e5) - 4*I6xy*de2*cos(e2)*cos(e4)^2*cos(e5)*cos(e6)^2*sin(e3) - 4*I6xy*de2*cos(e3)*cos(e4)^2*cos(e5)*cos(e6)^2*sin(e2) + 2*I6xx*de1*cos(e3)^2*cos(e4)*cos(e5)*cos(e6)^2*sin(e5) - 4*I6xy*de3*cos(e2)*cos(e4)^2*cos(e5)*cos(e6)^2*sin(e3) - 4*I6xy*de3*cos(e3)*cos(e4)^2*cos(e5)*cos(e6)^2*sin(e2) - 2*I6xy*de5*cos(e2)*cos(e3)*cos(e4)^2*cos(e6)^2*sin(e5) + 4*I5yy*de1*cos(e2)^2*cos(e3)^2*cos(e4)*cos(e5)*sin(e5) - 4*I6yy*de1*cos(e2)^2*cos(e3)^2*cos(e4)*cos(e5)*sin(e5) - 4*I6yz*de1*cos(e2)^2*cos(e3)^2*cos(e5)*cos(e6)*sin(e4) - 2*I6yy*de1*cos(e2)^2*cos(e4)*cos(e5)*cos(e6)^2*sin(e5) - 2*I6yy*de1*cos(e3)^2*cos(e4)*cos(e5)*cos(e6)^2*sin(e5) + 4*I6zz*de1*cos(e2)^2*cos(e3)^2*cos(e4)*cos(e5)*sin(e5) + 2*a2*de1*m4*x4*cos(e2)^2*cos(e4)*sin(e3) + 2*a2*de1*m5*x5*cos(e2)^2*cos(e3)*sin(e5) - 2*a3*de1*m6*x6*cos(e2)^2*cos(e6)*sin(e5) - 2*a3*de1*m6*x6*cos(e3)^2*cos(e6)*sin(e5) + I6xx*de5*cos(e2)*cos(e5)^2*cos(e6)^2*sin(e3)*sin(e4) + I6xx*de5*cos(e3)*cos(e5)^2*cos(e6)^2*sin(e2)*sin(e4) + 2*I6xx*de6*cos(e4)^2*cos(e5)*cos(e6)^2*sin(e2)*sin(e3) - I6yy*de5*cos(e2)*cos(e5)^2*cos(e6)^2*sin(e3)*sin(e4) - I6yy*de5*cos(e3)*cos(e5)^2*cos(e6)^2*sin(e2)*sin(e4) - 2*I6yy*de6*cos(e4)^2*cos(e5)*cos(e6)^2*sin(e2)*sin(e3) - 4*I6zx*de1*cos(e2)^2*cos(e3)^2*cos(e5)*sin(e4)*sin(e6) + 2*d4*de1*m5*y5*cos(e2)^2*cos(e4)*sin(e5) + 2*d4*de1*m5*y5*cos(e3)^2*cos(e4)*sin(e5) + 2*d4*de1*m6*y6*cos(e2)^2*cos(e6)*sin(e4) + 2*d4*de1*m6*y6*cos(e3)^2*cos(e6)*sin(e4) - 4*d4*de1*m4*z4*cos(e2)*cos(e3)^2*sin(e2) - 4*d4*de1*m4*z4*cos(e2)^2*cos(e3)*sin(e3) + 2*d4*de1*m6*z6*cos(e2)^2*cos(e4)*sin(e5) + 2*d4*de1*m6*z6*cos(e3)^2*cos(e4)*sin(e5) + 2*de1*m6*x6*z6*cos(e2)^2*cos(e4)*cos(e6) + 2*de1*m6*x6*z6*cos(e3)^2*cos(e4)*cos(e6) + 2*de1*m6*x6*z6*cos(e4)*cos(e5)^2*cos(e6) - 2*a2*de1*m4*y4*cos(e2)^2*sin(e3)*sin(e4) + 2*a3*de1*m6*y6*cos(e2)^2*sin(e5)*sin(e6) + 2*a3*de1*m6*y6*cos(e3)^2*sin(e5)*sin(e6) + 2*a2*de1*m5*z5*cos(e2)^2*sin(e3)*sin(e4) + 2*d4*de1*m6*x6*cos(e2)^2*sin(e4)*sin(e6) + 2*d4*de1*m6*x6*cos(e3)^2*sin(e4)*sin(e6) + 2*I6xy*de5*cos(e4)^2*cos(e6)^2*sin(e2)*sin(e3)*sin(e5) + de4*m5*x5^2*cos(e2)*cos(e3)*cos(e4)^2*cos(e5)^2 + de4*m6*x6^2*cos(e2)*cos(e3)*cos(e4)^2*cos(e6)^2 - de4*m6*x6^2*cos(e2)*cos(e3)*cos(e5)^2*cos(e6)^2 - de4*m5*y5^2*cos(e2)*cos(e3)*cos(e4)^2*cos(e5)^2 + de4*m6*y6^2*cos(e2)*cos(e3)*cos(e4)^2*cos(e5)^2 - de4*m6*y6^2*cos(e2)*cos(e3)*cos(e4)^2*cos(e6)^2 + de4*m6*y6^2*cos(e2)*cos(e3)*cos(e5)^2*cos(e6)^2 - 2*de2*m4*x4*y4*cos(e2)*cos(e4)^2*sin(e3) - 2*de2*m4*x4*y4*cos(e3)*cos(e4)^2*sin(e2) - 2*de3*m4*x4*y4*cos(e2)*cos(e4)^2*sin(e3) - 2*de3*m4*x4*y4*cos(e3)*cos(e4)^2*sin(e2) - de4*m6*z6^2*cos(e2)*cos(e3)*cos(e4)^2*cos(e5)^2 - 2*de1*m5*y5*z5*cos(e2)^2*cos(e5)*sin(e4) - 2*de1*m5*y5*z5*cos(e3)^2*cos(e5)*sin(e4) - 2*de1*m6*y6*z6*cos(e2)^2*cos(e4)*sin(e6) - 2*de1*m6*y6*z6*cos(e3)^2*cos(e4)*sin(e6) - 2*de1*m6*y6*z6*cos(e4)*cos(e5)^2*sin(e6) - I6yz*de2*cos(e2)*cos(e3)*cos(e4)*cos(e5)*cos(e6) - I6yz*de3*cos(e2)*cos(e3)*cos(e4)*cos(e5)*cos(e6) + 2*de1*m4*x4^2*cos(e2)*cos(e3)^2*cos(e4)^2*sin(e2) + 2*de1*m4*x4^2*cos(e2)^2*cos(e3)*cos(e4)^2*sin(e3) + 2*de1*m5*x5^2*cos(e2)*cos(e3)^2*cos(e5)^2*sin(e2) - de1*m5*x5^2*cos(e2)*cos(e4)^2*cos(e5)^2*sin(e2) + 2*de1*m5*x5^2*cos(e2)^2*cos(e3)*cos(e5)^2*sin(e3) - 2*de1*m6*x6^2*cos(e2)*cos(e3)^2*cos(e4)^2*sin(e2) - 2*de1*m6*x6^2*cos(e2)^2*cos(e3)*cos(e4)^2*sin(e3) - de1*m5*x5^2*cos(e3)*cos(e4)^2*cos(e5)^2*sin(e3) - 4*de1*m6*x6^2*cos(e2)*cos(e3)^2*cos(e6)^2*sin(e2) - de1*m6*x6^2*cos(e2)*cos(e4)^2*cos(e6)^2*sin(e2) - 4*de1*m6*x6^2*cos(e2)^2*cos(e3)*cos(e6)^2*sin(e3) - de1*m6*x6^2*cos(e2)*cos(e5)^2*cos(e6)^2*sin(e2) - de1*m6*x6^2*cos(e3)*cos(e4)^2*cos(e6)^2*sin(e3) - de1*m6*x6^2*cos(e3)*cos(e5)^2*cos(e6)^2*sin(e3) - 2*de1*m4*y4^2*cos(e2)*cos(e3)^2*cos(e4)^2*sin(e2) - 2*de1*m4*y4^2*cos(e2)^2*cos(e3)*cos(e4)^2*sin(e3) + 2*de1*m5*y5^2*cos(e2)*cos(e3)^2*cos(e4)^2*sin(e2) - 2*de1*m5*y5^2*cos(e2)*cos(e3)^2*cos(e5)^2*sin(e2) + 2*de1*m5*y5^2*cos(e2)^2*cos(e3)*cos(e4)^2*sin(e3) + de1*m5*y5^2*cos(e2)*cos(e4)^2*cos(e5)^2*sin(e2) - 2*de1*m5*y5^2*cos(e2)^2*cos(e3)*cos(e5)^2*sin(e3) + 2*de1*m6*y6^2*cos(e2)*cos(e3)^2*cos(e5)^2*sin(e2) + de1*m5*y5^2*cos(e3)*cos(e4)^2*cos(e5)^2*sin(e3) + 4*de1*m6*y6^2*cos(e2)*cos(e3)^2*cos(e6)^2*sin(e2) - de1*m6*y6^2*cos(e2)*cos(e4)^2*cos(e5)^2*sin(e2) + 2*de1*m6*y6^2*cos(e2)^2*cos(e3)*cos(e5)^2*sin(e3) + de1*m6*y6^2*cos(e2)*cos(e4)^2*cos(e6)^2*sin(e2) + 4*de1*m6*y6^2*cos(e2)^2*cos(e3)*cos(e6)^2*sin(e3) + de1*m6*y6^2*cos(e2)*cos(e5)^2*cos(e6)^2*sin(e2) - de1*m6*y6^2*cos(e3)*cos(e4)^2*cos(e5)^2*sin(e3) + de1*m6*y6^2*cos(e3)*cos(e4)^2*cos(e6)^2*sin(e3) + de1*m6*y6^2*cos(e3)*cos(e5)^2*cos(e6)^2*sin(e3) - 2*de1*m6*x6*y6*cos(e2)^2*sin(e4)*sin(e5) - 2*de1*m6*x6*y6*cos(e3)^2*sin(e4)*sin(e5) - 2*de1*m6*x6*y6*cos(e6)^2*sin(e4)*sin(e5) - 2*de1*m5*z5^2*cos(e2)*cos(e3)^2*cos(e4)^2*sin(e2) - 2*de1*m5*z5^2*cos(e2)^2*cos(e3)*cos(e4)^2*sin(e3) + 2*de1*m6*z6^2*cos(e2)*cos(e3)^2*cos(e4)^2*sin(e2) - 2*de1*m6*z6^2*cos(e2)*cos(e3)^2*cos(e5)^2*sin(e2) + 2*de1*m6*z6^2*cos(e2)^2*cos(e3)*cos(e4)^2*sin(e3) + de1*m6*z6^2*cos(e2)*cos(e4)^2*cos(e5)^2*sin(e2) - 2*de1*m6*z6^2*cos(e2)^2*cos(e3)*cos(e5)^2*sin(e3) + de1*m6*z6^2*cos(e3)*cos(e4)^2*cos(e5)^2*sin(e3) - 2*de1*m5*x5*z5*cos(e2)^2*sin(e4)*sin(e5) - 2*de1*m5*x5*z5*cos(e3)^2*sin(e4)*sin(e5) - 4*de1*m6*x6*z6*cos(e2)^2*cos(e3)^2*cos(e4)*cos(e6) - 4*de1*m6*x6*z6*cos(e2)^2*cos(e4)*cos(e5)^2*cos(e6) - 4*de1*m6*x6*z6*cos(e3)^2*cos(e4)*cos(e5)^2*cos(e6) - 4*a3*de1*m6*y6*cos(e2)^2*cos(e3)^2*sin(e5)*sin(e6) - 4*d4*de1*m6*x6*cos(e2)^2*cos(e3)^2*sin(e4)*sin(e6) - 2*I6zx*de4*cos(e4)*sin(e2)*sin(e3)*sin(e4)*sin(e5)*sin(e6) + de4*m6*x6^2*cos(e2)*cos(e3)*cos(e4)^2*cos(e5)^2*cos(e6)^2 - de4*m6*y6^2*cos(e2)*cos(e3)*cos(e4)^2*cos(e5)^2*cos(e6)^2 - de2*m5*x5^2*cos(e2)*cos(e3)*cos(e5)*sin(e4)*sin(e5) - de3*m5*x5^2*cos(e2)*cos(e3)*cos(e5)*sin(e4)*sin(e5) + de2*m6*x6^2*cos(e2)*cos(e5)*cos(e6)*sin(e3)*sin(e6) + de2*m6*x6^2*cos(e3)*cos(e5)*cos(e6)*sin(e2)*sin(e6) + de3*m6*x6^2*cos(e2)*cos(e5)*cos(e6)*sin(e3)*sin(e6) + de3*m6*x6^2*cos(e3)*cos(e5)*cos(e6)*sin(e2)*sin(e6) + de2*m5*y5^2*cos(e2)*cos(e3)*cos(e5)*sin(e4)*sin(e5) + de3*m5*y5^2*cos(e2)*cos(e3)*cos(e5)*sin(e4)*sin(e5) - de2*m6*y6^2*cos(e2)*cos(e3)*cos(e5)*sin(e4)*sin(e5) - de3*m6*y6^2*cos(e2)*cos(e3)*cos(e5)*sin(e4)*sin(e5) - de2*m6*y6^2*cos(e2)*cos(e5)*cos(e6)*sin(e3)*sin(e6) - de2*m6*y6^2*cos(e3)*cos(e5)*cos(e6)*sin(e2)*sin(e6) - de3*m6*y6^2*cos(e2)*cos(e5)*cos(e6)*sin(e3)*sin(e6) - de3*m6*y6^2*cos(e3)*cos(e5)*cos(e6)*sin(e2)*sin(e6) + de2*m6*z6^2*cos(e2)*cos(e3)*cos(e5)*sin(e4)*sin(e5) + de3*m6*z6^2*cos(e2)*cos(e3)*cos(e5)*sin(e4)*sin(e5) + 4*de1*m5*y5*z5*cos(e2)^2*cos(e3)^2*cos(e5)*sin(e4) + 4*de1*m6*y6*z6*cos(e2)^2*cos(e3)^2*cos(e4)*sin(e6) + 4*de1*m6*y6*z6*cos(e2)^2*cos(e4)*cos(e5)^2*sin(e6) + 4*de1*m6*y6*z6*cos(e3)^2*cos(e4)*cos(e5)^2*sin(e6) + 2*de1*m5*x5^2*cos(e2)*cos(e3)^2*cos(e4)^2*cos(e5)^2*sin(e2) + 2*de1*m5*x5^2*cos(e2)^2*cos(e3)*cos(e4)^2*cos(e5)^2*sin(e3) + 2*de1*m6*x6^2*cos(e2)*cos(e3)^2*cos(e4)^2*cos(e6)^2*sin(e2) + 2*de1*m6*x6^2*cos(e2)*cos(e3)^2*cos(e5)^2*cos(e6)^2*sin(e2) + 2*de1*m6*x6^2*cos(e2)^2*cos(e3)*cos(e4)^2*cos(e6)^2*sin(e3) - de1*m6*x6^2*cos(e2)*cos(e4)^2*cos(e5)^2*cos(e6)^2*sin(e2) + 2*de1*m6*x6^2*cos(e2)^2*cos(e3)*cos(e5)^2*cos(e6)^2*sin(e3) - de1*m6*x6^2*cos(e3)*cos(e4)^2*cos(e5)^2*cos(e6)^2*sin(e3) - 2*de1*m5*y5^2*cos(e2)*cos(e3)^2*cos(e4)^2*cos(e5)^2*sin(e2) - 2*de1*m5*y5^2*cos(e2)^2*cos(e3)*cos(e4)^2*cos(e5)^2*sin(e3) + 2*de1*m6*y6^2*cos(e2)*cos(e3)^2*cos(e4)^2*cos(e5)^2*sin(e2) - 2*de1*m6*y6^2*cos(e2)*cos(e3)^2*cos(e4)^2*cos(e6)^2*sin(e2) + 2*de1*m6*y6^2*cos(e2)^2*cos(e3)*cos(e4)^2*cos(e5)^2*sin(e3) - 2*de1*m6*y6^2*cos(e2)*cos(e3)^2*cos(e5)^2*cos(e6)^2*sin(e2) - 2*de1*m6*y6^2*cos(e2)^2*cos(e3)*cos(e4)^2*cos(e6)^2*sin(e3) + de1*m6*y6^2*cos(e2)*cos(e4)^2*cos(e5)^2*cos(e6)^2*sin(e2) - 2*de1*m6*y6^2*cos(e2)^2*cos(e3)*cos(e5)^2*cos(e6)^2*sin(e3) + de1*m6*y6^2*cos(e3)*cos(e4)^2*cos(e5)^2*cos(e6)^2*sin(e3) + 4*de1*m6*x6*y6*cos(e2)^2*cos(e3)^2*sin(e4)*sin(e5) + 4*de1*m6*x6*y6*cos(e2)^2*cos(e6)^2*sin(e4)*sin(e5) + 4*de1*m6*x6*y6*cos(e3)^2*cos(e6)^2*sin(e4)*sin(e5) - 2*de1*m6*z6^2*cos(e2)*cos(e3)^2*cos(e4)^2*cos(e5)^2*sin(e2) - 2*de1*m6*z6^2*cos(e2)^2*cos(e3)*cos(e4)^2*cos(e5)^2*sin(e3) + 4*de1*m5*x5*z5*cos(e2)^2*cos(e3)^2*sin(e4)*sin(e5) + a1*de1*m5*x5*cos(e2)*cos(e3)*cos(e4)*cos(e5) - 4*I6xy*de4*cos(e2)*cos(e3)*cos(e4)*cos(e5)*cos(e6)^2*sin(e4) - 4*I6xy*de6*cos(e2)*cos(e3)*cos(e4)^2*cos(e5)*cos(e6)*sin(e6) - 2*I6zx*de4*cos(e2)*cos(e3)*cos(e4)^2*cos(e5)*cos(e6)*sin(e5) - 2*I6zx*de5*cos(e2)*cos(e3)*cos(e4)*cos(e5)^2*cos(e6)*sin(e4) - d4*de2*m6*y6*cos(e2)*cos(e3)*cos(e4)*cos(e6) - d4*de3*m6*y6*cos(e2)*cos(e3)*cos(e4)*cos(e6) - de4*m6*x6^2*cos(e4)^2*cos(e5)^2*cos(e6)^2*sin(e2)*sin(e3) + de4*m6*y6^2*cos(e4)^2*cos(e5)^2*cos(e6)^2*sin(e2)*sin(e3) + de2*m5*x5^2*cos(e5)*sin(e2)*sin(e3)*sin(e4)*sin(e5) + de3*m5*x5^2*cos(e5)*sin(e2)*sin(e3)*sin(e4)*sin(e5) - de2*m5*y5^2*cos(e5)*sin(e2)*sin(e3)*sin(e4)*sin(e5) - de3*m5*y5^2*cos(e5)*sin(e2)*sin(e3)*sin(e4)*sin(e5) + de2*m6*y6^2*cos(e5)*sin(e2)*sin(e3)*sin(e4)*sin(e5) + de3*m6*y6^2*cos(e5)*sin(e2)*sin(e3)*sin(e4)*sin(e5) - de2*m6*z6^2*cos(e5)*sin(e2)*sin(e3)*sin(e4)*sin(e5) - de3*m6*z6^2*cos(e5)*sin(e2)*sin(e3)*sin(e4)*sin(e5) - 4*a3*d4*de1*m4*cos(e2)*cos(e3)*sin(e2)*sin(e3) - 4*a3*d4*de1*m5*cos(e2)*cos(e3)*sin(e2)*sin(e3) - 4*a3*d4*de1*m6*cos(e2)*cos(e3)*sin(e2)*sin(e3) + 2*a2*de1*m4*x4*cos(e2)*cos(e3)*cos(e4)*sin(e2) - 2*a3*de1*m5*x5*cos(e2)*cos(e4)*cos(e5)*sin(e2) - 2*a3*de1*m5*x5*cos(e3)*cos(e4)*cos(e5)*sin(e3) - a2*de1*m6*x6*cos(e4)*cos(e5)*cos(e6)*sin(e3) - a1*de1*m5*y5*cos(e2)*cos(e3)*cos(e4)*sin(e5) - a1*de1*m6*y6*cos(e2)*cos(e3)*cos(e6)*sin(e4) - a3*de2*m6*y6*cos(e2)*cos(e4)*cos(e6)*sin(e3) - a3*de2*m6*y6*cos(e3)*cos(e4)*cos(e6)*sin(e2) - a3*de3*m6*y6*cos(e2)*cos(e4)*cos(e6)*sin(e3) - a3*de3*m6*y6*cos(e3)*cos(e4)*cos(e6)*sin(e2) - a1*de1*m6*z6*cos(e2)*cos(e3)*cos(e4)*sin(e5) - d4*de2*m5*x5*cos(e2)*cos(e3)*cos(e5)*sin(e4) - d4*de3*m5*x5*cos(e2)*cos(e3)*cos(e5)*sin(e4) - d4*de2*m6*x6*cos(e2)*cos(e3)*cos(e4)*sin(e6) - d4*de3*m6*x6*cos(e2)*cos(e3)*cos(e4)*sin(e6) - 8*I5xy*de1*cos(e2)*cos(e3)*cos(e4)*cos(e5)^2*sin(e2)*sin(e3) + 4*I6xy*de1*cos(e2)*cos(e3)^2*cos(e4)*cos(e5)*sin(e2)*sin(e4) + 4*I6xy*de1*cos(e2)^2*cos(e3)*cos(e4)*cos(e5)*sin(e3)*sin(e4) + 4*I6xy*de1*cos(e2)*cos(e4)*cos(e5)*cos(e6)^2*sin(e2)*sin(e4) + I6xx*de2*cos(e2)*cos(e3)*cos(e5)*cos(e6)^2*sin(e4)*sin(e5) + 4*I6xy*de1*cos(e3)*cos(e4)*cos(e5)*cos(e6)^2*sin(e3)*sin(e4) + 2*I6xx*de2*cos(e2)*cos(e4)^2*cos(e5)*cos(e6)*sin(e3)*sin(e6) + 2*I6xx*de2*cos(e3)*cos(e4)^2*cos(e5)*cos(e6)*sin(e2)*sin(e6) + I6xx*de3*cos(e2)*cos(e3)*cos(e5)*cos(e6)^2*sin(e4)*sin(e5) + 2*I6xx*de3*cos(e2)*cos(e4)^2*cos(e5)*cos(e6)*sin(e3)*sin(e6) + 2*I6xx*de3*cos(e3)*cos(e4)^2*cos(e5)*cos(e6)*sin(e2)*sin(e6) + 4*I6xy*de1*cos(e2)^2*cos(e4)*cos(e5)*cos(e6)*sin(e5)*sin(e6) + I6xx*de5*cos(e2)*cos(e3)*cos(e4)^2*cos(e6)*sin(e5)*sin(e6) + 4*I6xy*de1*cos(e3)^2*cos(e4)*cos(e5)*cos(e6)*sin(e5)*sin(e6) - I6yy*de2*cos(e2)*cos(e3)*cos(e5)*cos(e6)^2*sin(e4)*sin(e5) - 2*I6yy*de2*cos(e2)*cos(e4)^2*cos(e5)*cos(e6)*sin(e3)*sin(e6) - 2*I6yy*de2*cos(e3)*cos(e4)^2*cos(e5)*cos(e6)*sin(e2)*sin(e6) - I6yy*de3*cos(e2)*cos(e3)*cos(e5)*cos(e6)^2*sin(e4)*sin(e5) - 2*I6yy*de3*cos(e2)*cos(e4)^2*cos(e5)*cos(e6)*sin(e3)*sin(e6) - 2*I6yy*de3*cos(e3)*cos(e4)^2*cos(e5)*cos(e6)*sin(e2)*sin(e6) + 2*I6yz*de4*cos(e2)*cos(e3)*cos(e4)^2*cos(e5)*sin(e5)*sin(e6) + 2*I6yz*de5*cos(e2)*cos(e3)*cos(e4)*cos(e5)^2*sin(e4)*sin(e6) - I6yy*de5*cos(e2)*cos(e3)*cos(e4)^2*cos(e6)*sin(e5)*sin(e6) + 4*I5zx*de1*cos(e2)*cos(e3)^2*cos(e4)*cos(e5)*sin(e2)*sin(e4) + 4*I5zx*de1*cos(e2)^2*cos(e3)*cos(e4)*cos(e5)*sin(e3)*sin(e4) - 4*I6zx*de1*cos(e2)*cos(e3)^2*cos(e5)*cos(e6)*sin(e2)*sin(e5) + 2*I6zx*de1*cos(e2)*cos(e4)^2*cos(e5)*cos(e6)*sin(e2)*sin(e5) - 4*I6zx*de1*cos(e2)^2*cos(e3)*cos(e5)*cos(e6)*sin(e3)*sin(e5) + 2*I6zx*de1*cos(e3)*cos(e4)^2*cos(e5)*cos(e6)*sin(e3)*sin(e5) + de2*m5*y5*z5*cos(e2)*cos(e3)*cos(e4)*cos(e5) + de3*m5*y5*z5*cos(e2)*cos(e3)*cos(e4)*cos(e5) - a1*de1*m5*x5*cos(e4)*cos(e5)*sin(e2)*sin(e3) - a1*de1*m6*x6*cos(e2)*cos(e3)*sin(e4)*sin(e6) - a3*de2*m5*x5*cos(e2)*cos(e5)*sin(e3)*sin(e4) - a3*de2*m5*x5*cos(e3)*cos(e5)*sin(e2)*sin(e4) - a1*de1*m6*x6*cos(e2)*cos(e6)*sin(e3)*sin(e5) - a1*de1*m6*x6*cos(e3)*cos(e6)*sin(e2)*sin(e5) - a3*de3*m5*x5*cos(e2)*cos(e5)*sin(e3)*sin(e4) - a3*de3*m5*x5*cos(e3)*cos(e5)*sin(e2)*sin(e4) - a3*de2*m6*x6*cos(e2)*cos(e4)*sin(e3)*sin(e6) - a3*de2*m6*x6*cos(e3)*cos(e4)*sin(e2)*sin(e6) - a2*de2*m6*x6*cos(e5)*cos(e6)*sin(e2)*sin(e4) - a3*de3*m6*x6*cos(e2)*cos(e4)*sin(e3)*sin(e6) - a3*de3*m6*x6*cos(e3)*cos(e4)*sin(e2)*sin(e6) - 2*a2*de1*m4*y4*cos(e2)*cos(e3)*sin(e2)*sin(e4) - 2*a2*de1*m5*y5*cos(e2)*cos(e5)*sin(e2)*sin(e3) + 2*a3*de1*m5*y5*cos(e2)*cos(e4)*sin(e2)*sin(e5) + 2*a3*de1*m5*y5*cos(e3)*cos(e4)*sin(e3)*sin(e5) + 2*a3*de1*m6*y6*cos(e2)*cos(e6)*sin(e2)*sin(e4) + 2*a3*de1*m6*y6*cos(e3)*cos(e6)*sin(e3)*sin(e4) + a2*de1*m6*y6*cos(e4)*cos(e5)*sin(e3)*sin(e6) - 2*I6xx*de1*cos(e2)*cos(e3)^2*cos(e4)^2*cos(e5)^2*cos(e6)^2*sin(e2) - 2*I6xx*de1*cos(e2)^2*cos(e3)*cos(e4)^2*cos(e5)^2*cos(e6)^2*sin(e3) + 2*I6yy*de1*cos(e2)*cos(e3)^2*cos(e4)^2*cos(e5)^2*cos(e6)^2*sin(e2) + 2*I6yy*de1*cos(e2)^2*cos(e3)*cos(e4)^2*cos(e5)^2*cos(e6)^2*sin(e3) - 4*a3*de1*m4*z4*cos(e2)*cos(e3)*sin(e2)*sin(e3) + 2*a2*de1*m5*z5*cos(e2)*cos(e3)*sin(e2)*sin(e4) - 2*a2*de1*m6*z6*cos(e2)*cos(e5)*sin(e2)*sin(e3) + 2*a3*de1*m6*z6*cos(e2)*cos(e4)*sin(e2)*sin(e5) + 2*a3*de1*m6*z6*cos(e3)*cos(e4)*sin(e3)*sin(e5) + 2*d4*de1*m6*x6*cos(e2)*cos(e6)*sin(e2)*sin(e5) + 2*d4*de1*m6*x6*cos(e3)*cos(e6)*sin(e3)*sin(e5) + 4*I6xy*de4*cos(e4)*cos(e5)*cos(e6)^2*sin(e2)*sin(e3)*sin(e4) + 2*I6xy*de5*cos(e2)*cos(e5)^2*cos(e6)*sin(e3)*sin(e4)*sin(e6) + 2*I6xy*de5*cos(e3)*cos(e5)^2*cos(e6)*sin(e2)*sin(e4)*sin(e6) + 2*I6xy*de6*cos(e2)*cos(e5)*cos(e6)^2*sin(e3)*sin(e4)*sin(e5) + 2*I6xy*de6*cos(e3)*cos(e5)*cos(e6)^2*sin(e2)*sin(e4)*sin(e5) + 4*I6xy*de6*cos(e4)^2*cos(e5)*cos(e6)*sin(e2)*sin(e3)*sin(e6) - 4*I5yz*de1*cos(e2)*cos(e3)^2*cos(e4)*sin(e2)*sin(e4)*sin(e5) - 4*I5yz*de1*cos(e2)^2*cos(e3)*cos(e4)*sin(e3)*sin(e4)*sin(e5) + 4*I6yz*de1*cos(e2)*cos(e3)^2*cos(e5)*sin(e2)*sin(e5)*sin(e6) - 2*I6yz*de1*cos(e2)*cos(e4)^2*cos(e5)*sin(e2)*sin(e5)*sin(e6) + 4*I6yz*de1*cos(e2)^2*cos(e3)*cos(e5)*sin(e3)*sin(e5)*sin(e6) - 2*I6yz*de1*cos(e3)*cos(e4)^2*cos(e5)*sin(e3)*sin(e5)*sin(e6) + 2*I6zx*de4*cos(e4)^2*cos(e5)*cos(e6)*sin(e2)*sin(e3)*sin(e5) + 2*I6zx*de5*cos(e4)*cos(e5)^2*cos(e6)*sin(e2)*sin(e3)*sin(e4) + d4*de2*m5*y5*cos(e2)*cos(e3)*sin(e4)*sin(e5) + d4*de3*m5*y5*cos(e2)*cos(e3)*sin(e4)*sin(e5) + d4*de2*m6*y6*cos(e4)*cos(e6)*sin(e2)*sin(e3) + d4*de3*m6*y6*cos(e4)*cos(e6)*sin(e2)*sin(e3) + d4*de2*m6*z6*cos(e2)*cos(e3)*sin(e4)*sin(e5) + d4*de3*m6*z6*cos(e2)*cos(e3)*sin(e4)*sin(e5) - 2*de4*m4*x4*y4*cos(e2)*cos(e3)*cos(e4)*sin(e4) + de5*m5*x5*y5*cos(e2)*cos(e3)*cos(e4)*sin(e4) + de2*m6*x6*y6*cos(e2)*cos(e3)*cos(e4)*sin(e5) + 2*de4*m5*x5*y5*cos(e2)*cos(e3)*cos(e5)*sin(e5) + de3*m6*x6*y6*cos(e2)*cos(e3)*cos(e4)*sin(e5) + de5*m6*x6*y6*cos(e2)*cos(e4)*cos(e5)*sin(e3) + de5*m6*x6*y6*cos(e3)*cos(e4)*cos(e5)*sin(e2) + de6*m6*x6*y6*cos(e2)*cos(e3)*cos(e4)*sin(e4) + de2*m5*x5*z5*cos(e2)*cos(e3)*cos(e4)*sin(e5) + de3*m5*x5*z5*cos(e2)*cos(e3)*cos(e4)*sin(e5) + de5*m5*x5*z5*cos(e2)*cos(e4)*cos(e5)*sin(e3) + de5*m5*x5*z5*cos(e3)*cos(e4)*cos(e5)*sin(e2) + de2*m6*x6*z6*cos(e2)*cos(e3)*cos(e6)*sin(e4) + de3*m6*x6*z6*cos(e2)*cos(e3)*cos(e6)*sin(e4) + de6*m6*x6*z6*cos(e2)*cos(e3)*cos(e6)*sin(e5) - 2*a2*de1*m5*x5*cos(e2)*sin(e2)*sin(e3)*sin(e5) + 2*a3*de1*m6*x6*cos(e2)*sin(e2)*sin(e4)*sin(e6) + 2*a3*de1*m6*x6*cos(e3)*sin(e3)*sin(e4)*sin(e6) + a1*de1*m5*y5*cos(e4)*sin(e2)*sin(e3)*sin(e5) + a1*de1*m6*y6*cos(e6)*sin(e2)*sin(e3)*sin(e4) + a3*de2*m5*y5*cos(e2)*sin(e3)*sin(e4)*sin(e5) + a3*de2*m5*y5*cos(e3)*sin(e2)*sin(e4)*sin(e5) + a1*de1*m6*y6*cos(e2)*sin(e3)*sin(e5)*sin(e6) + a1*de1*m6*y6*cos(e3)*sin(e2)*sin(e5)*sin(e6) + a3*de3*m5*y5*cos(e2)*sin(e3)*sin(e4)*sin(e5) + a3*de3*m5*y5*cos(e3)*sin(e2)*sin(e4)*sin(e5) + a2*de2*m6*y6*cos(e5)*sin(e2)*sin(e4)*sin(e6) + a1*de1*m6*z6*cos(e4)*sin(e2)*sin(e3)*sin(e5) + a3*de2*m6*z6*cos(e2)*sin(e3)*sin(e4)*sin(e5) + a3*de2*m6*z6*cos(e3)*sin(e2)*sin(e4)*sin(e5) + a3*de3*m6*z6*cos(e2)*sin(e3)*sin(e4)*sin(e5) + a3*de3*m6*z6*cos(e3)*sin(e2)*sin(e4)*sin(e5) + d4*de2*m5*x5*cos(e5)*sin(e2)*sin(e3)*sin(e4) + d4*de3*m5*x5*cos(e5)*sin(e2)*sin(e3)*sin(e4) + d4*de2*m6*x6*cos(e4)*sin(e2)*sin(e3)*sin(e6) + d4*de3*m6*x6*cos(e4)*sin(e2)*sin(e3)*sin(e6) - I6xx*de2*cos(e5)*cos(e6)^2*sin(e2)*sin(e3)*sin(e4)*sin(e5) - I6xx*de3*cos(e5)*cos(e6)^2*sin(e2)*sin(e3)*sin(e4)*sin(e5) - I6xx*de5*cos(e4)^2*cos(e6)*sin(e2)*sin(e3)*sin(e5)*sin(e6) + I6yy*de2*cos(e5)*cos(e6)^2*sin(e2)*sin(e3)*sin(e4)*sin(e5) + I6yy*de3*cos(e5)*cos(e6)^2*sin(e2)*sin(e3)*sin(e4)*sin(e5) - 2*I6yz*de4*cos(e4)^2*cos(e5)*sin(e2)*sin(e3)*sin(e5)*sin(e6) - 2*I6yz*de5*cos(e4)*cos(e5)^2*sin(e2)*sin(e3)*sin(e4)*sin(e6) + I6yy*de5*cos(e4)^2*cos(e6)*sin(e2)*sin(e3)*sin(e5)*sin(e6) - 2*d4*de1*m6*y6*cos(e2)*sin(e2)*sin(e5)*sin(e6) - 2*d4*de1*m6*y6*cos(e3)*sin(e3)*sin(e5)*sin(e6) + 8*de1*m5*x5*y5*cos(e2)^2*cos(e3)^2*cos(e4)*cos(e5)^2 - 4*de1*m3*x3*y3*cos(e2)*cos(e3)*sin(e2)*sin(e3) + 2*de1*m4*x4*y4*cos(e2)*cos(e4)*sin(e2)*sin(e4) + 2*de1*m4*x4*y4*cos(e3)*cos(e4)*sin(e3)*sin(e4) + 2*de1*m5*x5*y5*cos(e2)*cos(e5)*sin(e2)*sin(e5) + 2*de1*m5*x5*y5*cos(e3)*cos(e5)*sin(e3)*sin(e5) - 4*de1*m6*x6*y6*cos(e2)*cos(e6)*sin(e2)*sin(e6) - 4*de1*m6*x6*y6*cos(e3)*cos(e6)*sin(e3)*sin(e6) - de2*m5*y5*z5*cos(e4)*cos(e5)*sin(e2)*sin(e3) - de3*m5*y5*z5*cos(e4)*cos(e5)*sin(e2)*sin(e3) - de5*m5*y5*z5*cos(e2)*cos(e4)*sin(e3)*sin(e5) - de5*m5*y5*z5*cos(e3)*cos(e4)*sin(e2)*sin(e5) - de2*m6*y6*z6*cos(e2)*cos(e3)*sin(e4)*sin(e6) - de2*m6*y6*z6*cos(e2)*cos(e6)*sin(e3)*sin(e5) - de2*m6*y6*z6*cos(e3)*cos(e6)*sin(e2)*sin(e5) - de3*m6*y6*z6*cos(e2)*cos(e3)*sin(e4)*sin(e6) - de3*m6*y6*z6*cos(e2)*cos(e6)*sin(e3)*sin(e5) - de3*m6*y6*z6*cos(e3)*cos(e6)*sin(e2)*sin(e5) - de6*m6*y6*z6*cos(e2)*cos(e6)*sin(e3)*sin(e4) - de6*m6*y6*z6*cos(e3)*cos(e6)*sin(e2)*sin(e4) - de6*m6*y6*z6*cos(e2)*cos(e3)*sin(e5)*sin(e6) + a1*de1*m6*x6*sin(e2)*sin(e3)*sin(e4)*sin(e6) - d4*de2*m5*y5*sin(e2)*sin(e3)*sin(e4)*sin(e5) - d4*de3*m5*y5*sin(e2)*sin(e3)*sin(e4)*sin(e5) - d4*de2*m6*z6*sin(e2)*sin(e3)*sin(e4)*sin(e5) - d4*de3*m6*z6*sin(e2)*sin(e3)*sin(e4)*sin(e5) - de2*m5*x5^2*cos(e2)*cos(e4)*cos(e5)^2*sin(e3)*sin(e4) - de2*m5*x5^2*cos(e3)*cos(e4)*cos(e5)^2*sin(e2)*sin(e4) - de3*m5*x5^2*cos(e2)*cos(e4)*cos(e5)^2*sin(e3)*sin(e4) - de3*m5*x5^2*cos(e3)*cos(e4)*cos(e5)^2*sin(e2)*sin(e4) - de2*m6*x6^2*cos(e2)*cos(e4)*cos(e6)^2*sin(e3)*sin(e4) - de2*m6*x6^2*cos(e3)*cos(e4)*cos(e6)^2*sin(e2)*sin(e4) - de3*m6*x6^2*cos(e2)*cos(e4)*cos(e6)^2*sin(e3)*sin(e4) - de3*m6*x6^2*cos(e3)*cos(e4)*cos(e6)^2*sin(e2)*sin(e4) - de6*m6*x6^2*cos(e2)*cos(e4)*cos(e6)^2*sin(e3)*sin(e5) - de6*m6*x6^2*cos(e3)*cos(e4)*cos(e6)^2*sin(e2)*sin(e5) + de2*m5*y5^2*cos(e2)*cos(e4)*cos(e5)^2*sin(e3)*sin(e4) + de2*m5*y5^2*cos(e3)*cos(e4)*cos(e5)^2*sin(e2)*sin(e4) + de3*m5*y5^2*cos(e2)*cos(e4)*cos(e5)^2*sin(e3)*sin(e4) + de3*m5*y5^2*cos(e3)*cos(e4)*cos(e5)^2*sin(e2)*sin(e4) - de2*m6*y6^2*cos(e2)*cos(e4)*cos(e5)^2*sin(e3)*sin(e4) - de2*m6*y6^2*cos(e3)*cos(e4)*cos(e5)^2*sin(e2)*sin(e4) + de2*m6*y6^2*cos(e2)*cos(e4)*cos(e6)^2*sin(e3)*sin(e4) + de2*m6*y6^2*cos(e3)*cos(e4)*cos(e6)^2*sin(e2)*sin(e4) - de3*m6*y6^2*cos(e2)*cos(e4)*cos(e5)^2*sin(e3)*sin(e4) - de3*m6*y6^2*cos(e3)*cos(e4)*cos(e5)^2*sin(e2)*sin(e4) + de3*m6*y6^2*cos(e2)*cos(e4)*cos(e6)^2*sin(e3)*sin(e4) + de3*m6*y6^2*cos(e3)*cos(e4)*cos(e6)^2*sin(e2)*sin(e4) + de6*m6*y6^2*cos(e2)*cos(e4)*cos(e6)^2*sin(e3)*sin(e5) + de6*m6*y6^2*cos(e3)*cos(e4)*cos(e6)^2*sin(e2)*sin(e5) + 2*de4*m4*x4*y4*cos(e4)*sin(e2)*sin(e3)*sin(e4) - de5*m5*x5*y5*cos(e4)*sin(e2)*sin(e3)*sin(e4) - de2*m6*x6*y6*cos(e4)*sin(e2)*sin(e3)*sin(e5) - 2*de4*m5*x5*y5*cos(e5)*sin(e2)*sin(e3)*sin(e5) - de3*m6*x6*y6*cos(e4)*sin(e2)*sin(e3)*sin(e5) - de6*m6*x6*y6*cos(e4)*sin(e2)*sin(e3)*sin(e4) + de2*m6*z6^2*cos(e2)*cos(e4)*cos(e5)^2*sin(e3)*sin(e4) + de2*m6*z6^2*cos(e3)*cos(e4)*cos(e5)^2*sin(e2)*sin(e4) + de3*m6*z6^2*cos(e2)*cos(e4)*cos(e5)^2*sin(e3)*sin(e4) + de3*m6*z6^2*cos(e3)*cos(e4)*cos(e5)^2*sin(e2)*sin(e4) - de2*m5*x5*z5*cos(e4)*sin(e2)*sin(e3)*sin(e5) - de3*m5*x5*z5*cos(e4)*sin(e2)*sin(e3)*sin(e5) - de2*m6*x6*z6*cos(e6)*sin(e2)*sin(e3)*sin(e4) - de2*m6*x6*z6*cos(e2)*sin(e3)*sin(e5)*sin(e6) - de2*m6*x6*z6*cos(e3)*sin(e2)*sin(e5)*sin(e6) - de3*m6*x6*z6*cos(e6)*sin(e2)*sin(e3)*sin(e4) - de3*m6*x6*z6*cos(e2)*sin(e3)*sin(e5)*sin(e6) - de3*m6*x6*z6*cos(e3)*sin(e2)*sin(e5)*sin(e6) - de6*m6*x6*z6*cos(e2)*sin(e3)*sin(e4)*sin(e6) - de6*m6*x6*z6*cos(e3)*sin(e2)*sin(e4)*sin(e6) - de6*m6*x6*z6*cos(e6)*sin(e2)*sin(e3)*sin(e5) + 2*de1*m6*x6^2*cos(e2)^2*cos(e6)*sin(e4)*sin(e5)*sin(e6) + 2*de1*m6*x6^2*cos(e3)^2*cos(e6)*sin(e4)*sin(e5)*sin(e6) - 2*de1*m6*y6^2*cos(e2)^2*cos(e6)*sin(e4)*sin(e5)*sin(e6) - 2*de1*m6*y6^2*cos(e3)^2*cos(e6)*sin(e4)*sin(e5)*sin(e6) + de2*m6*y6*z6*sin(e2)*sin(e3)*sin(e4)*sin(e6) + de3*m6*y6*z6*sin(e2)*sin(e3)*sin(e4)*sin(e6) + de6*m6*y6*z6*sin(e2)*sin(e3)*sin(e5)*sin(e6) - 2*d4*de1*m6*x6*cos(e2)^2*cos(e4)*cos(e5)*cos(e6) - 2*d4*de1*m6*x6*cos(e3)^2*cos(e4)*cos(e5)*cos(e6) - 2*I6xy*de4*cos(e2)*cos(e3)*cos(e4)^2*cos(e5)^2*cos(e6)*sin(e6) - 2*I6xy*de6*cos(e2)*cos(e3)*cos(e4)*cos(e5)^2*cos(e6)^2*sin(e4) + 4*a3*de1*m4*x4*cos(e2)*cos(e3)^2*cos(e4)*sin(e2) + 4*a3*de1*m4*x4*cos(e2)^2*cos(e3)*cos(e4)*sin(e3) + 2*a2*de1*m5*x5*cos(e2)^2*cos(e4)*cos(e5)*sin(e3) + 2*a2*de1*m6*x6*cos(e2)^2*cos(e3)*cos(e6)*sin(e5) - 4*I5xy*de1*cos(e2)*cos(e3)^2*cos(e4)^2*cos(e5)*sin(e2)*sin(e5) - 4*I5xy*de1*cos(e2)^2*cos(e3)*cos(e4)^2*cos(e5)*sin(e3)*sin(e5) - 4*I6xy*de1*cos(e2)*cos(e3)^2*cos(e4)^2*cos(e6)*sin(e2)*sin(e6) + I6xx*de2*cos(e2)*cos(e4)*cos(e5)^2*cos(e6)^2*sin(e3)*sin(e4) + I6xx*de2*cos(e3)*cos(e4)*cos(e5)^2*cos(e6)^2*sin(e2)*sin(e4) - 4*I6xy*de1*cos(e2)*cos(e3)^2*cos(e5)^2*cos(e6)*sin(e2)*sin(e6) - 4*I6xy*de1*cos(e2)^2*cos(e3)*cos(e4)^2*cos(e6)*sin(e3)*sin(e6) + I6xx*de3*cos(e2)*cos(e4)*cos(e5)^2*cos(e6)^2*sin(e3)*sin(e4) + I6xx*de3*cos(e3)*cos(e4)*cos(e5)^2*cos(e6)^2*sin(e2)*sin(e4) + 2*I6xy*de1*cos(e2)*cos(e4)^2*cos(e5)^2*cos(e6)*sin(e2)*sin(e6) - 4*I6xy*de1*cos(e2)^2*cos(e3)*cos(e5)^2*cos(e6)*sin(e3)*sin(e6) + 2*I6xy*de1*cos(e3)*cos(e4)^2*cos(e5)^2*cos(e6)*sin(e3)*sin(e6) - I6yy*de2*cos(e2)*cos(e4)*cos(e5)^2*cos(e6)^2*sin(e3)*sin(e4) - I6yy*de2*cos(e3)*cos(e4)*cos(e5)^2*cos(e6)^2*sin(e2)*sin(e4) - I6yy*de3*cos(e2)*cos(e4)*cos(e5)^2*cos(e6)^2*sin(e3)*sin(e4) - I6yy*de3*cos(e3)*cos(e4)*cos(e5)^2*cos(e6)^2*sin(e2)*sin(e4) - 4*d4*de1*m5*y5*cos(e2)*cos(e3)^2*cos(e5)*sin(e2) - 4*d4*de1*m5*y5*cos(e2)^2*cos(e3)*cos(e5)*sin(e3) + 2*d4*de1*m6*y6*cos(e2)^2*cos(e4)*cos(e5)*sin(e6) + 2*d4*de1*m6*y6*cos(e3)^2*cos(e4)*cos(e5)*sin(e6) - 4*d4*de1*m6*z6*cos(e2)*cos(e3)^2*cos(e5)*sin(e2) - 4*d4*de1*m6*z6*cos(e2)^2*cos(e3)*cos(e5)*sin(e3) + de5*m5*y5*z5*cos(e2)*cos(e3)*cos(e4)^2*cos(e5) - 4*a3*de1*m4*y4*cos(e2)*cos(e3)^2*sin(e2)*sin(e4) - 4*a3*de1*m4*y4*cos(e2)^2*cos(e3)*sin(e3)*sin(e4) - 2*a2*de1*m5*y5*cos(e2)^2*cos(e4)*sin(e3)*sin(e5) - 2*a2*de1*m6*y6*cos(e2)^2*cos(e6)*sin(e3)*sin(e4) - 2*a2*de1*m6*y6*cos(e2)^2*cos(e3)*sin(e5)*sin(e6) + 4*a3*de1*m5*z5*cos(e2)*cos(e3)^2*sin(e2)*sin(e4) + 4*a3*de1*m5*z5*cos(e2)^2*cos(e3)*sin(e3)*sin(e4) - 2*a2*de1*m6*z6*cos(e2)^2*cos(e4)*sin(e3)*sin(e5) - 4*d4*de1*m5*x5*cos(e2)*cos(e3)^2*sin(e2)*sin(e5) - 4*d4*de1*m5*x5*cos(e2)^2*cos(e3)*sin(e3)*sin(e5) + 4*I6xx*de1*cos(e2)^2*cos(e3)^2*cos(e6)*sin(e4)*sin(e5)*sin(e6) + 2*I6xy*de4*cos(e4)^2*cos(e5)^2*cos(e6)*sin(e2)*sin(e3)*sin(e6) + 2*I6xy*de6*cos(e4)*cos(e5)^2*cos(e6)^2*sin(e2)*sin(e3)*sin(e4) - 4*I6yy*de1*cos(e2)^2*cos(e3)^2*cos(e6)*sin(e4)*sin(e5)*sin(e6) + 2*de6*m6*x6^2*cos(e2)*cos(e3)*cos(e4)^2*cos(e5)*cos(e6)^2 - 2*de6*m6*y6^2*cos(e2)*cos(e3)*cos(e4)^2*cos(e5)*cos(e6)^2 - 2*de2*m5*x5*y5*cos(e2)*cos(e3)*cos(e5)^2*sin(e4) - 2*de3*m5*x5*y5*cos(e2)*cos(e3)*cos(e5)^2*sin(e4) + 2*de2*m6*x6*y6*cos(e2)*cos(e4)^2*cos(e5)*sin(e3) + 2*de2*m6*x6*y6*cos(e3)*cos(e4)^2*cos(e5)*sin(e2) + 2*de3*m6*x6*y6*cos(e2)*cos(e4)^2*cos(e5)*sin(e3) + 2*de3*m6*x6*y6*cos(e3)*cos(e4)^2*cos(e5)*sin(e2) + 2*de2*m6*x6*y6*cos(e2)*cos(e5)*cos(e6)^2*sin(e3) + 2*de2*m6*x6*y6*cos(e3)*cos(e5)*cos(e6)^2*sin(e2) + 2*de3*m6*x6*y6*cos(e2)*cos(e5)*cos(e6)^2*sin(e3) + 2*de3*m6*x6*y6*cos(e3)*cos(e5)*cos(e6)^2*sin(e2) + de5*m6*x6*y6*cos(e2)*cos(e3)*cos(e4)^2*sin(e5) + 2*de2*m5*x5*z5*cos(e2)*cos(e4)^2*cos(e5)*sin(e3) + 2*de2*m5*x5*z5*cos(e3)*cos(e4)^2*cos(e5)*sin(e2) + 2*de3*m5*x5*z5*cos(e2)*cos(e4)^2*cos(e5)*sin(e3) + 2*de3*m5*x5*z5*cos(e3)*cos(e4)^2*cos(e5)*sin(e2) + de5*m5*x5*z5*cos(e2)*cos(e3)*cos(e4)^2*sin(e5) + 2*de1*m6*y6*z6*cos(e2)^2*cos(e5)*cos(e6)*sin(e4) + 2*de1*m6*y6*z6*cos(e3)^2*cos(e5)*cos(e6)*sin(e4) - 2*a2*de1*m6*x6*cos(e2)^2*sin(e3)*sin(e4)*sin(e6) + 4*de1*m5*x5^2*cos(e2)^2*cos(e3)^2*cos(e4)*cos(e5)*sin(e5) - 2*de1*m6*x6^2*cos(e2)^2*cos(e4)*cos(e5)*cos(e6)^2*sin(e5) - 2*de1*m6*x6^2*cos(e3)^2*cos(e4)*cos(e5)*cos(e6)^2*sin(e5) - 4*de1*m5*y5^2*cos(e2)^2*cos(e3)^2*cos(e4)*cos(e5)*sin(e5) + 4*de1*m6*y6^2*cos(e2)^2*cos(e3)^2*cos(e4)*cos(e5)*sin(e5) + 2*de1*m6*y6^2*cos(e2)^2*cos(e4)*cos(e5)*cos(e6)^2*sin(e5) + 2*de1*m6*y6^2*cos(e3)^2*cos(e4)*cos(e5)*cos(e6)^2*sin(e5) - 4*de1*m6*z6^2*cos(e2)^2*cos(e3)^2*cos(e4)*cos(e5)*sin(e5) + 2*de1*m6*x6*z6*cos(e2)^2*cos(e5)*sin(e4)*sin(e6) + 2*de1*m6*x6*z6*cos(e3)^2*cos(e5)*sin(e4)*sin(e6) - 2*de2*m5*y5*z5*cos(e2)*cos(e4)^2*sin(e3)*sin(e5) - 2*de2*m5*y5*z5*cos(e3)*cos(e4)^2*sin(e2)*sin(e5) - 2*de3*m5*y5*z5*cos(e2)*cos(e4)^2*sin(e3)*sin(e5) - 2*de3*m5*y5*z5*cos(e3)*cos(e4)^2*sin(e2)*sin(e5) - de5*m5*y5*z5*cos(e4)^2*cos(e5)*sin(e2)*sin(e3) - de5*m6*x6^2*cos(e2)*cos(e5)^2*cos(e6)^2*sin(e3)*sin(e4) - de5*m6*x6^2*cos(e3)*cos(e5)^2*cos(e6)^2*sin(e2)*sin(e4) - 2*de6*m6*x6^2*cos(e4)^2*cos(e5)*cos(e6)^2*sin(e2)*sin(e3) + de5*m6*y6^2*cos(e2)*cos(e5)^2*cos(e6)^2*sin(e3)*sin(e4) + de5*m6*y6^2*cos(e3)*cos(e5)^2*cos(e6)^2*sin(e2)*sin(e4) + 2*de6*m6*y6^2*cos(e4)^2*cos(e5)*cos(e6)^2*sin(e2)*sin(e3) + 2*de2*m5*x5*y5*cos(e5)^2*sin(e2)*sin(e3)*sin(e4) + 2*de3*m5*x5*y5*cos(e5)^2*sin(e2)*sin(e3)*sin(e4) - de5*m6*x6*y6*cos(e4)^2*sin(e2)*sin(e3)*sin(e5) - de5*m5*x5*z5*cos(e4)^2*sin(e2)*sin(e3)*sin(e5) + I5xx*de5*cos(e2)*cos(e3)*cos(e4)*cos(e5)*sin(e4)*sin(e5) + I6xx*de2*cos(e2)*cos(e3)*cos(e4)*cos(e6)*sin(e5)*sin(e6) + I6xx*de3*cos(e2)*cos(e3)*cos(e4)*cos(e6)*sin(e5)*sin(e6) + I6xx*de5*cos(e2)*cos(e4)*cos(e5)*cos(e6)*sin(e3)*sin(e6) + I6xx*de5*cos(e3)*cos(e4)*cos(e5)*cos(e6)*sin(e2)*sin(e6) + I6xx*de6*cos(e2)*cos(e3)*cos(e4)*cos(e6)*sin(e4)*sin(e6) - I5yy*de5*cos(e2)*cos(e3)*cos(e4)*cos(e5)*sin(e4)*sin(e5) - I6yy*de2*cos(e2)*cos(e3)*cos(e4)*cos(e6)*sin(e5)*sin(e6) + I6yy*de5*cos(e2)*cos(e3)*cos(e4)*cos(e5)*sin(e4)*sin(e5) - I6yy*de3*cos(e2)*cos(e3)*cos(e4)*cos(e6)*sin(e5)*sin(e6) + 2*I6yz*de4*cos(e2)*cos(e3)*cos(e4)*cos(e6)*sin(e4)*sin(e5) - I6yy*de5*cos(e2)*cos(e4)*cos(e5)*cos(e6)*sin(e3)*sin(e6) - I6yy*de5*cos(e3)*cos(e4)*cos(e5)*cos(e6)*sin(e2)*sin(e6) - I6yy*de6*cos(e2)*cos(e3)*cos(e4)*cos(e6)*sin(e4)*sin(e6) + 4*I6zx*de1*cos(e2)*cos(e3)*cos(e4)*cos(e6)*sin(e2)*sin(e3) - I6zz*de5*cos(e2)*cos(e3)*cos(e4)*cos(e5)*sin(e4)*sin(e5) + 4*d4*de1*m5*x5*cos(e2)^2*cos(e3)^2*cos(e4)*cos(e5) - 4*I6xx*de1*cos(e2)^2*cos(e3)^2*cos(e4)*cos(e5)*cos(e6)^2*sin(e5) + 4*I6yy*de1*cos(e2)^2*cos(e3)^2*cos(e4)*cos(e5)*cos(e6)^2*sin(e5) + 2*I5xy*de2*cos(e2)*cos(e4)*cos(e5)*sin(e3)*sin(e4)*sin(e5) + 2*I5xy*de2*cos(e3)*cos(e4)*cos(e5)*sin(e2)*sin(e4)*sin(e5) + 2*I5xy*de3*cos(e2)*cos(e4)*cos(e5)*sin(e3)*sin(e4)*sin(e5) + 2*I5xy*de3*cos(e3)*cos(e4)*cos(e5)*sin(e2)*sin(e4)*sin(e5) + 2*I6xy*de2*cos(e2)*cos(e4)*cos(e6)*sin(e3)*sin(e4)*sin(e6) + 2*I6xy*de2*cos(e3)*cos(e4)*cos(e6)*sin(e2)*sin(e4)*sin(e6) + 2*I6xy*de3*cos(e2)*cos(e4)*cos(e6)*sin(e3)*sin(e4)*sin(e6) + 2*I6xy*de3*cos(e3)*cos(e4)*cos(e6)*sin(e2)*sin(e4)*sin(e6) + 2*I6xy*de6*cos(e2)*cos(e4)*cos(e6)*sin(e3)*sin(e5)*sin(e6) + 2*I6xy*de6*cos(e3)*cos(e4)*cos(e6)*sin(e2)*sin(e5)*sin(e6) - 4*I5yz*de1*cos(e2)*cos(e3)*cos(e5)*sin(e2)*sin(e3)*sin(e4) - 4*I6yz*de1*cos(e2)*cos(e3)*cos(e4)*sin(e2)*sin(e3)*sin(e6) - 2*I6yz*de1*cos(e2)*cos(e4)*cos(e6)*sin(e2)*sin(e4)*sin(e5) - 2*I6yz*de1*cos(e3)*cos(e4)*cos(e6)*sin(e3)*sin(e4)*sin(e5) + 2*I6zx*de4*cos(e2)*cos(e3)*cos(e4)*sin(e4)*sin(e5)*sin(e6) + 2*I6zx*de5*cos(e2)*cos(e5)*cos(e6)*sin(e3)*sin(e4)*sin(e5) + 2*I6zx*de5*cos(e3)*cos(e5)*cos(e6)*sin(e2)*sin(e4)*sin(e5) + 4*a3*de1*m6*x6*cos(e2)^2*cos(e3)^2*cos(e6)*sin(e5) - 4*d4*de1*m5*y5*cos(e2)^2*cos(e3)^2*cos(e4)*sin(e5) - 4*d4*de1*m6*y6*cos(e2)^2*cos(e3)^2*cos(e6)*sin(e4) - 4*I6xy*de1*cos(e2)*cos(e3)*sin(e2)*sin(e3)*sin(e4)*sin(e5) - I5xx*de5*cos(e4)*cos(e5)*sin(e2)*sin(e3)*sin(e4)*sin(e5) - I6xx*de2*cos(e4)*cos(e6)*sin(e2)*sin(e3)*sin(e5)*sin(e6) - I6xx*de3*cos(e4)*cos(e6)*sin(e2)*sin(e3)*sin(e5)*sin(e6) - I6xx*de6*cos(e4)*cos(e6)*sin(e2)*sin(e3)*sin(e4)*sin(e6) + I5yy*de5*cos(e4)*cos(e5)*sin(e2)*sin(e3)*sin(e4)*sin(e5) + I6yy*de2*cos(e4)*cos(e6)*sin(e2)*sin(e3)*sin(e5)*sin(e6) - I6yy*de5*cos(e4)*cos(e5)*sin(e2)*sin(e3)*sin(e4)*sin(e5) + I6yy*de3*cos(e4)*cos(e6)*sin(e2)*sin(e3)*sin(e5)*sin(e6) - 2*I6yz*de4*cos(e4)*cos(e6)*sin(e2)*sin(e3)*sin(e4)*sin(e5) + I6yy*de6*cos(e4)*cos(e6)*sin(e2)*sin(e3)*sin(e4)*sin(e6) - 2*I6yz*de5*cos(e2)*cos(e5)*sin(e3)*sin(e4)*sin(e5)*sin(e6) - 2*I6yz*de5*cos(e3)*cos(e5)*sin(e2)*sin(e4)*sin(e5)*sin(e6) - 4*I5zx*de1*cos(e2)*cos(e3)*sin(e2)*sin(e3)*sin(e4)*sin(e5) - 2*I6zx*de1*cos(e2)*cos(e4)*sin(e2)*sin(e4)*sin(e5)*sin(e6) - 2*I6zx*de1*cos(e3)*cos(e4)*sin(e3)*sin(e4)*sin(e5)*sin(e6) + I6zz*de5*cos(e4)*cos(e5)*sin(e2)*sin(e3)*sin(e4)*sin(e5) - 4*d4*de1*m6*z6*cos(e2)^2*cos(e3)^2*cos(e4)*sin(e5) + 2*a2*de1*m5*x5*cos(e2)*cos(e3)*cos(e4)*cos(e5)*sin(e2) - 2*a3*de1*m6*x6*cos(e2)*cos(e4)*cos(e5)*cos(e6)*sin(e2) - 2*a3*de1*m6*x6*cos(e3)*cos(e4)*cos(e5)*cos(e6)*sin(e3) - a1*de1*m6*y6*cos(e2)*cos(e3)*cos(e4)*cos(e5)*sin(e6) - d4*de2*m6*x6*cos(e2)*cos(e3)*cos(e5)*cos(e6)*sin(e4) - d4*de3*m6*x6*cos(e2)*cos(e3)*cos(e5)*cos(e6)*sin(e4) + I6xx*de5*cos(e2)*cos(e3)*cos(e4)*cos(e5)*cos(e6)^2*sin(e4)*sin(e5) + I6xx*de6*cos(e2)*cos(e3)*cos(e4)*cos(e5)^2*cos(e6)*sin(e4)*sin(e6) - I6yy*de5*cos(e2)*cos(e3)*cos(e4)*cos(e5)*cos(e6)^2*sin(e4)*sin(e5) - I6yy*de6*cos(e2)*cos(e3)*cos(e4)*cos(e5)^2*cos(e6)*sin(e4)*sin(e6) - 8*I6zx*de1*cos(e2)*cos(e3)*cos(e4)*cos(e5)^2*cos(e6)*sin(e2)*sin(e3) - de2*m6*y6*z6*cos(e2)*cos(e3)*cos(e4)*cos(e5)*cos(e6) - de3*m6*y6*z6*cos(e2)*cos(e3)*cos(e4)*cos(e5)*cos(e6) - a1*de1*m6*x6*cos(e4)*cos(e5)*cos(e6)*sin(e2)*sin(e3) - a3*de2*m6*x6*cos(e2)*cos(e5)*cos(e6)*sin(e3)*sin(e4) - a3*de2*m6*x6*cos(e3)*cos(e5)*cos(e6)*sin(e2)*sin(e4) - a3*de3*m6*x6*cos(e2)*cos(e5)*cos(e6)*sin(e3)*sin(e4) - a3*de3*m6*x6*cos(e3)*cos(e5)*cos(e6)*sin(e2)*sin(e4) - 2*a2*de1*m5*y5*cos(e2)*cos(e3)*cos(e4)*sin(e2)*sin(e5) - 4*a3*de1*m5*y5*cos(e2)*cos(e3)*cos(e5)*sin(e2)*sin(e3) - 2*a2*de1*m6*y6*cos(e2)*cos(e3)*cos(e6)*sin(e2)*sin(e4) + 2*a3*de1*m6*y6*cos(e2)*cos(e4)*cos(e5)*sin(e2)*sin(e6) + 2*a3*de1*m6*y6*cos(e3)*cos(e4)*cos(e5)*sin(e3)*sin(e6) - 2*a2*de1*m6*z6*cos(e2)*cos(e3)*cos(e4)*sin(e2)*sin(e5) - 4*a3*de1*m6*z6*cos(e2)*cos(e3)*cos(e5)*sin(e2)*sin(e3) - 4*d4*de1*m4*x4*cos(e2)*cos(e3)*cos(e4)*sin(e2)*sin(e3) + 2*I6xy*de2*cos(e2)*cos(e4)*cos(e5)^2*cos(e6)*sin(e3)*sin(e4)*sin(e6) + 2*I6xy*de2*cos(e3)*cos(e4)*cos(e5)^2*cos(e6)*sin(e2)*sin(e4)*sin(e6) + 2*I6xy*de3*cos(e2)*cos(e4)*cos(e5)^2*cos(e6)*sin(e3)*sin(e4)*sin(e6) + 2*I6xy*de3*cos(e3)*cos(e4)*cos(e5)^2*cos(e6)*sin(e2)*sin(e4)*sin(e6) + 8*I6yz*de1*cos(e2)*cos(e3)*cos(e4)*cos(e5)^2*sin(e2)*sin(e3)*sin(e6) + 4*I6yz*de1*cos(e2)*cos(e3)^2*cos(e4)*cos(e6)*sin(e2)*sin(e4)*sin(e5) + 4*I6yz*de1*cos(e2)^2*cos(e3)*cos(e4)*cos(e6)*sin(e3)*sin(e4)*sin(e5) + d4*de2*m6*y6*cos(e2)*cos(e3)*cos(e5)*sin(e4)*sin(e6) + d4*de3*m6*y6*cos(e2)*cos(e3)*cos(e5)*sin(e4)*sin(e6) + 2*de4*m6*x6*y6*cos(e2)*cos(e3)*cos(e4)*cos(e5)*sin(e4) + 2*de6*m6*x6*y6*cos(e2)*cos(e3)*cos(e5)*cos(e6)*sin(e6) + 2*de4*m5*x5*z5*cos(e2)*cos(e3)*cos(e4)*cos(e5)*sin(e4) - de2*m6*x6*z6*cos(e2)*cos(e3)*cos(e4)*cos(e5)*sin(e6) - de3*m6*x6*z6*cos(e2)*cos(e3)*cos(e4)*cos(e5)*sin(e6) + de5*m6*x6*z6*cos(e2)*cos(e3)*cos(e4)*cos(e6)*sin(e4) + 2*de4*m6*x6*z6*cos(e2)*cos(e3)*cos(e5)*cos(e6)*sin(e5) - 4*a3*de1*m5*x5*cos(e2)*cos(e3)*sin(e2)*sin(e3)*sin(e5) - 2*a2*de1*m6*x6*cos(e2)*cos(e3)*sin(e2)*sin(e4)*sin(e6) - 2*a2*de1*m6*x6*cos(e2)*cos(e6)*sin(e2)*sin(e3)*sin(e5) + a1*de1*m6*y6*cos(e4)*cos(e5)*sin(e2)*sin(e3)*sin(e6) + a3*de2*m6*y6*cos(e2)*cos(e5)*sin(e3)*sin(e4)*sin(e6) + a3*de2*m6*y6*cos(e3)*cos(e5)*sin(e2)*sin(e4)*sin(e6) + a3*de3*m6*y6*cos(e2)*cos(e5)*sin(e3)*sin(e4)*sin(e6) + a3*de3*m6*y6*cos(e3)*cos(e5)*sin(e2)*sin(e4)*sin(e6) + d4*de2*m6*x6*cos(e5)*cos(e6)*sin(e2)*sin(e3)*sin(e4) + d4*de3*m6*x6*cos(e5)*cos(e6)*sin(e2)*sin(e3)*sin(e4) + 8*I6xy*de1*cos(e2)*cos(e3)*cos(e6)^2*sin(e2)*sin(e3)*sin(e4)*sin(e5) - I6xx*de5*cos(e4)*cos(e5)*cos(e6)^2*sin(e2)*sin(e3)*sin(e4)*sin(e5) - I6xx*de6*cos(e4)*cos(e5)^2*cos(e6)*sin(e2)*sin(e3)*sin(e4)*sin(e6) + I6yy*de5*cos(e4)*cos(e5)*cos(e6)^2*sin(e2)*sin(e3)*sin(e4)*sin(e5) + I6yy*de6*cos(e4)*cos(e5)^2*cos(e6)*sin(e2)*sin(e3)*sin(e4)*sin(e6) + 4*I6zx*de1*cos(e2)*cos(e3)^2*cos(e4)*sin(e2)*sin(e4)*sin(e5)*sin(e6) + 4*I6zx*de1*cos(e2)^2*cos(e3)*cos(e4)*sin(e3)*sin(e4)*sin(e5)*sin(e6) + 4*d4*de1*m4*y4*cos(e2)*cos(e3)*sin(e2)*sin(e3)*sin(e4) - 4*d4*de1*m5*z5*cos(e2)*cos(e3)*sin(e2)*sin(e3)*sin(e4) + 8*de1*m6*x6*z6*cos(e2)^2*cos(e3)^2*cos(e4)*cos(e5)^2*cos(e6) + 4*de1*m5*x5*y5*cos(e2)*cos(e3)*cos(e4)*sin(e2)*sin(e3) - 2*de1*m6*x6*y6*cos(e2)*cos(e4)*cos(e5)*sin(e2)*sin(e4) - 2*de1*m6*x6*y6*cos(e3)*cos(e4)*cos(e5)*sin(e3)*sin(e4) - 2*de1*m6*x6*y6*cos(e4)*cos(e5)*cos(e6)*sin(e5)*sin(e6) - 4*de1*m4*x4*z4*cos(e2)*cos(e3)*cos(e4)*sin(e2)*sin(e3) - 2*de1*m5*x5*z5*cos(e2)*cos(e4)*cos(e5)*sin(e2)*sin(e4) - 2*de1*m5*x5*z5*cos(e3)*cos(e4)*cos(e5)*sin(e3)*sin(e4) + 2*de1*m6*x6*z6*cos(e2)*cos(e5)*cos(e6)*sin(e2)*sin(e5) + 2*de1*m6*x6*z6*cos(e3)*cos(e5)*cos(e6)*sin(e3)*sin(e5) - 2*de4*m5*y5*z5*cos(e2)*cos(e3)*cos(e4)*sin(e4)*sin(e5) + de2*m6*y6*z6*cos(e4)*cos(e5)*cos(e6)*sin(e2)*sin(e3) + de3*m6*y6*z6*cos(e4)*cos(e5)*cos(e6)*sin(e2)*sin(e3) - de5*m6*y6*z6*cos(e2)*cos(e3)*cos(e4)*sin(e4)*sin(e6) - 2*de4*m6*y6*z6*cos(e2)*cos(e3)*cos(e5)*sin(e5)*sin(e6) + de5*m6*y6*z6*cos(e2)*cos(e4)*cos(e6)*sin(e3)*sin(e5) + de5*m6*y6*z6*cos(e3)*cos(e4)*cos(e6)*sin(e2)*sin(e5) + 2*a2*de1*m6*y6*cos(e2)*sin(e2)*sin(e3)*sin(e5)*sin(e6) - d4*de2*m6*y6*cos(e5)*sin(e2)*sin(e3)*sin(e4)*sin(e6) - d4*de3*m6*y6*cos(e5)*sin(e2)*sin(e3)*sin(e4)*sin(e6) - de2*m6*x6^2*cos(e2)*cos(e3)*cos(e5)*cos(e6)^2*sin(e4)*sin(e5) - 2*de2*m6*x6^2*cos(e2)*cos(e4)^2*cos(e5)*cos(e6)*sin(e3)*sin(e6) - 2*de2*m6*x6^2*cos(e3)*cos(e4)^2*cos(e5)*cos(e6)*sin(e2)*sin(e6) - de3*m6*x6^2*cos(e2)*cos(e3)*cos(e5)*cos(e6)^2*sin(e4)*sin(e5) - 2*de3*m6*x6^2*cos(e2)*cos(e4)^2*cos(e5)*cos(e6)*sin(e3)*sin(e6) - 2*de3*m6*x6^2*cos(e3)*cos(e4)^2*cos(e5)*cos(e6)*sin(e2)*sin(e6) - de5*m6*x6^2*cos(e2)*cos(e3)*cos(e4)^2*cos(e6)*sin(e5)*sin(e6) + de2*m6*y6^2*cos(e2)*cos(e3)*cos(e5)*cos(e6)^2*sin(e4)*sin(e5) + 2*de2*m6*y6^2*cos(e2)*cos(e4)^2*cos(e5)*cos(e6)*sin(e3)*sin(e6) + 2*de2*m6*y6^2*cos(e3)*cos(e4)^2*cos(e5)*cos(e6)*sin(e2)*sin(e6) + de3*m6*y6^2*cos(e2)*cos(e3)*cos(e5)*cos(e6)^2*sin(e4)*sin(e5) + 2*de3*m6*y6^2*cos(e2)*cos(e4)^2*cos(e5)*cos(e6)*sin(e3)*sin(e6) + 2*de3*m6*y6^2*cos(e3)*cos(e4)^2*cos(e5)*cos(e6)*sin(e2)*sin(e6) + de5*m6*y6^2*cos(e2)*cos(e3)*cos(e4)^2*cos(e6)*sin(e5)*sin(e6) + 2*de5*m5*x5*y5*cos(e2)*cos(e5)*sin(e3)*sin(e4)*sin(e5) + 2*de5*m5*x5*y5*cos(e3)*cos(e5)*sin(e2)*sin(e4)*sin(e5) - 2*de4*m6*x6*y6*cos(e4)*cos(e5)*sin(e2)*sin(e3)*sin(e4) - de6*m6*x6*y6*cos(e2)*cos(e5)*sin(e3)*sin(e4)*sin(e5) - de6*m6*x6*y6*cos(e3)*cos(e5)*sin(e2)*sin(e4)*sin(e5) - 2*de6*m6*x6*y6*cos(e5)*cos(e6)*sin(e2)*sin(e3)*sin(e6) - 8*de1*m6*y6*z6*cos(e2)^2*cos(e3)^2*cos(e4)*cos(e5)^2*sin(e6) - 2*de4*m5*x5*z5*cos(e4)*cos(e5)*sin(e2)*sin(e3)*sin(e4) + de2*m6*x6*z6*cos(e4)*cos(e5)*sin(e2)*sin(e3)*sin(e6) + de3*m6*x6*z6*cos(e4)*cos(e5)*sin(e2)*sin(e3)*sin(e6) - de5*m6*x6*z6*cos(e4)*cos(e6)*sin(e2)*sin(e3)*sin(e4) - 2*de4*m6*x6*z6*cos(e5)*cos(e6)*sin(e2)*sin(e3)*sin(e5) + de5*m6*x6*z6*cos(e2)*cos(e4)*sin(e3)*sin(e5)*sin(e6) + de5*m6*x6*z6*cos(e3)*cos(e4)*sin(e2)*sin(e5)*sin(e6) + 4*de1*m4*y4*z4*cos(e2)*cos(e3)*sin(e2)*sin(e3)*sin(e4) + 2*de1*m5*y5*z5*cos(e2)*cos(e4)*sin(e2)*sin(e4)*sin(e5) + 2*de1*m5*y5*z5*cos(e3)*cos(e4)*sin(e3)*sin(e4)*sin(e5) - 2*de1*m6*y6*z6*cos(e2)*cos(e5)*sin(e2)*sin(e5)*sin(e6) - 2*de1*m6*y6*z6*cos(e3)*cos(e5)*sin(e3)*sin(e5)*sin(e6) + 2*de1*m6*x6^2*cos(e2)*cos(e3)^2*cos(e4)^2*cos(e5)^2*cos(e6)^2*sin(e2) + 2*de1*m6*x6^2*cos(e2)^2*cos(e3)*cos(e4)^2*cos(e5)^2*cos(e6)^2*sin(e3) - 2*de1*m6*y6^2*cos(e2)*cos(e3)^2*cos(e4)^2*cos(e5)^2*cos(e6)^2*sin(e2) - 2*de1*m6*y6^2*cos(e2)^2*cos(e3)*cos(e4)^2*cos(e5)^2*cos(e6)^2*sin(e3) - 8*de1*m6*x6*y6*cos(e2)^2*cos(e3)^2*cos(e6)^2*sin(e4)*sin(e5) + 2*de4*m5*y5*z5*cos(e4)*sin(e2)*sin(e3)*sin(e4)*sin(e5) + de5*m6*y6*z6*cos(e4)*sin(e2)*sin(e3)*sin(e4)*sin(e6) + 2*de4*m6*y6*z6*cos(e5)*sin(e2)*sin(e3)*sin(e5)*sin(e6) + de2*m6*x6^2*cos(e5)*cos(e6)^2*sin(e2)*sin(e3)*sin(e4)*sin(e5) + de3*m6*x6^2*cos(e5)*cos(e6)^2*sin(e2)*sin(e3)*sin(e4)*sin(e5) + de5*m6*x6^2*cos(e4)^2*cos(e6)*sin(e2)*sin(e3)*sin(e5)*sin(e6) - de2*m6*y6^2*cos(e5)*cos(e6)^2*sin(e2)*sin(e3)*sin(e4)*sin(e5) - de3*m6*y6^2*cos(e5)*cos(e6)^2*sin(e2)*sin(e3)*sin(e4)*sin(e5) - de5*m6*y6^2*cos(e4)^2*cos(e6)*sin(e2)*sin(e3)*sin(e5)*sin(e6) + 4*a3*de1*m5*x5*cos(e2)*cos(e3)^2*cos(e4)*cos(e5)*sin(e2) + 4*a3*de1*m5*x5*cos(e2)^2*cos(e3)*cos(e4)*cos(e5)*sin(e3) + 2*a2*de1*m6*x6*cos(e2)^2*cos(e4)*cos(e5)*cos(e6)*sin(e3) - 8*I6xy*de1*cos(e2)*cos(e3)^2*cos(e4)*cos(e5)*cos(e6)^2*sin(e2)*sin(e4) - 8*I6xy*de1*cos(e2)^2*cos(e3)*cos(e4)*cos(e5)*cos(e6)^2*sin(e3)*sin(e4) - 8*I6xy*de1*cos(e2)^2*cos(e3)^2*cos(e4)*cos(e5)*cos(e6)*sin(e5)*sin(e6) - 4*I6zx*de1*cos(e2)*cos(e3)^2*cos(e4)^2*cos(e5)*cos(e6)*sin(e2)*sin(e5) - 4*I6zx*de1*cos(e2)^2*cos(e3)*cos(e4)^2*cos(e5)*cos(e6)*sin(e3)*sin(e5) - de5*m6*y6*z6*cos(e2)*cos(e3)*cos(e4)^2*cos(e5)*cos(e6) - 4*a3*de1*m5*y5*cos(e2)*cos(e3)^2*cos(e4)*sin(e2)*sin(e5) - 4*a3*de1*m5*y5*cos(e2)^2*cos(e3)*cos(e4)*sin(e3)*sin(e5) - 4*a3*de1*m6*y6*cos(e2)*cos(e3)^2*cos(e6)*sin(e2)*sin(e4) - 4*a3*de1*m6*y6*cos(e2)^2*cos(e3)*cos(e6)*sin(e3)*sin(e4) - 2*a2*de1*m6*y6*cos(e2)^2*cos(e4)*cos(e5)*sin(e3)*sin(e6) - 4*a3*de1*m6*z6*cos(e2)*cos(e3)^2*cos(e4)*sin(e2)*sin(e5) - 4*a3*de1*m6*z6*cos(e2)^2*cos(e3)*cos(e4)*sin(e3)*sin(e5) - 4*d4*de1*m6*x6*cos(e2)*cos(e3)^2*cos(e6)*sin(e2)*sin(e5) - 4*d4*de1*m6*x6*cos(e2)^2*cos(e3)*cos(e6)*sin(e3)*sin(e5) + 4*I6yz*de1*cos(e2)*cos(e3)^2*cos(e4)^2*cos(e5)*sin(e2)*sin(e5)*sin(e6) + 4*I6yz*de1*cos(e2)^2*cos(e3)*cos(e4)^2*cos(e5)*sin(e3)*sin(e5)*sin(e6) - 2*de4*m5*x5*y5*cos(e2)*cos(e3)*cos(e4)^2*cos(e5)*sin(e5) - 2*de5*m5*x5*y5*cos(e2)*cos(e3)*cos(e4)*cos(e5)^2*sin(e4) - 2*de2*m6*x6*y6*cos(e2)*cos(e3)*cos(e4)*cos(e6)^2*sin(e5) - 2*de3*m6*x6*y6*cos(e2)*cos(e3)*cos(e4)*cos(e6)^2*sin(e5) + de6*m6*x6*y6*cos(e2)*cos(e3)*cos(e4)*cos(e5)^2*sin(e4) - 2*de4*m6*x6*y6*cos(e2)*cos(e3)*cos(e4)^2*cos(e6)*sin(e6) - 2*de5*m6*x6*y6*cos(e2)*cos(e4)*cos(e5)*cos(e6)^2*sin(e3) - 2*de5*m6*x6*y6*cos(e3)*cos(e4)*cos(e5)*cos(e6)^2*sin(e2) - 2*de6*m6*x6*y6*cos(e2)*cos(e3)*cos(e4)*cos(e6)^2*sin(e4) + 2*de4*m6*x6*y6*cos(e2)*cos(e3)*cos(e5)^2*cos(e6)*sin(e6) - 2*de2*m6*x6*z6*cos(e2)*cos(e3)*cos(e5)^2*cos(e6)*sin(e4) - 2*de3*m6*x6*z6*cos(e2)*cos(e3)*cos(e5)^2*cos(e6)*sin(e4) - de5*m6*x6*z6*cos(e2)*cos(e3)*cos(e4)^2*cos(e5)*sin(e6) - de6*m6*x6*z6*cos(e2)*cos(e3)*cos(e4)^2*cos(e6)*sin(e5) - 4*a3*de1*m6*x6*cos(e2)*cos(e3)^2*sin(e2)*sin(e4)*sin(e6) - 4*a3*de1*m6*x6*cos(e2)^2*cos(e3)*sin(e3)*sin(e4)*sin(e6) + 4*d4*de1*m6*y6*cos(e2)*cos(e3)^2*sin(e2)*sin(e5)*sin(e6) + 4*d4*de1*m6*y6*cos(e2)^2*cos(e3)*sin(e3)*sin(e5)*sin(e6) - 4*de1*m4*x4*y4*cos(e2)*cos(e3)^2*cos(e4)*sin(e2)*sin(e4) - 4*de1*m4*x4*y4*cos(e2)^2*cos(e3)*cos(e4)*sin(e3)*sin(e4) - 4*de1*m5*x5*y5*cos(e2)*cos(e3)^2*cos(e5)*sin(e2)*sin(e5) + 2*de1*m5*x5*y5*cos(e2)*cos(e4)^2*cos(e5)*sin(e2)*sin(e5) - 4*de1*m5*x5*y5*cos(e2)^2*cos(e3)*cos(e5)*sin(e3)*sin(e5) + 2*de1*m5*x5*y5*cos(e3)*cos(e4)^2*cos(e5)*sin(e3)*sin(e5) + 8*de1*m6*x6*y6*cos(e2)*cos(e3)^2*cos(e6)*sin(e2)*sin(e6) + 2*de1*m6*x6*y6*cos(e2)*cos(e4)^2*cos(e6)*sin(e2)*sin(e6) + 8*de1*m6*x6*y6*cos(e2)^2*cos(e3)*cos(e6)*sin(e3)*sin(e6) + 2*de1*m6*x6*y6*cos(e2)*cos(e5)^2*cos(e6)*sin(e2)*sin(e6) + 2*de1*m6*x6*y6*cos(e3)*cos(e4)^2*cos(e6)*sin(e3)*sin(e6) + 2*de1*m6*x6*y6*cos(e3)*cos(e5)^2*cos(e6)*sin(e3)*sin(e6) + 2*de2*m6*y6*z6*cos(e2)*cos(e3)*cos(e5)^2*sin(e4)*sin(e6) + 2*de2*m6*y6*z6*cos(e2)*cos(e4)^2*cos(e6)*sin(e3)*sin(e5) + 2*de2*m6*y6*z6*cos(e3)*cos(e4)^2*cos(e6)*sin(e2)*sin(e5) + 2*de3*m6*y6*z6*cos(e2)*cos(e3)*cos(e5)^2*sin(e4)*sin(e6) + 2*de3*m6*y6*z6*cos(e2)*cos(e4)^2*cos(e6)*sin(e3)*sin(e5) + 2*de3*m6*y6*z6*cos(e3)*cos(e4)^2*cos(e6)*sin(e2)*sin(e5) + de5*m6*y6*z6*cos(e4)^2*cos(e5)*cos(e6)*sin(e2)*sin(e3) + de6*m6*y6*z6*cos(e2)*cos(e3)*cos(e4)^2*sin(e5)*sin(e6) + de6*m6*y6*z6*cos(e2)*cos(e5)^2*cos(e6)*sin(e3)*sin(e4) + de6*m6*y6*z6*cos(e3)*cos(e5)^2*cos(e6)*sin(e2)*sin(e4) - de2*m6*x6^2*cos(e2)*cos(e4)*cos(e5)^2*cos(e6)^2*sin(e3)*sin(e4) - de2*m6*x6^2*cos(e3)*cos(e4)*cos(e5)^2*cos(e6)^2*sin(e2)*sin(e4) - de3*m6*x6^2*cos(e2)*cos(e4)*cos(e5)^2*cos(e6)^2*sin(e3)*sin(e4) - de3*m6*x6^2*cos(e3)*cos(e4)*cos(e5)^2*cos(e6)^2*sin(e2)*sin(e4) + de2*m6*y6^2*cos(e2)*cos(e4)*cos(e5)^2*cos(e6)^2*sin(e3)*sin(e4) + de2*m6*y6^2*cos(e3)*cos(e4)*cos(e5)^2*cos(e6)^2*sin(e2)*sin(e4) + de3*m6*y6^2*cos(e2)*cos(e4)*cos(e5)^2*cos(e6)^2*sin(e3)*sin(e4) + de3*m6*y6^2*cos(e3)*cos(e4)*cos(e5)^2*cos(e6)^2*sin(e2)*sin(e4) + 2*de4*m5*x5*y5*cos(e4)^2*cos(e5)*sin(e2)*sin(e3)*sin(e5) + 2*de5*m5*x5*y5*cos(e4)*cos(e5)^2*sin(e2)*sin(e3)*sin(e4) + 2*de2*m6*x6*y6*cos(e4)*cos(e6)^2*sin(e2)*sin(e3)*sin(e5) + 2*de3*m6*x6*y6*cos(e4)*cos(e6)^2*sin(e2)*sin(e3)*sin(e5) - de6*m6*x6*y6*cos(e4)*cos(e5)^2*sin(e2)*sin(e3)*sin(e4) + 2*de4*m6*x6*y6*cos(e4)^2*cos(e6)*sin(e2)*sin(e3)*sin(e6) + 2*de6*m6*x6*y6*cos(e4)*cos(e6)^2*sin(e2)*sin(e3)*sin(e4) - 2*de4*m6*x6*y6*cos(e5)^2*cos(e6)*sin(e2)*sin(e3)*sin(e6) + 2*de2*m6*x6*z6*cos(e2)*cos(e4)^2*sin(e3)*sin(e5)*sin(e6) + 2*de2*m6*x6*z6*cos(e3)*cos(e4)^2*sin(e2)*sin(e5)*sin(e6) + 2*de2*m6*x6*z6*cos(e5)^2*cos(e6)*sin(e2)*sin(e3)*sin(e4) + 2*de3*m6*x6*z6*cos(e2)*cos(e4)^2*sin(e3)*sin(e5)*sin(e6) + 2*de3*m6*x6*z6*cos(e3)*cos(e4)^2*sin(e2)*sin(e5)*sin(e6) + 2*de3*m6*x6*z6*cos(e5)^2*cos(e6)*sin(e2)*sin(e3)*sin(e4) + de5*m6*x6*z6*cos(e4)^2*cos(e5)*sin(e2)*sin(e3)*sin(e6) + de6*m6*x6*z6*cos(e2)*cos(e5)^2*sin(e3)*sin(e4)*sin(e6) + de6*m6*x6*z6*cos(e3)*cos(e5)^2*sin(e2)*sin(e4)*sin(e6) + de6*m6*x6*z6*cos(e4)^2*cos(e6)*sin(e2)*sin(e3)*sin(e5) + 2*I6xx*de4*cos(e2)*cos(e3)*cos(e4)*cos(e5)*cos(e6)*sin(e4)*sin(e6) - 2*I6yy*de4*cos(e2)*cos(e3)*cos(e4)*cos(e5)*cos(e6)*sin(e4)*sin(e6) + I6yz*de6*cos(e2)*cos(e3)*cos(e4)*cos(e5)*cos(e6)*sin(e4)*sin(e5) - 4*de1*m6*x6^2*cos(e2)^2*cos(e3)^2*cos(e6)*sin(e4)*sin(e5)*sin(e6) + 4*de1*m6*y6^2*cos(e2)^2*cos(e3)^2*cos(e6)*sin(e4)*sin(e5)*sin(e6) - 2*de2*m6*y6*z6*cos(e5)^2*sin(e2)*sin(e3)*sin(e4)*sin(e6) - 2*de3*m6*y6*z6*cos(e5)^2*sin(e2)*sin(e3)*sin(e4)*sin(e6) - de6*m6*y6*z6*cos(e4)^2*sin(e2)*sin(e3)*sin(e5)*sin(e6) + 4*d4*de1*m6*x6*cos(e2)^2*cos(e3)^2*cos(e4)*cos(e5)*cos(e6) + 4*I5xx*de1*cos(e2)*cos(e3)*cos(e4)*cos(e5)*sin(e2)*sin(e3)*sin(e5) - 2*I6xx*de1*cos(e2)*cos(e4)*cos(e5)*cos(e6)*sin(e2)*sin(e4)*sin(e6) - 2*I6xx*de1*cos(e3)*cos(e4)*cos(e5)*cos(e6)*sin(e3)*sin(e4)*sin(e6) + 2*I6xy*de2*cos(e2)*cos(e3)*cos(e5)*cos(e6)*sin(e4)*sin(e5)*sin(e6) + 2*I6xy*de3*cos(e2)*cos(e3)*cos(e5)*cos(e6)*sin(e4)*sin(e5)*sin(e6) - 4*I5yy*de1*cos(e2)*cos(e3)*cos(e4)*cos(e5)*sin(e2)*sin(e3)*sin(e5) + 4*I6yy*de1*cos(e2)*cos(e3)*cos(e4)*cos(e5)*sin(e2)*sin(e3)*sin(e5) + 4*I6yz*de1*cos(e2)*cos(e3)*cos(e5)*cos(e6)*sin(e2)*sin(e3)*sin(e4) + 2*I6yy*de1*cos(e2)*cos(e4)*cos(e5)*cos(e6)*sin(e2)*sin(e4)*sin(e6) + 2*I6yy*de1*cos(e3)*cos(e4)*cos(e5)*cos(e6)*sin(e3)*sin(e4)*sin(e6) - 4*I6zz*de1*cos(e2)*cos(e3)*cos(e4)*cos(e5)*sin(e2)*sin(e3)*sin(e5) + 2*I6zx*de2*cos(e2)*cos(e4)*cos(e5)*cos(e6)*sin(e3)*sin(e4)*sin(e5) + 2*I6zx*de2*cos(e3)*cos(e4)*cos(e5)*cos(e6)*sin(e2)*sin(e4)*sin(e5) + 2*I6zx*de3*cos(e2)*cos(e4)*cos(e5)*cos(e6)*sin(e3)*sin(e4)*sin(e5) + 2*I6zx*de3*cos(e3)*cos(e4)*cos(e5)*cos(e6)*sin(e2)*sin(e4)*sin(e5) + I6zx*de6*cos(e2)*cos(e3)*cos(e4)*cos(e5)*sin(e4)*sin(e5)*sin(e6) - 4*I6xy*de1*cos(e2)*cos(e3)^2*cos(e4)^2*cos(e5)^2*cos(e6)*sin(e2)*sin(e6) - 4*I6xy*de1*cos(e2)^2*cos(e3)*cos(e4)^2*cos(e5)^2*cos(e6)*sin(e3)*sin(e6) - 4*d4*de1*m6*y6*cos(e2)^2*cos(e3)^2*cos(e4)*cos(e5)*sin(e6) - 2*I6xx*de4*cos(e4)*cos(e5)*cos(e6)*sin(e2)*sin(e3)*sin(e4)*sin(e6) - I6xx*de6*cos(e2)*cos(e5)*cos(e6)*sin(e3)*sin(e4)*sin(e5)*sin(e6) - I6xx*de6*cos(e3)*cos(e5)*cos(e6)*sin(e2)*sin(e4)*sin(e5)*sin(e6) - 2*I6yz*de2*cos(e2)*cos(e4)*cos(e5)*sin(e3)*sin(e4)*sin(e5)*sin(e6) - 2*I6yz*de2*cos(e3)*cos(e4)*cos(e5)*sin(e2)*sin(e4)*sin(e5)*sin(e6) - 2*I6yz*de3*cos(e2)*cos(e4)*cos(e5)*sin(e3)*sin(e4)*sin(e5)*sin(e6) - 2*I6yz*de3*cos(e3)*cos(e4)*cos(e5)*sin(e2)*sin(e4)*sin(e5)*sin(e6) + 2*I6yy*de4*cos(e4)*cos(e5)*cos(e6)*sin(e2)*sin(e3)*sin(e4)*sin(e6) - I6yz*de6*cos(e4)*cos(e5)*cos(e6)*sin(e2)*sin(e3)*sin(e4)*sin(e5) + I6yy*de6*cos(e2)*cos(e5)*cos(e6)*sin(e3)*sin(e4)*sin(e5)*sin(e6) + I6yy*de6*cos(e3)*cos(e5)*cos(e6)*sin(e2)*sin(e4)*sin(e5)*sin(e6) + 4*I6zx*de1*cos(e2)*cos(e3)*cos(e5)*sin(e2)*sin(e3)*sin(e4)*sin(e6) - 2*I6xy*de2*cos(e5)*cos(e6)*sin(e2)*sin(e3)*sin(e4)*sin(e5)*sin(e6) - 2*I6xy*de3*cos(e5)*cos(e6)*sin(e2)*sin(e3)*sin(e4)*sin(e5)*sin(e6) - I6zx*de6*cos(e4)*cos(e5)*sin(e2)*sin(e3)*sin(e4)*sin(e5)*sin(e6) - de5*m5*x5^2*cos(e2)*cos(e3)*cos(e4)*cos(e5)*sin(e4)*sin(e5) - de2*m6*x6^2*cos(e2)*cos(e3)*cos(e4)*cos(e6)*sin(e5)*sin(e6) - de3*m6*x6^2*cos(e2)*cos(e3)*cos(e4)*cos(e6)*sin(e5)*sin(e6) - de5*m6*x6^2*cos(e2)*cos(e4)*cos(e5)*cos(e6)*sin(e3)*sin(e6) - de5*m6*x6^2*cos(e3)*cos(e4)*cos(e5)*cos(e6)*sin(e2)*sin(e6) - de6*m6*x6^2*cos(e2)*cos(e3)*cos(e4)*cos(e6)*sin(e4)*sin(e6) - 4*de2*m6*x6*y6*cos(e2)*cos(e4)^2*cos(e5)*cos(e6)^2*sin(e3) - 4*de2*m6*x6*y6*cos(e3)*cos(e4)^2*cos(e5)*cos(e6)^2*sin(e2) - 4*de3*m6*x6*y6*cos(e2)*cos(e4)^2*cos(e5)*cos(e6)^2*sin(e3) - 4*de3*m6*x6*y6*cos(e3)*cos(e4)^2*cos(e5)*cos(e6)^2*sin(e2) - 2*de5*m6*x6*y6*cos(e2)*cos(e3)*cos(e4)^2*cos(e6)^2*sin(e5) + de5*m5*y5^2*cos(e2)*cos(e3)*cos(e4)*cos(e5)*sin(e4)*sin(e5) + de2*m6*y6^2*cos(e2)*cos(e3)*cos(e4)*cos(e6)*sin(e5)*sin(e6) - de5*m6*y6^2*cos(e2)*cos(e3)*cos(e4)*cos(e5)*sin(e4)*sin(e5) + de3*m6*y6^2*cos(e2)*cos(e3)*cos(e4)*cos(e6)*sin(e5)*sin(e6) + de5*m6*y6^2*cos(e2)*cos(e4)*cos(e5)*cos(e6)*sin(e3)*sin(e6) + de5*m6*y6^2*cos(e3)*cos(e4)*cos(e5)*cos(e6)*sin(e2)*sin(e6) + de6*m6*y6^2*cos(e2)*cos(e3)*cos(e4)*cos(e6)*sin(e4)*sin(e6) + de5*m6*z6^2*cos(e2)*cos(e3)*cos(e4)*cos(e5)*sin(e4)*sin(e5) - 4*de1*m6*y6*z6*cos(e2)^2*cos(e3)^2*cos(e5)*cos(e6)*sin(e4) + 4*de1*m6*x6^2*cos(e2)^2*cos(e3)^2*cos(e4)*cos(e5)*cos(e6)^2*sin(e5) - 4*de1*m6*y6^2*cos(e2)^2*cos(e3)^2*cos(e4)*cos(e5)*cos(e6)^2*sin(e5) - 4*de1*m6*x6*z6*cos(e2)^2*cos(e3)^2*cos(e5)*sin(e4)*sin(e6) + a1*de1*m6*x6*cos(e2)*cos(e3)*cos(e4)*cos(e5)*cos(e6) + de5*m5*x5^2*cos(e4)*cos(e5)*sin(e2)*sin(e3)*sin(e4)*sin(e5) + de2*m6*x6^2*cos(e4)*cos(e6)*sin(e2)*sin(e3)*sin(e5)*sin(e6) + de3*m6*x6^2*cos(e4)*cos(e6)*sin(e2)*sin(e3)*sin(e5)*sin(e6) + de6*m6*x6^2*cos(e4)*cos(e6)*sin(e2)*sin(e3)*sin(e4)*sin(e6) + 2*de5*m6*x6*y6*cos(e4)^2*cos(e6)^2*sin(e2)*sin(e3)*sin(e5) - de5*m5*y5^2*cos(e4)*cos(e5)*sin(e2)*sin(e3)*sin(e4)*sin(e5) - de2*m6*y6^2*cos(e4)*cos(e6)*sin(e2)*sin(e3)*sin(e5)*sin(e6) + de5*m6*y6^2*cos(e4)*cos(e5)*sin(e2)*sin(e3)*sin(e4)*sin(e5) - de3*m6*y6^2*cos(e4)*cos(e6)*sin(e2)*sin(e3)*sin(e5)*sin(e6) - de6*m6*y6^2*cos(e4)*cos(e6)*sin(e2)*sin(e3)*sin(e4)*sin(e6) - de5*m6*z6^2*cos(e4)*cos(e5)*sin(e2)*sin(e3)*sin(e4)*sin(e5) - de5*m6*x6^2*cos(e2)*cos(e3)*cos(e4)*cos(e5)*cos(e6)^2*sin(e4)*sin(e5) - de6*m6*x6^2*cos(e2)*cos(e3)*cos(e4)*cos(e5)^2*cos(e6)*sin(e4)*sin(e6) + de5*m6*y6^2*cos(e2)*cos(e3)*cos(e4)*cos(e5)*cos(e6)^2*sin(e4)*sin(e5) + de6*m6*y6^2*cos(e2)*cos(e3)*cos(e4)*cos(e5)^2*cos(e6)*sin(e4)*sin(e6) + 2*de2*m5*x5*y5*cos(e2)*cos(e4)*cos(e5)*sin(e3)*sin(e4)*sin(e5) + 2*de2*m5*x5*y5*cos(e3)*cos(e4)*cos(e5)*sin(e2)*sin(e4)*sin(e5) + 2*de3*m5*x5*y5*cos(e2)*cos(e4)*cos(e5)*sin(e3)*sin(e4)*sin(e5) + 2*de3*m5*x5*y5*cos(e3)*cos(e4)*cos(e5)*sin(e2)*sin(e4)*sin(e5) + 2*de2*m6*x6*y6*cos(e2)*cos(e4)*cos(e6)*sin(e3)*sin(e4)*sin(e6) + 2*de2*m6*x6*y6*cos(e3)*cos(e4)*cos(e6)*sin(e2)*sin(e4)*sin(e6) + 2*de3*m6*x6*y6*cos(e2)*cos(e4)*cos(e6)*sin(e3)*sin(e4)*sin(e6) + 2*de3*m6*x6*y6*cos(e3)*cos(e4)*cos(e6)*sin(e2)*sin(e4)*sin(e6) + 2*de6*m6*x6*y6*cos(e2)*cos(e4)*cos(e6)*sin(e3)*sin(e5)*sin(e6) + 2*de6*m6*x6*y6*cos(e3)*cos(e4)*cos(e6)*sin(e2)*sin(e5)*sin(e6) + 2*de4*m6*x6*z6*cos(e2)*cos(e3)*cos(e4)*sin(e4)*sin(e5)*sin(e6) + 2*de5*m6*x6*z6*cos(e2)*cos(e5)*cos(e6)*sin(e3)*sin(e4)*sin(e5) + 2*de5*m6*x6*z6*cos(e3)*cos(e5)*cos(e6)*sin(e2)*sin(e4)*sin(e5) - 4*de1*m5*y5*z5*cos(e2)*cos(e3)*cos(e5)*sin(e2)*sin(e3)*sin(e4) - 4*de1*m6*y6*z6*cos(e2)*cos(e3)*cos(e4)*sin(e2)*sin(e3)*sin(e6) - 2*de1*m6*y6*z6*cos(e2)*cos(e4)*cos(e6)*sin(e2)*sin(e4)*sin(e5) - 2*de1*m6*y6*z6*cos(e3)*cos(e4)*cos(e6)*sin(e3)*sin(e4)*sin(e5) - 4*de1*m6*x6*y6*cos(e2)*cos(e3)*sin(e2)*sin(e3)*sin(e4)*sin(e5) - 4*de1*m5*x5*z5*cos(e2)*cos(e3)*sin(e2)*sin(e3)*sin(e4)*sin(e5) - 2*de1*m6*x6*z6*cos(e2)*cos(e4)*sin(e2)*sin(e4)*sin(e5)*sin(e6) - 2*de1*m6*x6*z6*cos(e3)*cos(e4)*sin(e3)*sin(e4)*sin(e5)*sin(e6) - 2*de4*m6*y6*z6*cos(e4)*cos(e6)*sin(e2)*sin(e3)*sin(e4)*sin(e5) - 2*de5*m6*y6*z6*cos(e2)*cos(e5)*sin(e3)*sin(e4)*sin(e5)*sin(e6) - 2*de5*m6*y6*z6*cos(e3)*cos(e5)*sin(e2)*sin(e4)*sin(e5)*sin(e6) + de5*m6*x6^2*cos(e4)*cos(e5)*cos(e6)^2*sin(e2)*sin(e3)*sin(e4)*sin(e5) + de6*m6*x6^2*cos(e4)*cos(e5)^2*cos(e6)*sin(e2)*sin(e3)*sin(e4)*sin(e6) - de5*m6*y6^2*cos(e4)*cos(e5)*cos(e6)^2*sin(e2)*sin(e3)*sin(e4)*sin(e5) - de6*m6*y6^2*cos(e4)*cos(e5)^2*cos(e6)*sin(e2)*sin(e3)*sin(e4)*sin(e6) - 2*de4*m6*x6*z6*cos(e4)*sin(e2)*sin(e3)*sin(e4)*sin(e5)*sin(e6) + 4*a3*de1*m6*x6*cos(e2)*cos(e3)^2*cos(e4)*cos(e5)*cos(e6)*sin(e2) + 4*a3*de1*m6*x6*cos(e2)^2*cos(e3)*cos(e4)*cos(e5)*cos(e6)*sin(e3) - 4*a3*de1*m6*y6*cos(e2)*cos(e3)^2*cos(e4)*cos(e5)*sin(e2)*sin(e6) - 4*a3*de1*m6*y6*cos(e2)^2*cos(e3)*cos(e4)*cos(e5)*sin(e3)*sin(e6) - 4*de4*m6*x6*y6*cos(e2)*cos(e3)*cos(e4)*cos(e5)*cos(e6)^2*sin(e4) - 4*de6*m6*x6*y6*cos(e2)*cos(e3)*cos(e4)^2*cos(e5)*cos(e6)*sin(e6) - 2*de4*m6*x6*z6*cos(e2)*cos(e3)*cos(e4)^2*cos(e5)*cos(e6)*sin(e5) - 2*de5*m6*x6*z6*cos(e2)*cos(e3)*cos(e4)*cos(e5)^2*cos(e6)*sin(e4) - 8*de1*m5*x5*y5*cos(e2)*cos(e3)*cos(e4)*cos(e5)^2*sin(e2)*sin(e3) + 4*de1*m6*x6*y6*cos(e2)*cos(e3)^2*cos(e4)*cos(e5)*sin(e2)*sin(e4) + 4*de1*m6*x6*y6*cos(e2)^2*cos(e3)*cos(e4)*cos(e5)*sin(e3)*sin(e4) + 4*de1*m6*x6*y6*cos(e2)*cos(e4)*cos(e5)*cos(e6)^2*sin(e2)*sin(e4) + 4*de1*m6*x6*y6*cos(e3)*cos(e4)*cos(e5)*cos(e6)^2*sin(e3)*sin(e4) + 4*de1*m6*x6*y6*cos(e2)^2*cos(e4)*cos(e5)*cos(e6)*sin(e5)*sin(e6) + 4*de1*m6*x6*y6*cos(e3)^2*cos(e4)*cos(e5)*cos(e6)*sin(e5)*sin(e6) + 4*de1*m5*x5*z5*cos(e2)*cos(e3)^2*cos(e4)*cos(e5)*sin(e2)*sin(e4) + 